simulink model "simulator_prototype_v3_pdg"  (R2021b)
settings: Solver=VariableStepAuto  StartTime=0.0  StopTime=60  FixedStep=0.0001  RelTol=1e-4
undefined symbols (not defined in the file or in its folder): X, Y, Z
libraries: sm_lib x47, nesl_utility x7, simulink x1
(part 4 of 13)

== matlab function simulator_prototype_v3_pdg/Dynamic Model/Coriolis_vector1 ==
  data: dq1 input; dq2 input; tau_c output; dq3 input; dq4 input; dq5 input; dq6 input; q1 input; q2 input; q3 input; q4 input; q5 input; q6 input
function tau_c = Coriolis_vector(dq1,dq2,dq3,dq4,dq5,dq6,q1,q2,q3,q4,q5,q6)
%#codegen

%    This function was generated by the Symbolic Math Toolbox version 9.0.
%    08-Oct-2021 19:57:53

t2 = conj(q1);
t3 = conj(q2);
t4 = conj(q3);
t5 = conj(q4);
t6 = conj(q5);
t7 = conj(q6);
t8 = cos(q1);
t9 = cos(q2);
t10 = cos(q4);
t11 = cos(q5);
t12 = cos(q6);
t13 = sin(q1);
t14 = sin(q2);
t15 = sin(q4);
t16 = sin(q5);
t17 = sin(q6);
t23 = q1+q2;
t29 = dq1.^2;
t30 = dq2.^2;
t31 = dq3.^2;
t32 = dq4.^2;
t33 = dq5.^2;
t34 = dq6.^2;
t50 = 9.007199254740992e+15;
t18 = cos(t2);
t19 = cos(t3);
t20 = cos(t5);
t21 = cos(t6);
t22 = cos(t7);
t24 = sin(t2);
t25 = sin(t3);
t26 = sin(t5);
t27 = sin(t6);
t28 = sin(t7);
t35 = cos(t23);
t36 = sin(t23);
t37 = t2+t3;
t51 = t11.*3.347317932164228e+33;
t52 = t16.*3.347317932164228e+33;
t56 = t8.*4.990478e-2;
t58 = t13.*4.990478e-2;
t59 = t8.*2.167433e-2;
t60 = t13.*2.167433e-2;
t61 = t10.*t12.*3.315051378778914e+33;
t62 = t8.*t9.*3.641522e-2;
t63 = t10.*t17.*3.315051378778914e+33;
t64 = t12.*t15.*3.315051378778914e+33;
t65 = t10.*t16.*1.990083581481952e+33;
t66 = t11.*t15.*1.990083581481952e+33;
t67 = t8.*t14.*3.641522e-2;
t68 = t9.*t13.*3.641522e-2;
t69 = t15.*t16.*1.990083581481952e+33;
t70 = t13.*t14.*3.641522e-2;
t74 = t13.*t14.*2.462267e-2;
t78 = t11.*t12.*5.575912001630188e+33;
t79 = t10.*t12.*6.099194893302011e+33;
t80 = t11.*t12.*1.025883768304404e+34;
t81 = t11.*t17.*5.575912001630188e+33;
t82 = t10.*t17.*6.099194893302011e+33;
t83 = t11.*t17.*1.025883768304404e+34;
t84 = t12.*t16.*1.025883768304404e+34;
t85 = t16.*t17.*5.575912001630188e+33;
t87 = t15.*t17.*6.099194893302011e+33;
t89 = t8.*t9.*2.462267e-2;
t90 = t8.*t14.*2.462267e-2;
t91 = t9.*t13.*2.462267e-2;
t93 = t15.*t16.*t17.*3.315051378778914e+33;
t105 = t11.*t15.*t17.*3.315051378778914e+33;
t116 = t11.*t12.*t15.*6.099194893302011e+33;
t118 = t12.*t15.*t16.*6.099194893302011e+33;
t127 = t15.*t16.*t17.*-6.099194893302011e+33;
t142 = t10.*7.746286054220548e+49;
t143 = t15.*7.746286054220548e+49;
t144 = t10.*t16.*1.830618490855195e+48;
t145 = t11.*t15.*1.830618490855195e+48;
t150 = t10.*t11.*1.830618490855195e+48;
t153 = t10.*t11.*7.290917220067534e+49;
t154 = t10.*t16.*7.290917220067534e+49;
t155 = t15.*t16.*7.290917220067534e+49;
t158 = t10.*6.997781708721691e+52;
t159 = t15.*6.997781708721691e+52;
t166 = t10.*t11.*t12.*5.84291401185902e+49;
t168 = t10.*t11.*t17.*5.84291401185902e+49;
t170 = t10.*t16.*t17.*5.84291401185902e+49;
t171 = t11.*t15.*t17.*5.84291401185902e+49;
t174 = t10.*t16.*7.183572847808854e+52;
t175 = t11.*t15.*7.183572847808854e+52;
t177 = t15.*t16.*7.183572847808854e+52;
t178 = t10.*t11.*t12.*1.075008113939401e+50;
t179 = t10.*t11.*t17.*1.075008113939401e+50;
t180 = t10.*t12.*t16.*1.075008113939401e+50;
t181 = t11.*t12.*t15.*1.075008113939401e+50;
t183 = (q3.*t50)./9.007199254740992e+15;
t184 = t10.*t12.*1.196628789628727e+53;
t185 = t10.*t17.*1.196628789628727e+53;
t186 = t12.*t15.*1.196628789628727e+53;
t187 = (t4.*t50)./9.007199254740992e+15;
t191 = t10.*t12.*2.201616617347892e+53;
t192 = t10.*t17.*2.201616617347892e+53;
t193 = q3.*t50.*2.220446049250313e-16i;
t194 = t15.*t17.*2.201616617347892e+53;
t199 = t4.*t50.*2.220446049250313e-16i;
t206 = q3.*t50.*1.110223024625157e-16i;
t210 = t11.*t15.*t17.*1.196628789628727e+53;
t212 = t15.*t16.*t17.*1.196628789628727e+53;
t214 = t4.*t50.*1.110223024625157e-16i;
t219 = t11.*t12.*t15.*2.201616617347892e+53;
t221 = t12.*t15.*t16.*2.201616617347892e+53;
t232 = t10.*t11.*t50.*4.323455642275676e+17i;
t233 = t10.*t16.*t50.*4.323455642275676e+17i;
t234 = t15.*t16.*t50.*4.323455642275676e+17i;
t242 = t15.*t16.*t17.*-2.201616617347892e+53;
t247 = t10.*t12.*t50.*7.201947557068188e+17i;
t248 = t10.*t17.*t50.*1.325049802940888e+18i;
t249 = t12.*t15.*t50.*1.325049802940888e+18i;
t251 = t12.*t15.*t50.*7.201947557068188e+17i;
t253 = t15.*t17.*t50.*1.325049802940888e+18i;
t254 = t15.*t17.*t50.*7.201947557068188e+17i;
t278 = t10.*t11.*t12.*t50.*1.325049802940888e+18i;
t282 = t10.*t12.*t16.*t50.*1.325049802940888e+18i;
t284 = t10.*t11.*t17.*t50.*7.201947557068188e+17i;
t289 = t10.*t16.*t17.*t50.*7.201947557068188e+17i;
t297 = t10.*t16.*t17.*t50.*-1.325049802940888e+18i;
t298 = t12.*t15.*t16.*t50.*-1.325049802940888e+18i;
t299 = t15.*t16.*t17.*t50.*-7.201947557068188e+17i;
t353 = t11.*t50.*1.746965228796509e+32i;
t355 = t16.*t50.*1.746965228796509e+32i;
t375 = t10.*t50.*4.394953650240249e+33i;
t377 = t15.*t50.*4.394953650240249e+33i;
t379 = t11.*t15.*t50.*1.03862462117543e+32i;
t383 = t15.*t16.*t50.*1.03862462117543e+32i;
t385 = t11.*t50.*6.957746211523004e+33i;
t386 = t16.*t50.*6.957746211523004e+33i;
t390 = t10.*t11.*t50.*1.03862462117543e+32i;
t394 = t10.*t16.*t50.*4.136594366080324e+33i;
t395 = t11.*t15.*t50.*4.136594366080324e+33i;
t396 = t15.*t16.*t50.*4.136594366080324e+33i;
t399 = t10.*t50.*3.97028021545552e+36i;
t400 = t15.*t50.*3.97028021545552e+36i;
t401 = t11.*t12.*t50.*1.025883768304404e+34i;
t402 = t11.*t17.*t50.*5.575912001630188e+33i;
t403 = t12.*t16.*t50.*5.575912001630188e+33i;
t404 = t12.*t16.*t50.*1.025883768304404e+34i;
t406 = t16.*t17.*t50.*5.575912001630188e+33i;
t409 = t16.*t17.*t50.*1.025883768304404e+34i;
t415 = t10.*t11.*t17.*t50.*3.315051378778914e+33i;
t416 = t11.*t12.*t15.*t50.*3.315051378778914e+33i;
t417 = t11.*t15.*t17.*t50.*3.315051378778914e+33i;
t418 = t15.*t16.*t17.*t50.*3.315051378778914e+33i;
t433 = t10.*t11.*t50.*4.075691174875038e+36i;
t435 = t10.*t16.*t50.*4.075691174875038e+36i;
t436 = t15.*t16.*t50.*4.075691174875038e+36i;
t440 = t10.*t11.*t12.*t50.*6.099194893302011e+33i;
t443 = t11.*t12.*t15.*t50.*6.099194893302011e+33i;
t446 = t11.*t15.*t17.*t50.*6.099194893302011e+33i;
t447 = t12.*t15.*t16.*t50.*6.099194893302011e+33i;
t448 = t10.*t12.*t50.*6.789225223739216e+36i;
t449 = t10.*t17.*t50.*1.249115114148252e+37i;
t450 = t12.*t15.*t50.*1.249115114148252e+37i;
t451 = t12.*t15.*t50.*6.789225223739216e+36i;
t453 = t15.*t17.*t50.*1.249115114148252e+37i;
t454 = t15.*t17.*t50.*6.789225223739216e+36i;
t472 = t10.*t11.*t12.*t50.*1.249115114148252e+37i;
t476 = t10.*t12.*t16.*t50.*1.249115114148252e+37i;
t477 = t10.*t11.*t17.*t50.*6.789225223739216e+36i;
t483 = t10.*t16.*t17.*t50.*6.789225223739216e+36i;
t494 = t10.*t16.*t17.*t50.*-1.249115114148252e+37i;
t495 = t12.*t15.*t16.*t50.*-1.249115114148252e+37i;
t496 = t15.*t16.*t17.*t50.*-6.789225223739216e+36i;
t583 = t8.*t9.*3.15365435562893e-2;
t584 = t8.*t14.*3.15365435562893e-2;
t585 = t9.*t13.*3.15365435562893e-2;
t586 = t8.*t9.*2.561099610858757e-2;
t588 = t13.*t14.*3.15365435562893e-2;
t589 = t8.*t14.*2.561099610858757e-2;
t590 = t9.*t13.*2.561099610858757e-2;
t592 = t13.*t14.*2.561099610858757e-2;
t597 = t8.*t9.*1.57299335562893e-2;
t600 = t8.*t14.*1.57299335562893e-2;
t601 = t9.*t13.*1.57299335562893e-2;
t603 = t13.*t14.*1.57299335562893e-2;
t604 = t8.*t9.*4.804434610858757e-2;
t605 = t8.*t14.*4.804434610858757e-2;
t606 = t9.*t13.*4.804434610858757e-2;
t607 = t13.*t14.*4.804434610858757e-2;
t626 = t8.*t9.*1.919581841189621e-2;
t628 = t8.*t9.*4.735389991350965e-2;
t632 = t8.*t14.*1.919581841189621e-2;
t633 = t9.*t13.*1.919581841189621e-2;
t635 = t8.*t14.*4.735389991350965e-2;
t636 = t9.*t13.*4.735389991350965e-2;
t638 = t13.*t14.*1.919581841189621e-2;
t639 = t13.*t14.*4.735389991350965e-2;
t640 = t8.*t9.*2.273122991350965e-2;
t641 = t8.*t9.*3.603517512464e-2;
t642 = t8.*t14.*2.273122991350965e-2;
t643 = t9.*t13.*2.273122991350965e-2;
t645 = t8.*t14.*3.603517512464e-2;
t646 = t9.*t13.*3.603517512464e-2;
t647 = t13.*t14.*2.273122991350965e-2;
t649 = t13.*t14.*3.603517512464e-2;
t653 = t8.*t9.*1.141250512464e-2;
t654 = t8.*t14.*1.141250512464e-2;
t655 = t9.*t13.*1.141250512464e-2;
t656 = t13.*t14.*1.141250512464e-2;
t661 = t8.*t9.*5.561103841189621e-2;
t663 = t8.*t14.*5.561103841189621e-2;
t664 = t9.*t13.*5.561103841189621e-2;
t666 = t13.*t14.*5.561103841189621e-2;
t667 = t8.*t9.*3.823389842399381e-2;
t668 = t8.*t14.*3.823389842399381e-2;
t669 = t9.*t13.*3.823389842399381e-2;
t671 = t8.*t9.*7.464911842399381e-2;
t674 = t13.*t14.*3.823389842399381e-2;
t675 = t8.*t14.*7.464911842399381e-2;
t676 = t9.*t13.*7.464911842399381e-2;
t679 = t13.*t14.*7.464911842399381e-2;
t703 = t8.*t9.*t10.*t16.*2.498039274760989e-3;
t704 = t8.*t10.*t11.*t14.*2.498039274760989e-3;
t705 = t9.*t10.*t11.*t13.*2.498039274760989e-3;
t706 = t8.*t9.*t15.*t16.*2.498039274760989e-3;
t707 = t8.*t10.*t14.*t16.*2.498039274760989e-3;
t708 = t9.*t10.*t13.*t16.*2.498039274760989e-3;
t709 = t10.*t11.*t13.*t14.*2.498039274760989e-3;
t711 = t8.*t9.*t10.*t11.*5.478347731418506e-3;
t712 = t8.*t14.*t15.*t16.*2.498039274760989e-3;
t713 = t9.*t13.*t15.*t16.*2.498039274760989e-3;
t714 = t10.*t13.*t14.*t16.*2.498039274760989e-3;
t719 = t8.*t9.*t10.*t16.*5.478347731418506e-3;
t720 = t8.*t9.*t11.*t15.*5.478347731418506e-3;
t721 = t8.*t10.*t11.*t14.*5.478347731418506e-3;
t722 = t9.*t10.*t11.*t13.*5.478347731418506e-3;
t723 = t13.*t14.*t15.*t16.*2.498039274760989e-3;
t726 = t8.*t10.*t14.*t16.*5.478347731418506e-3;
t727 = t8.*t11.*t14.*t15.*5.478347731418506e-3;
t728 = t9.*t10.*t13.*t16.*5.478347731418506e-3;
t729 = t9.*t11.*t13.*t15.*5.478347731418506e-3;
t730 = t10.*t11.*t13.*t14.*5.478347731418506e-3;
t731 = t10.*t13.*t14.*t16.*5.478347731418506e-3;
t732 = t11.*t13.*t14.*t15.*5.478347731418506e-3;
t742 = t8.*t9.*t10.*t11.*2.498039274760989e-3;
t748 = t8.*t9.*t10.*t11.*4.201698731382561e-3;
t749 = t8.*t9.*t10.*t16.*4.201698731382561e-3;
t750 = t8.*t10.*t11.*t14.*4.201698731382561e-3;
t751 = t9.*t10.*t11.*t13.*4.201698731382561e-3;
t752 = t8.*t9.*t15.*t16.*4.201698731382561e-3;
t753 = t8.*t10.*t14.*t16.*4.201698731382561e-3;
t754 = t9.*t10.*t13.*t16.*4.201698731382561e-3;
t755 = t10.*t11.*t13.*t14.*4.201698731382561e-3;
t760 = t8.*t14.*t15.*t16.*4.201698731382561e-3;
t761 = t9.*t13.*t15.*t16.*4.201698731382561e-3;
t762 = t10.*t13.*t14.*t16.*4.201698731382561e-3;
t766 = t13.*t14.*t15.*t16.*4.201698731382561e-3;
t768 = t8.*t9.*t10.*t11.*9.214573584066668e-3;
t769 = t8.*t9.*t10.*t16.*9.214573584066668e-3;
t770 = t8.*t9.*t11.*t15.*9.214573584066668e-3;
t771 = t8.*t10.*t11.*t14.*9.214573584066668e-3;
t772 = t9.*t10.*t11.*t13.*9.214573584066668e-3;
t773 = t8.*t10.*t14.*t16.*9.214573584066668e-3;
t774 = t8.*t11.*t14.*t15.*9.214573584066668e-3;
t775 = t9.*t10.*t13.*t16.*9.214573584066668e-3;
t776 = t9.*t11.*t13.*t15.*9.214573584066668e-3;
t777 = t10.*t11.*t13.*t14.*9.214573584066668e-3;
t778 = t10.*t13.*t14.*t16.*9.214573584066668e-3;
t779 = t11.*t13.*t14.*t15.*9.214573584066668e-3;
t780 = t13.*t14.*t15.*2.842045365580232e-6;
t788 = t8.*t9.*t10.*2.538961213904336e-3;
t789 = t8.*t9.*t15.*2.538961213904336e-3;
t790 = t8.*t10.*t14.*2.538961213904336e-3;
t791 = t9.*t10.*t13.*2.538961213904336e-3;
t792 = t8.*t14.*t15.*2.538961213904336e-3;
t793 = t9.*t13.*t15.*2.538961213904336e-3;
t794 = t10.*t13.*t14.*2.538961213904336e-3;
t795 = t13.*t14.*t15.*2.538961213904336e-3;
t798 = t8.*t9.*t10.*2.842045365580232e-6;
t800 = t8.*t9.*t15.*2.842045365580232e-6;
t801 = t8.*t10.*t14.*2.842045365580232e-6;
t802 = t9.*t10.*t13.*2.842045365580232e-6;
t803 = t8.*t14.*t15.*2.842045365580232e-6;
t804 = t9.*t13.*t15.*2.842045365580232e-6;
t805 = t10.*t13.*t14.*2.842045365580232e-6;
t806 = t8.*t14.*t15.*4.780316517734772e-6;
t807 = t9.*t13.*t15.*4.780316517734772e-6;
t808 = t10.*t13.*t14.*4.780316517734772e-6;
t810 = t13.*t14.*t15.*4.780316517734772e-6;
t811 = t8.*t9.*t10.*4.270529378491088e-3;
t813 = t8.*t9.*t15.*4.270529378491088e-3;
t814 = t8.*t10.*t14.*4.270529378491088e-3;
t815 = t9.*t10.*t13.*4.270529378491088e-3;
t816 = t8.*t14.*t15.*4.270529378491088e-3;
t817 = t9.*t13.*t15.*4.270529378491088e-3;
t818 = t10.*t13.*t14.*4.270529378491088e-3;
t819 = t13.*t14.*t15.*4.270529378491088e-3;
t821 = t8.*t9.*t10.*4.780316517734772e-6;
t822 = t8.*t9.*t15.*4.780316517734772e-6;
t823 = t8.*t10.*t14.*4.780316517734772e-6;
t824 = t9.*t10.*t13.*4.780316517734772e-6;
t38 = cos(t37);
t39 = sin(t37);
t40 = t36.*7.742227997977903e+15;
t41 = t35.*4.602992943936994e+15;
t42 = t36.*4.602992943936994e+15;
t43 = t35.*7.742227997977903e+15;
t53 = t21.*3.347317932164228e+33;
t54 = t27.*3.347317932164228e+33;
t55 = t35.*1.580661e-2;
t57 = t36.*1.580661e-2;
t73 = -t60;
t75 = -t61;
t76 = -t62;
t77 = -t66;
t86 = t35.*2.243335e-2;
t88 = t36.*2.243335e-2;
t92 = -t74;
t94 = -t83;
t96 = -t87;
t98 = t20.*t22.*3.315051378778914e+33;
t99 = t20.*t28.*3.315051378778914e+33;
t100 = t22.*t26.*3.315051378778914e+33;
t101 = t20.*t27.*1.990083581481952e+33;
t102 = t21.*t26.*1.990083581481952e+33;
t103 = t26.*t27.*1.990083581481952e+33;
t104 = t16.*t63;
t106 = t16.*t64;
t107 = t21.*t22.*5.575912001630188e+33;
t108 = t20.*t22.*6.099194893302011e+33;
t109 = t21.*t22.*1.025883768304404e+34;
t110 = t21.*t28.*5.575912001630188e+33;
t111 = t20.*t28.*6.099194893302011e+33;
t112 = t21.*t28.*1.025883768304404e+34;
t113 = t22.*t27.*1.025883768304404e+34;
t114 = t27.*t28.*5.575912001630188e+33;
t115 = t16.*t79;
t117 = t26.*t28.*6.099194893302011e+33;
t119 = t16.*t87;
t122 = -t105;
t125 = -t116;
t129 = t21.*t26.*t28.*3.315051378778914e+33;
t132 = t26.*t27.*t28.*3.315051378778914e+33;
t135 = t21.*t22.*t26.*6.099194893302011e+33;
t136 = t22.*t26.*t27.*6.099194893302011e+33;
t139 = t26.*t27.*t28.*-6.099194893302011e+33;
t146 = t20.*7.746286054220548e+49;
t147 = t26.*7.746286054220548e+49;
t148 = -t142;
t149 = -t143;
t156 = -t154;
t157 = -t155;
t160 = t20.*t21.*1.830618490855195e+48;
t161 = t20.*t27.*1.830618490855195e+48;
t162 = t21.*t26.*1.830618490855195e+48;
t163 = t20.*t27.*7.290917220067534e+49;
t164 = t26.*t27.*7.290917220067534e+49;
t165 = -t159;
t167 = t20.*6.997781708721691e+52;
t169 = t26.*6.997781708721691e+52;
t172 = t20.*t21.*7.290917220067534e+49;
t188 = cos(t183);
t189 = sin(t183);
t190 = -t179;
t195 = t20.*t21.*t28.*5.84291401185902e+49;
t196 = t20.*t27.*t28.*5.84291401185902e+49;
t197 = t21.*t26.*t28.*5.84291401185902e+49;
t198 = -t184;
t200 = exp(t193);
t201 = cos(t187);
t202 = sin(t187);
t203 = t20.*t27.*7.183572847808854e+52;
t204 = t21.*t26.*7.183572847808854e+52;
t205 = t26.*t27.*7.183572847808854e+52;
t207 = -t194;
t208 = t20.*t21.*t22.*5.84291401185902e+49;
t209 = t16.*t185;
t211 = t16.*t186;
t213 = -t199;
t215 = exp(t206);
t216 = t20.*t22.*2.201616617347892e+53;
t217 = t20.*t28.*2.201616617347892e+53;
t218 = t16.*t191;
t220 = t26.*t28.*2.201616617347892e+53;
t222 = t16.*t194;
t223 = t20.*t21.*t22.*1.075008113939401e+50;
t224 = t20.*t22.*1.196628789628727e+53;
t225 = t20.*t21.*t28.*1.075008113939401e+50;
t226 = t20.*t22.*t27.*1.075008113939401e+50;
t227 = t21.*t22.*t26.*1.075008113939401e+50;
t228 = -t206;
t230 = t20.*t28.*1.196628789628727e+53;
t231 = t22.*t26.*1.196628789628727e+53;
t235 = -t214;
t241 = exp(t214);
t245 = -t232;
t246 = -t234;
t255 = t20.*t27.*t50.*4.323455642275676e+17i;
t257 = t26.*t27.*t50.*4.323455642275676e+17i;
t260 = t21.*t26.*t28.*1.196628789628727e+53;
t263 = t26.*t27.*t28.*1.196628789628727e+53;
t266 = -t248;
t267 = -t249;
t269 = -t253;
t270 = -t254;
t272 = t21.*t22.*t26.*2.201616617347892e+53;
t273 = t20.*t21.*t50.*4.323455642275676e+17i;
t274 = t22.*t26.*t27.*2.201616617347892e+53;
t276 = t26.*t27.*t28.*-2.201616617347892e+53;
t277 = t20.*t22.*t50.*7.201947557068188e+17i;
t279 = t20.*t28.*t50.*1.325049802940888e+18i;
t280 = t22.*t26.*t50.*1.325049802940888e+18i;
t281 = t22.*t26.*t50.*7.201947557068188e+17i;
t283 = t26.*t28.*t50.*1.325049802940888e+18i;
t285 = t16.*t247;
t286 = t26.*t28.*t50.*7.201947557068188e+17i;
t287 = t16.*t248;
t288 = t16.*t249;
t290 = t16.*t254;
t294 = -t278;
t296 = -t284;
t301 = t20.*t21.*t22.*t50.*1.325049802940888e+18i;
t302 = t20.*t22.*t27.*t50.*1.325049802940888e+18i;
t303 = t20.*t21.*t28.*t50.*7.201947557068188e+17i;
t307 = t20.*t27.*t28.*t50.*7.201947557068188e+17i;
t310 = t20.*t22.*t27.*t50.*-7.201947557068188e+17i;
t312 = t18.*7.234522890390001e-5;
t313 = t24.*7.234522890390001e-5;
t314 = t18.*1.665736718274e-4;
t315 = t18.*4.418500737171001e-4;
t316 = t24.*1.665736718274e-4;
t317 = t24.*4.418500737171001e-4;
t318 = t18.*1.0173523574586e-3;
t320 = t24.*1.0173523574586e-3;
t321 = t18.*1.4420704809832e-3;
t322 = t24.*1.4420704809832e-3;
t326 = t18.*5.42809301582e-4;
t327 = t24.*2.35749519977e-4;
t328 = t24.*5.42809301582e-4;
t329 = t18.*3.62675502933e-4;
t330 = t18.*6.263109763852e-4;
t331 = t24.*3.62675502933e-4;
t332 = t24.*6.263109763852e-4;
t333 = t18.*1.575149421255e-4;
t334 = t24.*1.575149421255e-4;
t338 = t18.*2.35749519977e-4;
t357 = t18.*t19.*2.64642149067e-4;
t358 = t18.*t25.*2.64642149067e-4;
t359 = t19.*t24.*2.64642149067e-4;
t360 = t24.*t25.*2.64642149067e-4;
t364 = t18.*t25.*1.789415608245e-4;
t365 = t19.*t24.*1.789415608245e-4;
t367 = t24.*t25.*1.789415608245e-4;
t368 = -t353;
t373 = t21.*t50.*1.746965228796509e+32i;
t376 = t27.*t50.*1.746965228796509e+32i;
t378 = t18.*t19.*1.789415608245e-4;
t381 = t20.*t50.*4.394953650240249e+33i;
t384 = t26.*t50.*4.394953650240249e+33i;
t388 = -t375;
t391 = -t379;
t392 = -t383;
t397 = t21.*t50.*6.957746211523004e+33i;
t398 = t27.*t50.*6.957746211523004e+33i;
t405 = t20.*t21.*t50.*1.03862462117543e+32i;
t407 = -t394;
t408 = -t395;
t411 = t21.*t26.*t50.*1.03862462117543e+32i;
t412 = t26.*t27.*t50.*1.03862462117543e+32i;
t419 = -t399;
t420 = -t400;
t421 = t20.*t27.*t50.*4.136594366080324e+33i;
t422 = t21.*t26.*t50.*4.136594366080324e+33i;
t423 = t26.*t27.*t50.*4.136594366080324e+33i;
t424 = -t401;
t425 = -t402;
t427 = -t409;
t428 = t20.*t50.*3.97028021545552e+36i;
t430 = t26.*t50.*3.97028021545552e+36i;
t431 = -t416;
t432 = -t417;
t434 = -t418;
t437 = t21.*t22.*t50.*1.025883768304404e+34i;
t438 = t21.*t28.*t50.*5.575912001630188e+33i;
t439 = t22.*t27.*t50.*5.575912001630188e+33i;
t441 = t22.*t27.*t50.*1.025883768304404e+34i;
t442 = t27.*t28.*t50.*5.575912001630188e+33i;
t444 = t27.*t28.*t50.*1.025883768304404e+34i;
t452 = -t436;
t457 = -t443;
t459 = -t447;
t460 = t20.*t27.*t50.*4.075691174875038e+36i;
t461 = t26.*t27.*t50.*4.075691174875038e+36i;
t462 = t20.*t21.*t28.*t50.*3.315051378778914e+33i;
t463 = t21.*t22.*t26.*t50.*3.315051378778914e+33i;
t464 = -t449;
t465 = -t450;
t466 = t21.*t26.*t28.*t50.*3.315051378778914e+33i;
t467 = -t453;
t468 = -t454;
t469 = t26.*t27.*t28.*t50.*3.315051378778914e+33i;
t470 = t20.*t21.*t50.*4.075691174875038e+36i;
t473 = t20.*t28.*t50.*1.249115114148252e+37i;
t474 = t22.*t26.*t50.*1.249115114148252e+37i;
tau_c = ft_1({dq1,dq2,dq3,dq4,dq5,dq6,t10,t100,t101,t102,t103,t104,t105,t106,t107,t108,t109,t11,t110,t111,t112,t113,t114,t115,t116,t117,t118,t119,t12,t122,t125,t127,t129,t13,t132,t135,t136,t139,t14,t142,t143,t144,t145,t146,t147,t148,t149,t15,t150,t153,t154,t155,t156,t157,t158,t159,t16,t160,t161,t162,t163,t164,t165,t166,t167,t168,t169,t17,t170,t171,t172,t174,t175,t177,t178,t179,t18,t180,t181,t184,t185,t186,t188,t189,t19,t190,t191,t192,t194,t195,t196,t197,t198,t20,t200,t201,t202,t203,t204,t205,t207,t208,t209,t21,t210,t211,t212,t213,t215,t216,t217,t218,t219,t22,t220,t221,t222,t223,t224,t225,t226,t227,t230,t231,t232,t233,t234,t235,t24,t241,t242,t245,t246,t247,t248,t249,t25,t251,t253,t254,t255,t257,t26,t260,t263,t266,t267,t269,t27,t270,t272,t273,t274,t276,t277,t278,t279,t28,t280,t281,t282,t283,t284,t285,t286,t287,t288,t289,t29,t290,t294,t296,t297,t298,t299,t30,t301,t302,t303,t307,t31,t310,t312,t313,t314,t315,t316,t317,t318,t32,t320,t321,t322,t326,t327,t328,t329,t33,t330,t331,t332,t333,t334,t338,t34,t35,t353,t355,t357,t358,t359,t36,t360,t364,t365,t367,t368,t373,t375,t376,t377,t378,t379,t38,t381,t383,t384,t385,t386,t388,t39,t390,t391,t392,t394,t395,t396,t397,t398,t399,t40,t400,t401,t402,t403,t404,t405,t406,t407,t408,t409,t41,t411,t412,t415,t416,t417,t418,t419,t42,t420,t421,t422,t423,t424,t425,t427,t428,t43,t430,t431,t432,t433,t434,t435,t436,t437,t438,t439,t440,t441,t442,t443,t444,t446,t447,t448,t449,t450,t451,t452,t453,t454,t457,t459,t460,t461,t462,t463,t464,t465,t466,t467,t468,t469,t470,t472,t473,t474,t476,t477,t483,t494,t495,t496,t50,t51,t52,t53,t54,t55,t56,t57,t58,t583,t584,t585,t586,t588,t589,t59,t590,t592,t597,t60,t600,t601,t603,t604,t605,t606,t607,t61,t626,t628,t63,t632,t633,t635,t636,t638,t639,t64,t640,t641,t642,t643,t645,t646,t647,t649,t65,t653,t654,t655,t656,t66,t661,t663,t664,t666,t667,t668,t669,t67,t671,t674,t675,t676,t679,t68,t69,t70,t703,t704,t705,t706,t707,t708,t709,t711,t712,t713,t714,t719,t720,t721,t722,t723,t726,t727,t728,t729,t73,t730,t731,t732,t742,t748,t749,t75,t750,t751,t752,t753,t754,t755,t76,t760,t761,t762,t766,t768,t769,t77,t770,t771,t772,t773,t774,t775,t776,t777,t778,t779,t78,t780,t788,t789,t79,t790,t791,t792,t793,t794,t795,t798,t8,t80,t800,t801,t802,t803,t804,t805,t806,t807,t808,t81,t810,t811,t813,t814,t815,t816,t817,t818,t819,t82,t821,t822,t823,t824,t83,t84,t85,t86,t87,t88,t89,t9,t90,t91,t92,t93,t94,t96,t98,t99});
end
function tau_c = ft_1(ct)
dq1 = ct{1};
dq2 = ct{2};
dq3 = ct{3};
dq4 = ct{4};
dq5 = ct{5};
dq6 = ct{6};
t10 = ct{7};
t100 = ct{8};
t101 = ct{9};
t102 = ct{10};
t103 = ct{11};
t104 = ct{12};
t105 = ct{13};
t106 = ct{14};
t107 = ct{15};
t108 = ct{16};
t109 = ct{17};
t11 = ct{18};
t110 = ct{19};
t111 = ct{20};
t112 = ct{21};
t113 = ct{22};
t114 = ct{23};
t115 = ct{24};
t116 = ct{25};
t117 = ct{26};
t118 = ct{27};
t119 = ct{28};
t12 = ct{29};
t122 = ct{30};
t125 = ct{31};
t127 = ct{32};
t129 = ct{33};
t13 = ct{34};
t132 = ct{35};
t135 = ct{36};
t136 = ct{37};
t139 = ct{38};
t14 = ct{39};
t142 = ct{40};
t143 = ct{41};
t144 = ct{42};
t145 = ct{43};
t146 = ct{44};
t147 = ct{45};
t148 = ct{46};
t149 = ct{47};
t15 = ct{48};
t150 = ct{49};
t153 = ct{50};
t154 = ct{51};
t155 = ct{52};
t156 = ct{53};
t157 = ct{54};
t158 = ct{55};
t159 = ct{56};
t16 = ct{57};
t160 = ct{58};
t161 = ct{59};
t162 = ct{60};
t163 = ct{61};
t164 = ct{62};
t165 = ct{63};
t166 = ct{64};
t167 = ct{65};
t168 = ct{66};
t169 = ct{67};
t17 = ct{68};
t170 = ct{69};
t171 = ct{70};
t172 = ct{71};
t174 = ct{72};
t175 = ct{73};
t177 = ct{74};
t178 = ct{75};
t179 = ct{76};
t18 = ct{77};
t180 = ct{78};
t181 = ct{79};
t184 = ct{80};
t185 = ct{81};
t186 = ct{82};
t188 = ct{83};
t189 = ct{84};
t19 = ct{85};
t190 = ct{86};
t191 = ct{87};
t192 = ct{88};
t194 = ct{89};
t195 = ct{90};
t196 = ct{91};
t197 = ct{92};
t198 = ct{93};
t20 = ct{94};
t200 = ct{95};
t201 = ct{96};
t202 = ct{97};
t203 = ct{98};
t204 = ct{99};
t205 = ct{100};
t207 = ct{101};
t208 = ct{102};
t209 = ct{103};
t21 = ct{104};
t210 = ct{105};
t211 = ct{106};
t212 = ct{107};
t213 = ct{108};
t215 = ct{109};
t216 = ct{110};
t217 = ct{111};
t218 = ct{112};
t219 = ct{113};
t22 = ct{114};
t220 = ct{115};
t221 = ct{116};
t222 = ct{117};
t223 = ct{118};
t224 = ct{119};
t225 = ct{120};
t226 = ct{121};
t227 = ct{122};
t230 = ct{123};
t231 = ct{124};
t232 = ct{125};
t233 = ct{126};
t234 = ct{127};
t235 = ct{128};
t24 = ct{129};
t241 = ct{130};
t242 = ct{131};
t245 = ct{132};
t246 = ct{133};
t247 = ct{134};
t248 = ct{135};
t249 = ct{136};
t25 = ct{137};
t251 = ct{138};
t253 = ct{139};
t254 = ct{140};
t255 = ct{141};
t257 = ct{142};
t26 = ct{143};
t260 = ct{144};
t263 = ct{145};
t266 = ct{146};
t267 = ct{147};
t269 = ct{148};
t27 = ct{149};
t270 = ct{150};
t272 = ct{151};
t273 = ct{152};
t274 = ct{153};
t276 = ct{154};
t277 = ct{155};
t278 = ct{156};
t279 = ct{157};
t28 = ct{158};
t280 = ct{159};
t281 = ct{160};
t282 = ct{161};
t283 = ct{162};
t284 = ct{163};
t285 = ct{164};
t286 = ct{165};
t287 = ct{166};
t288 = ct{167};
t289 = ct{168};
t29 = ct{169};
t290 = ct{170};
t294 = ct{171};
t296 = ct{172};
t297 = ct{173};
t298 = ct{174};
t299 = ct{175};
t30 = ct{176};
t301 = ct{177};
t302 = ct{178};
t303 = ct{179};
t307 = ct{180};
t31 = ct{181};
t310 = ct{182};
t312 = ct{183};
t313 = ct{184};
t314 = ct{185};
t315 = ct{186};
t316 = ct{187};
t317 = ct{188};
t318 = ct{189};
t32 = ct{190};
t320 = ct{191};
t321 = ct{192};
t322 = ct{193};
t326 = ct{194};
t327 = ct{195};
t328 = ct{196};
t329 = ct{197};
t33 = ct{198};
t330 = ct{199};
t331 = ct{200};
t332 = ct{201};
t333 = ct{202};
t334 = ct{203};
t338 = ct{204};
t34 = ct{205};
t35 = ct{206};
t353 = ct{207};
t355 = ct{208};
t357 = ct{209};
t358 = ct{210};
t359 = ct{211};
t36 = ct{212};
t360 = ct{213};
t364 = ct{214};
t365 = ct{215};
t367 = ct{216};
t368 = ct{217};
t373 = ct{218};
t375 = ct{219};
t376 = ct{220};
t377 = ct{221};
t378 = ct{222};
t379 = ct{223};
t38 = ct{224};
t381 = ct{225};
t383 = ct{226};
t384 = ct{227};
t385 = ct{228};
t386 = ct{229};
t388 = ct{230};
t39 = ct{231};
t390 = ct{232};
t391 = ct{233};
t392 = ct{234};
t394 = ct{235};
t395 = ct{236};
t396 = ct{237};
t397 = ct{238};
t398 = ct{239};
t399 = ct{240};
t40 = ct{241};
t400 = ct{242};
t401 = ct{243};
t402 = ct{244};
t403 = ct{245};
t404 = ct{246};
t405 = ct{247};
t406 = ct{248};
t407 = ct{249};
t408 = ct{250};
t409 = ct{251};
t41 = ct{252};
t411 = ct{253};
t412 = ct{254};
t415 = ct{255};
t416 = ct{256};
t417 = ct{257};
t418 = ct{258};
t419 = ct{259};
t42 = ct{260};
t420 = ct{261};
t421 = ct{262};
t422 = ct{263};
t423 = ct{264};
t424 = ct{265};
t425 = ct{266};
t427 = ct{267};
t428 = ct{268};
t43 = ct{269};
t430 = ct{270};
t431 = ct{271};
t432 = ct{272};
t433 = ct{273};
t434 = ct{274};
t435 = ct{275};
t436 = ct{276};
t437 = ct{277};
t438 = ct{278};
t439 = ct{279};
t440 = ct{280};
t441 = ct{281};
t442 = ct{282};
t443 = ct{283};
t444 = ct{284};
t446 = ct{285};
t447 = ct{286};
t448 = ct{287};
t449 = ct{288};
t450 = ct{289};
t451 = ct{290};
t452 = ct{291};
t453 = ct{292};
t454 = ct{293};
t457 = ct{294};
t459 = ct{295};
t460 = ct{296};
t461 = ct{297};
t462 = ct{298};
t463 = ct{299};
t464 = ct{300};
t465 = ct{301};
t466 = ct{302};
t467 = ct{303};
t468 = ct{304};
t469 = ct{305};
t470 = ct{306};
t472 = ct{307};
t473 = ct{308};
t474 = ct{309};
t476 = ct{310};
t477 = ct{311};
t483 = ct{312};
t494 = ct{313};
t495 = ct{314};
t496 = ct{315};
t50 = ct{316};
t51 = ct{317};
t52 = ct{318};
t53 = ct{319};
t54 = ct{320};
t55 = ct{321};
t56 = ct{322};
t57 = ct{323};
t58 = ct{324};
t583 = ct{325};
t584 = ct{326};
t585 = ct{327};
t586 = ct{328};
t588 = ct{329};
t589 = ct{330};
t59 = ct{331};
t590 = ct{332};
t592 = ct{333};
t597 = ct{334};
t60 = ct{335};
t600 = ct{336};
t601 = ct{337};
t603 = ct{338};
t604 = ct{339};
t605 = ct{340};
t606 = ct{341};
t607 = ct{342};
t61 = ct{343};
t626 = ct{344};
t628 = ct{345};
t63 = ct{346};
t632 = ct{347};
t633 = ct{348};
t635 = ct{349};
t636 = ct{350};
t638 = ct{351};
t639 = ct{352};
t64 = ct{353};
t640 = ct{354};
t641 = ct{355};
t642 = ct{356};
t643 = ct{357};
t645 = ct{358};
t646 = ct{359};
t647 = ct{360};
t649 = ct{361};
t65 = ct{362};
t653 = ct{363};
t654 = ct{364};
t655 = ct{365};
t656 = ct{366};
t66 = ct{367};
t661 = ct{368};
t663 = ct{369};
t664 = ct{370};
t666 = ct{371};
t667 = ct{372};
t668 = ct{373};
t669 = ct{374};
t67 = ct{375};
t671 = ct{376};
t674 = ct{377};
t675 = ct{378};
t676 = ct{379};
t679 = ct{380};
t68 = ct{381};
t69 = ct{382};
t70 = ct{383};
t703 = ct{384};
t704 = ct{385};
t705 = ct{386};
t706 = ct{387};
t707 = ct{388};
t708 = ct{389};
t709 = ct{390};
t711 = ct{391};
t712 = ct{392};
t713 = ct{393};
t714 = ct{394};
t719 = ct{395};
t720 = ct{396};
t721 = ct{397};
t722 = ct{398};
t723 = ct{399};
t726 = ct{400};
t727 = ct{401};
t728 = ct{402};
t729 = ct{403};
t73 = ct{404};
t730 = ct{405};
t731 = ct{406};
t732 = ct{407};
t742 = ct{408};
t748 = ct{409};
t749 = ct{410};
t75 = ct{411};
t750 = ct{412};
t751 = ct{413};
t752 = ct{414};
t753 = ct{415};
t754 = ct{416};
t755 = ct{417};
t76 = ct{418};
t760 = ct{419};
t761 = ct{420};
t762 = ct{421};
t766 = ct{422};
t768 = ct{423};
t769 = ct{424};
t77 = ct{425};
t770 = ct{426};
t771 = ct{427};
t772 = ct{428};
t773 = ct{429};
t774 = ct{430};
t775 = ct{431};
t776 = ct{432};
t777 = ct{433};
t778 = ct{434};
t779 = ct{435};
t78 = ct{436};
t780 = ct{437};
t788 = ct{438};
t789 = ct{439};
t79 = ct{440};
t790 = ct{441};
t791 = ct{442};
t792 = ct{443};
t793 = ct{444};
t794 = ct{445};
t795 = ct{446};
t798 = ct{447};
t8 = ct{448};
t80 = ct{449};
t800 = ct{450};
t801 = ct{451};
t802 = ct{452};
t803 = ct{453};
t804 = ct{454};
t805 = ct{455};
t806 = ct{456};
t807 = ct{457};
t808 = ct{458};
t81 = ct{459};
t810 = ct{460};
t811 = ct{461};
t813 = ct{462};
t814 = ct{463};
t815 = ct{464};
t816 = ct{465};
t817 = ct{466};
t818 = ct{467};
t819 = ct{468};
t82 = ct{469};
t821 = ct{470};
t822 = ct{471};
t823 = ct{472};
t824 = ct{473};
t83 = ct{474};
t84 = ct{475};
t85 = ct{476};
t86 = ct{477};
t87 = ct{478};
t88 = ct{479};
t89 = ct{480};
t9 = ct{481};
t90 = ct{482};
t91 = ct{483};
t92 = ct{484};
t93 = ct{485};
t94 = ct{486};
t96 = ct{487};
t98 = ct{488};
t99 = ct{489};
t475 = t22.*t26.*t50.*6.789225223739216e+36i;
t478 = t16.*t448;
t479 = t26.*t28.*t50.*1.249115114148252e+37i;
t480 = t26.*t28.*t50.*6.789225223739216e+36i;
t481 = t16.*t449;
t482 = t16.*t450;
t484 = t16.*t454;
t487 = t20.*t21.*t22.*t50.*6.099194893302011e+33i;
t488 = t21.*t22.*t26.*t50.*6.099194893302011e+33i;
t489 = t21.*t26.*t28.*t50.*6.099194893302011e+33i;
t490 = t22.*t26.*t27.*t50.*6.099194893302011e+33i;
t492 = t20.*t22.*t50.*6.789225223739216e+36i;
t499 = t20.*t21.*t22.*t50.*1.249115114148252e+37i;
t500 = t20.*t22.*t27.*t50.*1.249115114148252e+37i;
t501 = t20.*t21.*t28.*t50.*6.789225223739216e+36i;
t505 = t20.*t27.*t28.*t50.*6.789225223739216e+36i;
t510 = t20.*t22.*t27.*t50.*-6.789225223739216e+36i;
t608 = -t586;
t609 = -t588;
t621 = -t603;
t622 = -t604;
t657 = -t626;
t659 = -t632;
t660 = -t633;
t665 = -t639;
t670 = -t641;
t672 = -t642;
t673 = -t643;
t677 = -t647;
t678 = -t649;
t681 = -t653;
t682 = t18.*t19.*2.273122991350965e-2;
t683 = -t661;
t684 = t18.*t25.*2.273122991350965e-2;
t685 = t19.*t24.*2.273122991350965e-2;
t686 = -t663;
t687 = -t664;
t688 = t24.*t25.*2.273122991350965e-2;
t689 = -t671;
t690 = t18.*t19.*1.141250512464e-2;
t691 = -t674;
t692 = t18.*t25.*1.141250512464e-2;
t693 = t19.*t24.*1.141250512464e-2;
t694 = t24.*t25.*1.141250512464e-2;
t695 = t18.*t19.*1.919581841189621e-2;
t699 = t18.*t25.*1.919581841189621e-2;
t700 = t19.*t24.*1.919581841189621e-2;
t702 = t24.*t25.*1.919581841189621e-2;
t710 = t18.*t19.*3.823389842399381e-2;
t715 = t18.*t25.*3.823389842399381e-2;
t716 = t19.*t24.*3.823389842399381e-2;
t724 = t24.*t25.*3.823389842399381e-2;
t743 = -t703;
t744 = -t706;
t745 = -t707;
t746 = -t708;
t747 = -t709;
t757 = -t727;
t758 = -t729;
t759 = -t730;
t763 = -t731;
t764 = -t732;
t781 = -t748;
t782 = -t752;
t783 = -t753;
t784 = -t754;
t785 = -t760;
t786 = -t761;
t787 = -t762;
t796 = -t768;
t797 = -t769;
t799 = -t779;
t809 = -t780;
t812 = -t788;
t820 = -t795;
t825 = -t803;
t826 = -t804;
t827 = -t805;
t828 = -t810;
t829 = -t811;
t830 = -t813;
t831 = -t814;
t832 = -t815;
t833 = -t821;
t1089 = t24.*t25.*5.250384412218911e-5;
t1101 = t18.*t19.*8.548515114112684e-5;
t1104 = t18.*t25.*8.548515114112684e-5;
t1105 = t19.*t24.*8.548515114112684e-5;
t1108 = t18.*t19.*1.052636211784891e-4;
t1110 = t24.*t25.*8.548515114112684e-5;
t1113 = t18.*t25.*1.052636211784891e-4;
t1114 = t19.*t24.*1.052636211784891e-4;
t1115 = t24.*t25.*1.052636211784891e-4;
t1121 = t18.*t19.*5.250384412218911e-5;
t1123 = t18.*t25.*5.250384412218911e-5;
t1124 = t19.*t24.*5.250384412218911e-5;
t1155 = t18.*t19.*1.603638597716268e-4;
t1158 = t18.*t25.*1.603638597716268e-4;
t1159 = t19.*t24.*1.603638597716268e-4;
t1162 = t24.*t25.*1.603638597716268e-4;
t1190 = t18.*t19.*1.041288275878652e-3;
t1193 = t18.*t25.*1.041288275878652e-3;
t1194 = t19.*t24.*1.041288275878652e-3;
t1196 = t24.*t25.*1.041288275878652e-3;
t1205 = t18.*t19.*5.150636339692531e-4;
t1207 = t18.*t25.*5.150636339692531e-4;
t1208 = t19.*t24.*5.150636339692531e-4;
t1210 = t24.*t25.*5.150636339692531e-4;
t1215 = t18.*t19.*8.119509961859382e-4;
t1216 = t18.*t19.*1.606961034807054e-3;
t1217 = t18.*t25.*8.119509961859382e-4;
t1218 = t19.*t24.*8.119509961859382e-4;
t1219 = t18.*t25.*1.606961034807054e-3;
t1220 = t19.*t24.*1.606961034807054e-3;
t1221 = t24.*t25.*8.119509961859382e-4;
t1222 = t24.*t25.*1.606961034807054e-3;
t1284 = t18.*t19.*t20.*2.761602722751607e-5;
t1285 = t18.*t19.*t26.*2.761602722751607e-5;
t1286 = t18.*t20.*t25.*2.761602722751607e-5;
t1287 = t19.*t20.*t24.*2.761602722751607e-5;
t1288 = t18.*t25.*t26.*2.761602722751607e-5;
t1289 = t19.*t24.*t26.*2.761602722751607e-5;
t1290 = t20.*t24.*t25.*2.761602722751607e-5;
t1293 = t24.*t25.*t26.*2.761602722751607e-5;
t1299 = t18.*t19.*t20.*t21.*5.958744043986595e-5;
t1300 = t18.*t19.*t20.*t27.*5.958744043986595e-5;
t1301 = t18.*t19.*t21.*t26.*5.958744043986595e-5;
t1302 = t18.*t20.*t21.*t25.*5.958744043986595e-5;
t1303 = t19.*t20.*t21.*t24.*5.958744043986595e-5;
t1305 = t18.*t20.*t25.*t27.*5.958744043986595e-5;
t1306 = t18.*t21.*t25.*t26.*5.958744043986595e-5;
t1307 = t19.*t20.*t24.*t27.*5.958744043986595e-5;
t1308 = t19.*t21.*t24.*t26.*5.958744043986595e-5;
t1309 = t20.*t21.*t24.*t25.*5.958744043986595e-5;
t1311 = t18.*t19.*t20.*t21.*2.71709233876478e-5;
t1312 = t20.*t24.*t25.*t27.*5.958744043986595e-5;
t1313 = t21.*t24.*t25.*t26.*5.958744043986595e-5;
t1315 = t18.*t19.*t20.*t27.*2.71709233876478e-5;
t1316 = t18.*t20.*t21.*t25.*2.71709233876478e-5;
t1317 = t19.*t20.*t21.*t24.*2.71709233876478e-5;
t1318 = t18.*t19.*t26.*t27.*2.71709233876478e-5;
t1319 = t18.*t20.*t25.*t27.*2.71709233876478e-5;
t1320 = t19.*t20.*t24.*t27.*2.71709233876478e-5;
t1321 = t20.*t21.*t24.*t25.*2.71709233876478e-5;
t1322 = t18.*t25.*t26.*t27.*2.71709233876478e-5;
t1323 = t19.*t24.*t26.*t27.*2.71709233876478e-5;
t1324 = t20.*t24.*t25.*t27.*2.71709233876478e-5;
t1328 = t24.*t25.*t26.*t27.*2.71709233876478e-5;
t1333 = t18.*t19.*t20.*t21.*4.570145693137498e-5;
t1336 = t18.*t19.*t20.*t27.*4.570145693137498e-5;
t1337 = t18.*t20.*t21.*t25.*4.570145693137498e-5;
t1338 = t19.*t20.*t21.*t24.*4.570145693137498e-5;
t1339 = t18.*t19.*t26.*t27.*4.570145693137498e-5;
t1340 = t18.*t20.*t25.*t27.*4.570145693137498e-5;
t1341 = t19.*t20.*t24.*t27.*4.570145693137498e-5;
t1342 = t20.*t21.*t24.*t25.*4.570145693137498e-5;
t1343 = t18.*t19.*t20.*3.091264323687963e-8;
t1346 = t18.*t25.*t26.*t27.*4.570145693137498e-5;
t1347 = t19.*t24.*t26.*t27.*4.570145693137498e-5;
t1348 = t20.*t24.*t25.*t27.*4.570145693137498e-5;
t1349 = t18.*t19.*t26.*3.091264323687963e-8;
t1350 = t18.*t20.*t25.*3.091264323687963e-8;
t1351 = t19.*t20.*t24.*3.091264323687963e-8;
t1354 = t24.*t25.*t26.*t27.*4.570145693137498e-5;
t1355 = t18.*t19.*t20.*4.645012099690971e-5;
t1356 = t18.*t25.*t26.*3.091264323687963e-8;
t1357 = t19.*t24.*t26.*3.091264323687963e-8;
t1358 = t20.*t24.*t25.*3.091264323687963e-8;
t1360 = t18.*t19.*t26.*4.645012099690971e-5;
t1361 = t18.*t20.*t25.*4.645012099690971e-5;
t1362 = t19.*t20.*t24.*4.645012099690971e-5;
t1363 = t24.*t25.*t26.*3.091264323687963e-8;
t1366 = t18.*t25.*t26.*4.645012099690971e-5;
t1367 = t19.*t24.*t26.*4.645012099690971e-5;
t1368 = t20.*t24.*t25.*4.645012099690971e-5;
t1369 = t24.*t25.*t26.*4.645012099690971e-5;
t1378 = t18.*t19.*t20.*t21.*1.002259954165347e-4;
t1384 = t18.*t19.*t20.*t27.*1.002259954165347e-4;
t1385 = t18.*t19.*t21.*t26.*1.002259954165347e-4;
t1386 = t18.*t20.*t21.*t25.*1.002259954165347e-4;
t1387 = t19.*t20.*t21.*t24.*1.002259954165347e-4;
t1392 = t18.*t20.*t25.*t27.*1.002259954165347e-4;
t1393 = t18.*t21.*t25.*t26.*1.002259954165347e-4;
t1394 = t19.*t20.*t24.*t27.*1.002259954165347e-4;
t1395 = t19.*t21.*t24.*t26.*1.002259954165347e-4;
t1396 = t20.*t21.*t24.*t25.*1.002259954165347e-4;
t1399 = t20.*t24.*t25.*t27.*1.002259954165347e-4;
t1400 = t21.*t24.*t25.*t26.*1.002259954165347e-4;
t1425 = t18.*t19.*t20.*5.199502473174935e-8;
t1427 = t18.*t19.*t26.*5.199502473174935e-8;
t1428 = t18.*t20.*t25.*5.199502473174935e-8;
t1429 = t19.*t20.*t24.*5.199502473174935e-8;
t1433 = t18.*t25.*t26.*5.199502473174935e-8;
t1434 = t19.*t24.*t26.*5.199502473174935e-8;
t1435 = t20.*t24.*t25.*5.199502473174935e-8;
t1438 = t24.*t25.*t26.*5.199502473174935e-8;
t44 = -t42;
t45 = t38.*4.602992943936994e+15;
t46 = t39.*4.602992943936994e+15;
t47 = t38.*7.742227997977903e+15;
t48 = t39.*7.742227997977903e+15;
t71 = -t55;
t72 = -t57;
t95 = -t86;
t97 = -t88;
t120 = -t98;
t121 = -t102;
t123 = t40+t41;
t124 = -t112;
t126 = -t117;
t128 = t27.*t99;
t130 = t27.*t100;
t133 = -t129;
t134 = t27.*t108;
t137 = t27.*t117;
t138 = -t135;
t151 = -t146;
t152 = -t147;
t173 = -t163;
t176 = -t164;
t182 = -t169;
t229 = -t208;
t236 = 1.0./t215;
t237 = t10.*t188;
t238 = t15.*t188;
t239 = -t220;
t240 = exp(t213);
t243 = -t224;
t244 = -t201;
t250 = exp(t235);
t252 = t189.*1i;
t256 = t27.*t220;
t258 = t202.*1i;
t259 = t27.*t230;
t261 = t27.*t231;
t262 = t20.*t201;
t264 = t26.*t201;
t265 = t215-1.0;
t271 = t27.*t216;
t275 = -t255;
t293 = -t277;
t295 = -t281;
t304 = t27.*t277;
t305 = t27.*t279;
t306 = t27.*t280;
t308 = t27.*t286;
t309 = -t302;
t311 = -t307;
t319 = -t313;
t323 = -t317;
t324 = t38.*3.222314966007e-4;
t325 = t39.*3.222314966007e-4;
t339 = -t327;
t340 = t39.*1.71926916309e-4;
t341 = t38.*4.567547574683999e-4;
t342 = t39.*4.567547574683999e-4;
t343 = -t332;
t344 = t38.*1.148721671835e-4;
t345 = t39.*1.148721671835e-4;
t346 = -t334;
t348 = t38.*4.573233567645e-4;
t349 = t39.*4.573233567645e-4;
t350 = t38.*1.71926916309e-4;
t363 = t38.*2.44005304615e-4;
t366 = t39.*2.44005304615e-4;
t369 = t38.*6.48243952274e-4;
t370 = t39.*6.48243952274e-4;
t371 = -t357;
t372 = t38.*1.630310061225e-4;
t374 = t39.*1.630310061225e-4;
t382 = -t367;
t389 = -t376;
t393 = -t384;
t410 = t55+t88;
t413 = -t397;
t414 = -t398;
t426 = -t405;
t445 = -t423;
t455 = -t441;
t456 = -t442;
t458 = -t444;
t471 = -t460;
t485 = -t462;
t486 = -t463;
t491 = -t470;
t493 = -t475;
t497 = -t487;
t498 = -t492;
t502 = t27.*t492;
t503 = t27.*t473;
t504 = t27.*t474;
t506 = t27.*t480;
t507 = -t499;
t508 = -t500;
t509 = -t501;
t511 = -t505;
t514 = t11.*t188.*8.595599785252598e-1;
t515 = t200.*3.064357668490995e+34;
t516 = t16.*t188.*8.595599785252598e-1;
t519 = t51.*t200;
t520 = t52.*t200;
t521 = t21.*t201.*8.595599785252598e-1;
t522 = t27.*t201.*8.595599785252598e-1;
t528 = t11.*t188.*5.157359871151559e-3;
t529 = t61.*t200;
t531 = t63.*t200;
t532 = t64.*t200;
t533 = t65.*t200;
t534 = t66.*t200;
t537 = t69.*t200;
t541 = t87.*t200;
t545 = t10.*t12.*t200.*-3.315051378778914e+33;
t547 = t10.*t16.*t200.*7.788445287802242e+33;
t548 = t11.*t15.*t200.*-1.990083581481952e+33;
t550 = t78.*t200;
t553 = t79.*t200;
t554 = t80.*t200;
t555 = t81.*t200;
t557 = t82.*t200;
t558 = t83.*t200;
t559 = t84.*t200;
t560 = t85.*t200;
t561 = t15.*t17.*t200.*-6.099194893302011e+33;
t562 = t21.*t201.*5.157359871151559e-3;
t566 = t104.*t200;
t567 = t105.*t200;
t568 = t106.*t200;
t570 = t93.*t200;
t582 = t11.*t17.*t200.*-1.025883768304404e+34;
t591 = t11.*t15.*t17.*t200.*-3.315051378778914e+33;
t595 = t115.*t200;
t596 = t116.*t200;
t599 = t118.*t200;
t602 = t119.*t200;
t619 = t11.*t12.*t15.*t200.*-6.099194893302011e+33;
t620 = t127.*t200;
t648 = t16.*t188.*8.595599785252598e-9;
t717 = -t684;
t718 = -t685;
t725 = -t688;
t736 = -t690;
t738 = -t695;
t740 = -t699;
t741 = -t700;
t756 = -t724;
t834 = t142.*t200;
t835 = t143.*t200;
t836 = t10.*t200.*-7.746286054220548e+49;
t837 = t15.*t200.*-7.746286054220548e+49;
t838 = t150.*t200;
t839 = t144.*t200;
t840 = t145.*t200;
t841 = t153.*t200;
t842 = t154.*t200;
t843 = t155.*t200;
t844 = t10.*t16.*t200.*-7.290917220067534e+49;
t845 = t15.*t16.*t200.*-7.290917220067534e+49;
t846 = t158.*t200;
t848 = t159.*t200;
t850 = (t50.*t189)./9.007199254740992e+15;
t851 = t166.*t200;
t852 = t168.*t200;
t853 = t170.*t200;
t854 = t171.*t200;
t855 = (t50.*t202)./9.007199254740992e+15;
t857 = t15.*t200.*-6.997781708721691e+52;
t860 = t10.*t16.*t200.*7.342112502577776e+52;
t861 = t178.*t200;
t862 = t179.*t200;
t863 = t180.*t200;
t864 = t181.*t200;
t866 = t174.*t200;
t867 = t175.*t200;
t869 = t177.*t200;
t874 = t50.*t188.*1.110223024625157e-16i;
t875 = t10.*t11.*t17.*t200.*-1.075008113939401e+50;
t876 = t191.*t200;
t877 = t192.*t200;
t878 = t50.*t201.*1.110223024625157e-16i;
t879 = t194.*t200;
t880 = t184.*t200;
t882 = t185.*t200;
t883 = t186.*t200;
t887 = t15.*t50.*t189.*(-1.110223024625157e-16);
t889 = t15.*t17.*t200.*-2.201616617347892e+53;
t890 = t10.*t12.*t200.*-1.196628789628727e+53;
t896 = t200.*t218;
t897 = t200.*t219;
t898 = t200.*t221;
t899 = t200.*t222;
t900 = t200.*t209;
t901 = t200.*t210;
t902 = t200.*t211;
t903 = t200.*t212;
t904 = t26.*t50.*t202.*(-1.110223024625157e-16);
t905 = t11.*t50.*t200.*7.432538878058787e+17i;
t906 = t200.*t242;
t908 = t15.*t16.*t50.*t200.*4.418873226179514e+17i;
t909 = t200.*t232;
t910 = t200.*t233;
t913 = t200.*t234;
t919 = t200.*t247;
t920 = t200.*t248;
t921 = t200.*t249;
t922 = t200.*t251;
t923 = t200.*t253;
t924 = t200.*t254;
t929 = t10.*t16.*t50.*t200.*-4.323455642275676e+17i;
t938 = t10.*t12.*t50.*t200.*-7.201947557068188e+17i;
t939 = t12.*t15.*t50.*t200.*-7.201947557068188e+17i;
t946 = t200.*t290;
t952 = t200.*t278;
t953 = t200.*t282;
t954 = t200.*t284;
t955 = t200.*t285;
t956 = t200.*t287;
t957 = t200.*t288;
t958 = t200.*t289;
t963 = t188.*7.38843356682345e-1;
t964 = t188.*2.61156643317655e-1;
t972 = (t15.*t50.*t189)./9.007199254740992e+23;
t975 = t10.*t12.*t16.*t50.*t200.*-1.325049802940888e+18i;
t977 = t10.*t16.*t17.*t50.*t200.*-7.201947557068188e+17i;
t983 = t188.*1.738813335718512e-2;
t986 = t201.*7.38843356682345e-1;
t988 = t201.*2.61156643317655e-1;
t996 = t201.*1.738813335718512e-2;
t998 = t188.*2.982577219529057e-2;
t1000 = t188.*4.721390555247569e-2;
t1001 = t11.*t188.*1.07201054193752e-2;
t1002 = t16.*t188.*1.07201054193752e-2;
t1003 = t201.*4.721390555247569e-2;
t1006 = t11.*t188.*4.888197259476159e-3;
t1008 = t16.*t188.*4.888197259476159e-3;
t1019 = t201.*2.982577219529057e-2;
t1030 = t188.*2.673231533213558e-6;
t1035 = t27.*t201.*1.07201054193752e-2;
t1039 = t188.*2.784974330421842e-6;
t1044 = t21.*t201.*4.888197259476159e-3;
t1047 = t15.*t17.*t200.*2.386997519508773e+34;
t1049 = t11.*t188.*2.691626116753997e-4;
t1055 = t12.*t15.*t200.*1.297387533374166e+34;
t1058 = t16.*t188.*8.76751178095765e-7;
t1065 = t11.*t188.*4.899491877593981e-7;
t1066 = t10.*t12.*t16.*t200.*2.386997519508773e+34;
t1067 = t21.*t201.*2.691626116753997e-4;
t1070 = t10.*t16.*t17.*t200.*1.297387533374166e+34;
t1071 = t16.*t188.*2.062943948460623e-7;
t1080 = t200.*t353;
t1082 = t200.*t355;
t1083 = t11.*t188.*3.438239914101039e-8;
t1084 = t16.*t188.*3.438239914101039e-8;
t1092 = t200.*t375;
t1096 = t200.*t377;
t1112 = t16.*t50.*t200.*-1.746965228796509e+32i;
t1126 = -t1089;
t1137 = t15.*t50.*t200.*-4.394953650240249e+33i;
t1143 = t200.*t390;
t1145 = t200.*t379;
t1148 = t200.*t383;
t1150 = -t1101;
t1154 = -t1115;
t1157 = t200.*t385;
t1161 = t200.*t386;
t1166 = t200.*t394;
t1167 = t200.*t395;
t1168 = t200.*t396;
t1170 = t10.*t11.*t50.*t200.*-1.03862462117543e+32i;
t1176 = -t1155;
t1177 = t11.*t50.*t200.*-6.957746211523004e+33i;
t1178 = t16.*t50.*t200.*-6.957746211523004e+33i;
t1179 = t200.*t401;
t1180 = t200.*t402;
t1181 = t200.*t403;
t1182 = t200.*t404;
t1183 = t200.*t406;
t1184 = t200.*t409;
t1185 = t15.*t16.*t50.*t200.*-4.136594366080324e+33i;
t1189 = t200.*t399;
t1192 = t200.*t400;
t1197 = t12.*t16.*t50.*t200.*-5.575912001630188e+33i;
t1198 = t12.*t16.*t50.*t200.*-1.025883768304404e+34i;
t1199 = t16.*t17.*t50.*t200.*-5.575912001630188e+33i;
t1201 = t200.*t415;
t1202 = t200.*t416;
t1203 = t200.*t417;
t1204 = t200.*t418;
t1212 = -t1190;
t1214 = -t1196;
t1223 = t10.*t11.*t17.*t50.*t200.*-3.315051378778914e+33i;
t1225 = t200.*t433;
t1227 = t200.*t435;
t1229 = t200.*t436;
t1230 = -t1210;
t1231 = t200.*t440;
t1232 = t200.*t443;
t1233 = t200.*t446;
t1234 = t200.*t447;
t1235 = -t1215;
t1236 = -t1216;
tau_c = ft_2({dq1,dq2,dq3,dq4,dq5,dq6,t10,t100,t1000,t1001,t1002,t1003,t1006,t1008,t101,t1019,t102,t103,t1030,t1035,t1039,t104,t1044,t1047,t1049,t1055,t1058,t106,t1065,t1066,t1067,t107,t1070,t1071,t108,t1080,t1083,t1084,t1089,t109,t1092,t11,t110,t1104,t1105,t1108,t111,t1110,t1112,t1113,t1114,t1115,t112,t1121,t1123,t1124,t1126,t113,t1137,t114,t1145,t1148,t115,t1150,t1154,t1158,t1159,t1162,t1166,t1167,t117,t1170,t1176,t1177,t1178,t1179,t118,t1180,t1184,t1185,t1189,t1190,t1192,t1193,t1194,t1196,t1197,t1198,t1199,t12,t120,t1202,t1203,t1204,t1205,t1207,t1208,t121,t1210,t1212,t1214,t1217,t1218,t1219,t122,t1220,t1221,t1222,t1223,t1229,t123,t1230,t1232,t1234,t1235,t1236,t124,t125,t126,t127,t128,t1284,t1285,t1286,t1287,t1288,t1289,t129,t1290,t1293,t1299,t13,t130,t1300,t1301,t1302,t1303,t1305,t1306,t1307,t1308,t1309,t1311,t1312,t1313,t1315,t1316,t1317,t1318,t1319,t132,t1320,t1321,t1322,t1323,t1324,t1328,t133,t1333,t1336,t1337,t1338,t1339,t134,t1340,t1341,t1342,t1343,t1346,t1347,t1348,t1349,t135,t1350,t1351,t1354,t1355,t1356,t1357,t1358,t136,t1360,t1361,t1362,t1363,t1366,t1367,t1368,t1369,t137,t1378,t138,t1384,t1385,t1386,t1387,t139,t1392,t1393,t1394,t1395,t1396,t1399,t14,t1400,t1425,t1427,t1428,t1429,t1433,t1434,t1435,t1438,t144,t145,t146,t147,t148,t149,t15,t150,t151,t152,t153,t156,t157,t158,t16,t160,t161,t162,t163,t164,t165,t166,t167,t168,t169,t17,t170,t171,t172,t173,t174,t175,t176,t177,t178,t18,t180,t181,t182,t185,t186,t188,t189,t19,t190,t191,t192,t195,t196,t197,t198,t20,t200,t201,t202,t203,t204,t205,t207,t208,t209,t21,t210,t211,t212,t216,t217,t218,t219,t22,t220,t221,t223,t224,t225,t226,t227,t229,t230,t231,t233,t236,t237,t238,t239,t24,t240,t241,t242,t243,t244,t245,t246,t247,t25,t250,t251,t252,t255,t256,t257,t258,t259,t26,t260,t261,t262,t263,t264,t265,t266,t267,t269,t27,t270,t271,t272,t273,t274,t275,t276,t277,t279,t28,t280,t281,t282,t283,t285,t286,t289,t29,t293,t294,t295,t296,t297,t298,t299,t30,t301,t302,t303,t304,t305,t306,t307,t308,t309,t31,t310,t311,t312,t313,t314,t315,t316,t318,t319,t32,t320,t321,t322,t323,t324,t325,t326,t328,t329,t33,t330,t331,t332,t333,t338,t339,t34,t340,t341,t342,t343,t344,t345,t346,t348,t349,t35,t350,t355,t358,t359,t36,t360,t363,t364,t365,t366,t368,t369,t370,t371,t372,t373,t374,t376,t377,t378,t38,t381,t382,t384,t385,t386,t388,t389,t39,t390,t391,t392,t393,t396,t397,t398,t403,t404,t405,t406,t407,t408,t410,t411,t412,t413,t414,t415,t419,t42,t420,t421,t422,t423,t424,t425,t426,t427,t428,t43,t430,t431,t432,t433,t434,t435,t437,t438,t439,t44,t440,t441,t442,t444,t445,t446,t448,t449,t45,t450,t451,t452,t453,t454,t455,t456,t457,t458,t459,t46,t460,t461,t462,t463,t464,t465,t466,t467,t468,t469,t47,t470,t471,t472,t473,t474,t475,t476,t477,t478,t479,t48,t480,t481,t482,t483,t484,t485,t486,t487,t488,t489,t490,t491,t492,t493,t494,t495,t496,t497,t498,t499,t50,t500,t501,t502,t503,t504,t505,t506,t507,t508,t509,t51,t510,t511,t514,t515,t516,t519,t52,t520,t521,t522,t528,t53,t531,t532,t533,t537,t54,t545,t547,t548,t550,t553,t554,t555,t557,t559,t56,t560,t561,t562,t566,t568,t57,t570,t58,t582,t583,t584,t585,t589,t59,t590,t591,t592,t595,t597,t599,t60,t600,t601,t605,t606,t607,t608,t609,t619,t620,t621,t622,t628,t63,t635,t636,t638,t64,t640,t641,t642,t643,t645,t646,t648,t649,t65,t654,t655,t656,t657,t659,t660,t663,t664,t665,t666,t667,t668,t669,t67,t670,t672,t673,t674,t675,t676,t677,t678,t679,t68,t681,t682,t683,t684,t685,t686,t687,t689,t69,t691,t692,t693,t694,t70,t702,t704,t705,t707,t708,t71,t710,t711,t712,t713,t714,t715,t716,t717,t718,t719,t72,t720,t721,t722,t723,t724,t725,t726,t728,t73,t736,t738,t740,t741,t742,t743,t744,t745,t746,t747,t749,t75,t750,t751,t755,t756,t757,t758,t759,t76,t762,t763,t764,t766,t768,t77,t770,t771,t772,t773,t774,t775,t776,t777,t778,t78,t781,t782,t783,t784,t785,t786,t787,t789,t79,t790,t791,t792,t793,t794,t796,t797,t798,t799,t8,t80,t800,t801,t802,t806,t807,t808,t809,t81,t812,t813,t816,t817,t818,t819,t82,t820,t821,t822,t823,t824,t825,t826,t827,t828,t829,t830,t831,t832,t833,t836,t837,t838,t839,t84,t840,t841,t844,t845,t846,t85,t850,t851,t852,t853,t854,t855,t857,t86,t860,t861,t863,t864,t866,t867,t869,t874,t875,t876,t877,t878,t882,t883,t887,t889,t89,t890,t896,t897,t898,t9,t90,t900,t901,t902,t903,t904,t905,t906,t908,t909,t91,t913,t92,t920,t921,t923,t924,t929,t93,t938,t939,t94,t946,t95,t952,t954,t956,t957,t96,t963,t964,t97,t972,t975,t977,t98,t983,t986,t988,t99,t996,t998});
end
function tau_c = ft_2(ct)
dq1 = ct{1};
dq2 = ct{2};
dq3 = ct{3};
dq4 = ct{4};
dq5 = ct{5};
dq6 = ct{6};
t10 = ct{7};
t100 = ct{8};
t1000 = ct{9};
t1001 = ct{10};
t1002 = ct{11};
t1003 = ct{12};
t1006 = ct{13};
t1008 = ct{14};
t101 = ct{15};
t1019 = ct{16};
t102 = ct{17};
t103 = ct{18};
t1030 = ct{19};
t1035 = ct{20};
t1039 = ct{21};
t104 = ct{22};
t1044 = ct{23};
t1047 = ct{24};
t1049 = ct{25};
t1055 = ct{26};
t1058 = ct{27};
t106 = ct{28};
t1065 = ct{29};
t1066 = ct{30};
t1067 = ct{31};
t107 = ct{32};
t1070 = ct{33};
t1071 = ct{34};
t108 = ct{35};
t1080 = ct{36};
t1083 = ct{37};
t1084 = ct{38};
t1089 = ct{39};
t109 = ct{40};
t1092 = ct{41};
t11 = ct{42};
t110 = ct{43};
t1104 = ct{44};
t1105 = ct{45};
t1108 = ct{46};
t111 = ct{47};
t1110 = ct{48};
t1112 = ct{49};
t1113 = ct{50};
t1114 = ct{51};
t1115 = ct{52};
t112 = ct{53};
t1121 = ct{54};
t1123 = ct{55};
t1124 = ct{56};
t1126 = ct{57};
t113 = ct{58};
t1137 = ct{59};
t114 = ct{60};
t1145 = ct{61};
t1148 = ct{62};
t115 = ct{63};
t1150 = ct{64};
t1154 = ct{65};
t1158 = ct{66};
t1159 = ct{67};
t1162 = ct{68};
t1166 = ct{69};
t1167 = ct{70};
t117 = ct{71};
t1170 = ct{72};
t1176 = ct{73};
t1177 = ct{74};
t1178 = ct{75};
t1179 = ct{76};
t118 = ct{77};
t1180 = ct{78};
t1184 = ct{79};
t1185 = ct{80};
t1189 = ct{81};
t1190 = ct{82};
t1192 = ct{83};
t1193 = ct{84};
t1194 = ct{85};
t1196 = ct{86};
t1197 = ct{87};
t1198 = ct{88};
t1199 = ct{89};
t12 = ct{90};
t120 = ct{91};
t1202 = ct{92};
t1203 = ct{93};
t1204 = ct{94};
t1205 = ct{95};
t1207 = ct{96};
t1208 = ct{97};
t121 = ct{98};
t1210 = ct{99};
t1212 = ct{100};
t1214 = ct{101};
t1217 = ct{102};
t1218 = ct{103};
t1219 = ct{104};
t122 = ct{105};
t1220 = ct{106};
t1221 = ct{107};
t1222 = ct{108};
t1223 = ct{109};
t1229 = ct{110};
t123 = ct{111};
t1230 = ct{112};
t1232 = ct{113};
t1234 = ct{114};
t1235 = ct{115};
t1236 = ct{116};
t124 = ct{117};
t125 = ct{118};
t126 = ct{119};
t127 = ct{120};
t128 = ct{121};
t1284 = ct{122};
t1285 = ct{123};
t1286 = ct{124};
t1287 = ct{125};
t1288 = ct{126};
t1289 = ct{127};
t129 = ct{128};
t1290 = ct{129};
t1293 = ct{130};
t1299 = ct{131};
t13 = ct{132};
t130 = ct{133};
t1300 = ct{134};
t1301 = ct{135};
t1302 = ct{136};
t1303 = ct{137};
t1305 = ct{138};
t1306 = ct{139};
t1307 = ct{140};
t1308 = ct{141};
t1309 = ct{142};
t1311 = ct{143};
t1312 = ct{144};
t1313 = ct{145};
t1315 = ct{146};
t1316 = ct{147};
t1317 = ct{148};
t1318 = ct{149};
t1319 = ct{150};
t132 = ct{151};
t1320 = ct{152};
t1321 = ct{153};
t1322 = ct{154};
t1323 = ct{155};
t1324 = ct{156};
t1328 = ct{157};
t133 = ct{158};
t1333 = ct{159};
t1336 = ct{160};
t1337 = ct{161};
t1338 = ct{162};
t1339 = ct{163};
t134 = ct{164};
t1340 = ct{165};
t1341 = ct{166};
t1342 = ct{167};
t1343 = ct{168};
t1346 = ct{169};
t1347 = ct{170};
t1348 = ct{171};
t1349 = ct{172};
t135 = ct{173};
t1350 = ct{174};
t1351 = ct{175};
t1354 = ct{176};
t1355 = ct{177};
t1356 = ct{178};
t1357 = ct{179};
t1358 = ct{180};
t136 = ct{181};
t1360 = ct{182};
t1361 = ct{183};
t1362 = ct{184};
t1363 = ct{185};
t1366 = ct{186};
t1367 = ct{187};
t1368 = ct{188};
t1369 = ct{189};
t137 = ct{190};
t1378 = ct{191};
t138 = ct{192};
t1384 = ct{193};
t1385 = ct{194};
t1386 = ct{195};
t1387 = ct{196};
t139 = ct{197};
t1392 = ct{198};
t1393 = ct{199};
t1394 = ct{200};
t1395 = ct{201};
t1396 = ct{202};
t1399 = ct{203};
t14 = ct{204};
t1400 = ct{205};
t1425 = ct{206};
t1427 = ct{207};
t1428 = ct{208};
t1429 = ct{209};
t1433 = ct{210};
t1434 = ct{211};
t1435 = ct{212};
t1438 = ct{213};
t144 = ct{214};
t145 = ct{215};
t146 = ct{216};
t147 = ct{217};
t148 = ct{218};
t149 = ct{219};
t15 = ct{220};
t150 = ct{221};
t151 = ct{222};
t152 = ct{223};
t153 = ct{224};
t156 = ct{225};
t157 = ct{226};
t158 = ct{227};
t16 = ct{228};
t160 = ct{229};
t161 = ct{230};
t162 = ct{231};
t163 = ct{232};
t164 = ct{233};
t165 = ct{234};
t166 = ct{235};
t167 = ct{236};
t168 = ct{237};
t169 = ct{238};
t17 = ct{239};
t170 = ct{240};
t171 = ct{241};
t172 = ct{242};
t173 = ct{243};
t174 = ct{244};
t175 = ct{245};
t176 = ct{246};
t177 = ct{247};
t178 = ct{248};
t18 = ct{249};
t180 = ct{250};
t181 = ct{251};
t182 = ct{252};
t185 = ct{253};
t186 = ct{254};
t188 = ct{255};
t189 = ct{256};
t19 = ct{257};
t190 = ct{258};
t191 = ct{259};
t192 = ct{260};
t195 = ct{261};
t196 = ct{262};
t197 = ct{263};
t198 = ct{264};
t20 = ct{265};
t200 = ct{266};
t201 = ct{267};
t202 = ct{268};
t203 = ct{269};
t204 = ct{270};
t205 = ct{271};
t207 = ct{272};
t208 = ct{273};
t209 = ct{274};
t21 = ct{275};
t210 = ct{276};
t211 = ct{277};
t212 = ct{278};
t216 = ct{279};
t217 = ct{280};
t218 = ct{281};
t219 = ct{282};
t22 = ct{283};
t220 = ct{284};
t221 = ct{285};
t223 = ct{286};
t224 = ct{287};
t225 = ct{288};
t226 = ct{289};
t227 = ct{290};
t229 = ct{291};
t230 = ct{292};
t231 = ct{293};
t233 = ct{294};
t236 = ct{295};
t237 = ct{296};
t238 = ct{297};
t239 = ct{298};
t24 = ct{299};
t240 = ct{300};
t241 = ct{301};
t242 = ct{302};
t243 = ct{303};
t244 = ct{304};
t245 = ct{305};
t246 = ct{306};
t247 = ct{307};
t25 = ct{308};
t250 = ct{309};
t251 = ct{310};
t252 = ct{311};
t255 = ct{312};
t256 = ct{313};
t257 = ct{314};
t258 = ct{315};
t259 = ct{316};
t26 = ct{317};
t260 = ct{318};
t261 = ct{319};
t262 = ct{320};
t263 = ct{321};
t264 = ct{322};
t265 = ct{323};
t266 = ct{324};
t267 = ct{325};
t269 = ct{326};
t27 = ct{327};
t270 = ct{328};
t271 = ct{329};
t272 = ct{330};
t273 = ct{331};
t274 = ct{332};
t275 = ct{333};
t276 = ct{334};
t277 = ct{335};
t279 = ct{336};
t28 = ct{337};
t280 = ct{338};
t281 = ct{339};
t282 = ct{340};
t283 = ct{341};
t285 = ct{342};
t286 = ct{343};
t289 = ct{344};
t29 = ct{345};
t293 = ct{346};
t294 = ct{347};
t295 = ct{348};
t296 = ct{349};
t297 = ct{350};
t298 = ct{351};
t299 = ct{352};
t30 = ct{353};
t301 = ct{354};
t302 = ct{355};
t303 = ct{356};
t304 = ct{357};
t305 = ct{358};
t306 = ct{359};
t307 = ct{360};
t308 = ct{361};
t309 = ct{362};
t31 = ct{363};
t310 = ct{364};
t311 = ct{365};
t312 = ct{366};
t313 = ct{367};
t314 = ct{368};
t315 = ct{369};
t316 = ct{370};
t318 = ct{371};
t319 = ct{372};
t32 = ct{373};
t320 = ct{374};
t321 = ct{375};
t322 = ct{376};
t323 = ct{377};
t324 = ct{378};
t325 = ct{379};
t326 = ct{380};
t328 = ct{381};
t329 = ct{382};
t33 = ct{383};
t330 = ct{384};
t331 = ct{385};
t332 = ct{386};
t333 = ct{387};
t338 = ct{388};
t339 = ct{389};
t34 = ct{390};
t340 = ct{391};
t341 = ct{392};
t342 = ct{393};
t343 = ct{394};
t344 = ct{395};
t345 = ct{396};
t346 = ct{397};
t348 = ct{398};
t349 = ct{399};
t35 = ct{400};
t350 = ct{401};
t355 = ct{402};
t358 = ct{403};
t359 = ct{404};
t36 = ct{405};
t360 = ct{406};
t363 = ct{407};
t364 = ct{408};
t365 = ct{409};
t366 = ct{410};
t368 = ct{411};
t369 = ct{412};
t370 = ct{413};
t371 = ct{414};
t372 = ct{415};
t373 = ct{416};
t374 = ct{417};
t376 = ct{418};
t377 = ct{419};
t378 = ct{420};
t38 = ct{421};
t381 = ct{422};
t382 = ct{423};
t384 = ct{424};
t385 = ct{425};
t386 = ct{426};
t388 = ct{427};
t389 = ct{428};
t39 = ct{429};
t390 = ct{430};
t391 = ct{431};
t392 = ct{432};
t393 = ct{433};
t396 = ct{434};
t397 = ct{435};
t398 = ct{436};
t403 = ct{437};
t404 = ct{438};
t405 = ct{439};
t406 = ct{440};
t407 = ct{441};
t408 = ct{442};
t410 = ct{443};
t411 = ct{444};
t412 = ct{445};
t413 = ct{446};
t414 = ct{447};
t415 = ct{448};
t419 = ct{449};
t42 = ct{450};
t420 = ct{451};
t421 = ct{452};
t422 = ct{453};
t423 = ct{454};
t424 = ct{455};
t425 = ct{456};
t426 = ct{457};
t427 = ct{458};
t428 = ct{459};
t43 = ct{460};
t430 = ct{461};
t431 = ct{462};
t432 = ct{463};
t433 = ct{464};
t434 = ct{465};
t435 = ct{466};
t437 = ct{467};
t438 = ct{468};
t439 = ct{469};
t44 = ct{470};
t440 = ct{471};
t441 = ct{472};
t442 = ct{473};
t444 = ct{474};
t445 = ct{475};
t446 = ct{476};
t448 = ct{477};
t449 = ct{478};
t45 = ct{479};
t450 = ct{480};
t451 = ct{481};
t452 = ct{482};
t453 = ct{483};
t454 = ct{484};
t455 = ct{485};
t456 = ct{486};
t457 = ct{487};
t458 = ct{488};
t459 = ct{489};
t46 = ct{490};
t460 = ct{491};
t461 = ct{492};
t462 = ct{493};
t463 = ct{494};
t464 = ct{495};
t465 = ct{496};
t466 = ct{497};
t467 = ct{498};
t468 = ct{499};
t469 = ct{500};
t47 = ct{501};
t470 = ct{502};
t471 = ct{503};
t472 = ct{504};
t473 = ct{505};
t474 = ct{506};
t475 = ct{507};
t476 = ct{508};
t477 = ct{509};
t478 = ct{510};
t479 = ct{511};
t48 = ct{512};
t480 = ct{513};
t481 = ct{514};
t482 = ct{515};
t483 = ct{516};
t484 = ct{517};
t485 = ct{518};
t486 = ct{519};
t487 = ct{520};
t488 = ct{521};
t489 = ct{522};
t490 = ct{523};
t491 = ct{524};
t492 = ct{525};
t493 = ct{526};
t494 = ct{527};
t495 = ct{528};
t496 = ct{529};
t497 = ct{530};
t498 = ct{531};
t499 = ct{532};
t50 = ct{533};
t500 = ct{534};
t501 = ct{535};
t502 = ct{536};
t503 = ct{537};
t504 = ct{538};
t505 = ct{539};
t506 = ct{540};
t507 = ct{541};
t508 = ct{542};
t509 = ct{543};
t51 = ct{544};
t510 = ct{545};
t511 = ct{546};
t514 = ct{547};
t515 = ct{548};
t516 = ct{549};
t519 = ct{550};
t52 = ct{551};
t520 = ct{552};
t521 = ct{553};
t522 = ct{554};
t528 = ct{555};
t53 = ct{556};
t531 = ct{557};
t532 = ct{558};
t533 = ct{559};
t537 = ct{560};
t54 = ct{561};
t545 = ct{562};
t547 = ct{563};
t548 = ct{564};
t550 = ct{565};
t553 = ct{566};
t554 = ct{567};
t555 = ct{568};
t557 = ct{569};
t559 = ct{570};
t56 = ct{571};
t560 = ct{572};
t561 = ct{573};
t562 = ct{574};
t566 = ct{575};
t568 = ct{576};
t57 = ct{577};
t570 = ct{578};
t58 = ct{579};
t582 = ct{580};
t583 = ct{581};
t584 = ct{582};
t585 = ct{583};
t589 = ct{584};
t59 = ct{585};
t590 = ct{586};
t591 = ct{587};
t592 = ct{588};
t595 = ct{589};
t597 = ct{590};
t599 = ct{591};
t60 = ct{592};
t600 = ct{593};
t601 = ct{594};
t605 = ct{595};
t606 = ct{596};
t607 = ct{597};
t608 = ct{598};
t609 = ct{599};
t619 = ct{600};
t620 = ct{601};
t621 = ct{602};
t622 = ct{603};
t628 = ct{604};
t63 = ct{605};
t635 = ct{606};
t636 = ct{607};
t638 = ct{608};
t64 = ct{609};
t640 = ct{610};
t641 = ct{611};
t642 = ct{612};
t643 = ct{613};
t645 = ct{614};
t646 = ct{615};
t648 = ct{616};
t649 = ct{617};
t65 = ct{618};
t654 = ct{619};
t655 = ct{620};
t656 = ct{621};
t657 = ct{622};
t659 = ct{623};
t660 = ct{624};
t663 = ct{625};
t664 = ct{626};
t665 = ct{627};
t666 = ct{628};
t667 = ct{629};
t668 = ct{630};
t669 = ct{631};
t67 = ct{632};
t670 = ct{633};
t672 = ct{634};
t673 = ct{635};
t674 = ct{636};
t675 = ct{637};
t676 = ct{638};
t677 = ct{639};
t678 = ct{640};
t679 = ct{641};
t68 = ct{642};
t681 = ct{643};
t682 = ct{644};
t683 = ct{645};
t684 = ct{646};
t685 = ct{647};
t686 = ct{648};
t687 = ct{649};
t689 = ct{650};
t69 = ct{651};
t691 = ct{652};
t692 = ct{653};
t693 = ct{654};
t694 = ct{655};
t70 = ct{656};
t702 = ct{657};
t704 = ct{658};
t705 = ct{659};
t707 = ct{660};
t708 = ct{661};
t71 = ct{662};
t710 = ct{663};
t711 = ct{664};
t712 = ct{665};
t713 = ct{666};
t714 = ct{667};
t715 = ct{668};
t716 = ct{669};
t717 = ct{670};
t718 = ct{671};
t719 = ct{672};
t72 = ct{673};
t720 = ct{674};
t721 = ct{675};
t722 = ct{676};
t723 = ct{677};
t724 = ct{678};
t725 = ct{679};
t726 = ct{680};
t728 = ct{681};
t73 = ct{682};
t736 = ct{683};
t738 = ct{684};
t740 = ct{685};
t741 = ct{686};
t742 = ct{687};
t743 = ct{688};
t744 = ct{689};
t745 = ct{690};
t746 = ct{691};
t747 = ct{692};
t749 = ct{693};
t75 = ct{694};
t750 = ct{695};
t751 = ct{696};
t755 = ct{697};
t756 = ct{698};
t757 = ct{699};
t758 = ct{700};
t759 = ct{701};
t76 = ct{702};
t762 = ct{703};
t763 = ct{704};
t764 = ct{705};
t766 = ct{706};
t768 = ct{707};
t77 = ct{708};
t770 = ct{709};
t771 = ct{710};
t772 = ct{711};
t773 = ct{712};
t774 = ct{713};
t775 = ct{714};
t776 = ct{715};
t777 = ct{716};
t778 = ct{717};
t78 = ct{718};
t781 = ct{719};
t782 = ct{720};
t783 = ct{721};
t784 = ct{722};
t785 = ct{723};
t786 = ct{724};
t787 = ct{725};
t789 = ct{726};
t79 = ct{727};
t790 = ct{728};
t791 = ct{729};
t792 = ct{730};
t793 = ct{731};
t794 = ct{732};
t796 = ct{733};
t797 = ct{734};
t798 = ct{735};
t799 = ct{736};
t8 = ct{737};
t80 = ct{738};
t800 = ct{739};
t801 = ct{740};
t802 = ct{741};
t806 = ct{742};
t807 = ct{743};
t808 = ct{744};
t809 = ct{745};
t81 = ct{746};
t812 = ct{747};
t813 = ct{748};
t816 = ct{749};
t817 = ct{750};
t818 = ct{751};
t819 = ct{752};
t82 = ct{753};
t820 = ct{754};
t821 = ct{755};
t822 = ct{756};
t823 = ct{757};
t824 = ct{758};
t825 = ct{759};
t826 = ct{760};
t827 = ct{761};
t828 = ct{762};
t829 = ct{763};
t830 = ct{764};
t831 = ct{765};
t832 = ct{766};
t833 = ct{767};
t836 = ct{768};
t837 = ct{769};
t838 = ct{770};
t839 = ct{771};
t84 = ct{772};
t840 = ct{773};
t841 = ct{774};
t844 = ct{775};
t845 = ct{776};
t846 = ct{777};
t85 = ct{778};
t850 = ct{779};
t851 = ct{780};
t852 = ct{781};
t853 = ct{782};
t854 = ct{783};
t855 = ct{784};
t857 = ct{785};
t86 = ct{786};
t860 = ct{787};
t861 = ct{788};
t863 = ct{789};
t864 = ct{790};
t866 = ct{791};
t867 = ct{792};
t869 = ct{793};
t874 = ct{794};
t875 = ct{795};
t876 = ct{796};
t877 = ct{797};
t878 = ct{798};
t882 = ct{799};
t883 = ct{800};
t887 = ct{801};
t889 = ct{802};
t89 = ct{803};
t890 = ct{804};
t896 = ct{805};
t897 = ct{806};
t898 = ct{807};
t9 = ct{808};
t90 = ct{809};
t900 = ct{810};
t901 = ct{811};
t902 = ct{812};
t903 = ct{813};
t904 = ct{814};
t905 = ct{815};
t906 = ct{816};
t908 = ct{817};
t909 = ct{818};
t91 = ct{819};
t913 = ct{820};
t92 = ct{821};
t920 = ct{822};
t921 = ct{823};
t923 = ct{824};
t924 = ct{825};
t929 = ct{826};
t93 = ct{827};
t938 = ct{828};
t939 = ct{829};
t94 = ct{830};
t946 = ct{831};
t95 = ct{832};
t952 = ct{833};
t954 = ct{834};
t956 = ct{835};
t957 = ct{836};
t96 = ct{837};
t963 = ct{838};
t964 = ct{839};
t97 = ct{840};
t972 = ct{841};
t975 = ct{842};
t977 = ct{843};
t98 = ct{844};
t983 = ct{845};
t986 = ct{846};
t988 = ct{847};
t99 = ct{848};
t996 = ct{849};
t998 = ct{850};
t1237 = -t1219;
t1238 = -t1220;
t1242 = t10.*t11.*t50.*t200.*-4.075691174875038e+36i;
t1243 = t200.*t448;
t1246 = t10.*t16.*t50.*t200.*-4.075691174875038e+36i;
t1247 = t200.*t449;
t1248 = t200.*t450;
t1249 = t200.*t451;
t1252 = t200.*t453;
t1253 = t200.*t454;
t1254 = t10.*t11.*t12.*t50.*t200.*-6.099194893302011e+33i;
t1255 = t15.*t16.*t50.*t200.*1.595073594941899e+37i;
t1256 = t11.*t15.*t17.*t50.*t200.*-6.099194893302011e+33i;
t1265 = t10.*t12.*t50.*t200.*-6.789225223739216e+36i;
t1267 = t12.*t15.*t50.*t200.*-6.789225223739216e+36i;
t1269 = t15.*t200.*7.152220999552773e+52;
t1273 = t200.*t472;
t1274 = t200.*t476;
t1275 = t200.*t477;
t1276 = t200.*t478;
t1277 = t200.*t481;
t1278 = t200.*t482;
t1279 = t200.*t483;
t1280 = t200.*t484;
t1291 = t10.*t11.*t12.*t50.*t200.*-1.249115114148252e+37i;
t1292 = t16.*t200.*3.147052781374869e+48;
t1294 = t10.*t12.*t16.*t50.*t200.*-1.249115114148252e+37i;
t1295 = t10.*t11.*t17.*t50.*t200.*-6.789225223739216e+36i;
t1297 = t10.*t16.*t17.*t50.*t200.*-6.789225223739216e+36i;
t1298 = t12.*t15.*t200.*1.223038087510652e+53;
t1327 = t15.*t17.*t200.*2.250205745048369e+53;
t1329 = t11.*t15.*t200.*1.871019782761396e+48;
t1334 = t11.*t200.*1.253396129822139e+50;
t1335 = -t1284;
t1344 = -t1288;
t1345 = -t1289;
t1352 = -t1293;
t1370 = -t1302;
t1371 = -t1303;
t1373 = t10.*t200.*7.917244648613035e+49;
t1374 = -t1306;
t1375 = -t1308;
t1376 = -t1309;
t1379 = -t1312;
t1380 = -t1313;
t1389 = -t1315;
t1397 = -t1318;
t1398 = -t1321;
t1404 = -t1333;
t1405 = -t1336;
t1406 = -t1339;
t1407 = -t1340;
t1408 = -t1341;
t1409 = -t1346;
t1410 = -t1347;
t1411 = -t1350;
t1412 = -t1351;
t1413 = t10.*t16.*t17.*t200.*1.223038087510652e+53;
t1414 = -t1355;
t1415 = -t1356;
t1416 = -t1357;
t1417 = -t1358;
t1419 = -t1361;
t1420 = -t1362;
t1421 = -t1363;
t1424 = -t1369;
t1430 = t10.*t12.*t16.*t200.*2.250205745048369e+53;
t1436 = -t1384;
t1440 = -t1396;
t1441 = -t1400;
t1443 = t16.*t17.*t200.*1.004467008511696e+50;
t1445 = t15.*t16.*t200.*7.451825938264896e+49;
t1446 = t12.*t16.*t200.*1.848067902664462e+50;
t1447 = -t1435;
t1448 = -t1438;
t1454 = t10.*t50.*t189.*5.673626844500105e-17;
t1455 = t15.*t50.*t189.*5.673626844500105e-17;
t1456 = t11.*t50.*t189.*9.543032792050485e-17;
t1458 = t16.*t50.*t189.*9.543032792050485e-17;
t1470 = t11.*t15.*t17.*t200.*5.971865661673106e+49;
t1473 = t11.*t12.*t15.*t200.*1.098733273949399e+50;
t1474 = t20.*t50.*t202.*5.673626844500105e-17;
t1475 = t26.*t50.*t202.*5.673626844500105e-17;
t1477 = t21.*t50.*t202.*9.543032792050485e-17;
t1478 = t27.*t50.*t202.*9.543032792050485e-17;
t1480 = t10.*t50.*t189.*6.489053738789607e-19;
t1481 = t15.*t50.*t189.*6.489053738789607e-19;
t1483 = t10.*t50.*t189.*1.092459456231154e-21;
t1488 = t11.*t50.*t189.*5.725819675230291e-19;
t1490 = t10.*t50.*t189.*7.194245199571015e-21;
t1491 = t50.*t200.*6.804240878490729e+18i;
t1492 = t16.*t50.*t189.*5.725819675230291e-19;
t1493 = t15.*t50.*t189.*7.194245199571015e-21;
t1496 = t10.*t11.*t50.*t189.*1.384627967837559e-18;
t1497 = t10.*t16.*t50.*t189.*1.384627967837559e-18;
t1498 = t11.*t15.*t50.*t189.*1.384627967837559e-18;
t1500 = t10.*t16.*t50.*t189.*6.313682909819818e-19;
t1501 = t15.*t16.*t50.*t189.*6.313682909819818e-19;
t1503 = t26.*t50.*t202.*6.489053738789607e-19;
t1509 = t10.*t11.*t50.*t189.*6.313682909819818e-19;
t1511 = t15.*t50.*t189.*6.88338275267597e-23;
t1513 = t21.*t50.*t202.*5.725819675230291e-19;
t1514 = t27.*t50.*t202.*5.725819675230291e-19;
t1515 = t26.*t50.*t202.*7.194245199571015e-21;
t1517 = t10.*t50.*t189.*6.417111286793897e-19;
t1518 = t15.*t50.*t189.*3.597122599785507e-22;
t1519 = t10.*t50.*t189.*7.183142969324763e-22;
t1520 = t15.*t50.*t189.*8.693046282814975e-22;
t1521 = t15.*t50.*t189.*7.183142969324763e-22;
t1523 = t10.*t17.*t50.*t200.*1.354293320444013e+18i;
t1524 = t10.*t12.*t50.*t200.*7.360892737071442e+17i;
t1528 = t11.*t12.*t50.*t200.*2.277919560321538e+18i;
t1530 = t11.*t17.*t50.*t200.*1.238101177498716e+18i;
t1537 = t20.*t50.*t202.*7.183142969324763e-22;
t1538 = t10.*t50.*t189.*5.673626844500105e-25;
t1539 = t15.*t50.*t189.*5.673626844500105e-25;
t1541 = t12.*t15.*t16.*t50.*t200.*1.354293320444013e+18i;
t1542 = t15.*t16.*t17.*t50.*t200.*7.360892737071442e+17i;
t1545 = t11.*t50.*t189.*9.543032792050485e-25;
t1546 = t16.*t50.*t189.*9.543032792050485e-25;
t1560 = t8.*t9.*t188.*1.374006108587572e-3;
t1561 = t8.*t14.*t188.*1.374006108587572e-3;
t1562 = t9.*t13.*t188.*1.374006108587572e-3;
t1563 = t13.*t14.*t188.*1.374006108587572e-3;
t1566 = t13.*t14.*t188.*6.463878411896211e-3;
t1567 = t8.*t9.*t188.*2.311076443710702e-3;
t1570 = t8.*t14.*t188.*2.311076443710702e-3;
t1571 = t9.*t13.*t188.*2.311076443710702e-3;
t1573 = t13.*t14.*t188.*2.311076443710702e-3;
t1576 = t8.*t9.*t188.*6.463878411896211e-3;
t1577 = t8.*t14.*t188.*6.463878411896211e-3;
t1578 = t9.*t13.*t188.*6.463878411896211e-3;
t1581 = t8.*t9.*t188.*1.087223487536e-2;
t1582 = t201.*8.618586366948822e-4;
t1584 = t8.*t14.*t188.*1.087223487536e-2;
t1585 = t9.*t13.*t188.*1.087223487536e-2;
t1586 = t13.*t14.*t188.*1.087223487536e-2;
t1587 = t8.*t9.*t188.*2.550195842399381e-2;
t1589 = t8.*t14.*t188.*2.550195842399381e-2;
t1590 = t9.*t13.*t188.*2.550195842399381e-2;
t1591 = t13.*t14.*t188.*2.550195842399381e-2;
t1593 = t201.*5.135409293037228e-4;
t1607 = t8.*t9.*t188.*4.289426008649035e-2;
t1608 = t8.*t14.*t188.*4.289426008649035e-2;
t1609 = t9.*t13.*t188.*4.289426008649035e-2;
t1611 = t13.*t14.*t188.*4.289426008649035e-2;
t1614 = t18.*t19.*t201.*6.463878411896211e-3;
t1615 = t18.*t25.*t201.*6.463878411896211e-3;
t1616 = t19.*t24.*t201.*6.463878411896211e-3;
t1617 = t24.*t25.*t201.*6.463878411896211e-3;
t1621 = t21.*t201.*5.316843277159623e-5;
t1623 = t27.*t201.*5.316843277159623e-5;
t1624 = t21.*t201.*1.166015146360021e-4;
t1625 = t27.*t201.*1.166015146360021e-4;
t1638 = t18.*t19.*t201.*1.087223487536e-2;
t1648 = t18.*t25.*t201.*1.087223487536e-2;
t1649 = t19.*t24.*t201.*1.087223487536e-2;
t1660 = t24.*t25.*t201.*1.087223487536e-2;
t1686 = t18.*t19.*t201.*2.550195842399381e-2;
t1688 = t18.*t25.*t201.*2.550195842399381e-2;
t1689 = t19.*t24.*t201.*2.550195842399381e-2;
t1690 = t24.*t25.*t201.*2.550195842399381e-2;
t1695 = t10.*t50.*t200.*1.553819674864718e+37i;
t1700 = t18.*t25.*t201.*4.289426008649035e-2;
t1701 = t19.*t24.*t201.*4.289426008649035e-2;
t1702 = t24.*t25.*t201.*4.289426008649035e-2;
t1750 = t18.*t19.*t201.*4.289426008649035e-2;
t1765 = t10.*t17.*t50.*t200.*4.888570919953966e+37i;
t1780 = t10.*t12.*t50.*t200.*2.657049668350291e+37i;
t1782 = t15.*t50.*t200.*1.720021026545681e+34i;
t1795 = t12.*t15.*t16.*t50.*t200.*4.888570919953966e+37i;
t1796 = t10.*t11.*t50.*t200.*4.064789595703988e+32i;
t1797 = t15.*t16.*t17.*t50.*t200.*2.657049668350291e+37i;
t1798 = t10.*t16.*t50.*t200.*1.618908833671003e+34i;
t1807 = t10.*t11.*t12.*t50.*t200.*2.386997519508773e+34i;
t1817 = t10.*t11.*t17.*t50.*t200.*1.297387533374166e+34i;
t1863 = t10.*t50.*t189.*(t42-t43).*(-1.232595164407831e-32);
t1865 = t15.*t50.*t189.*(t42-t43).*(-1.232595164407831e-32);
t1868 = (t10.*t50.*t189.*(t42-t43))./8.112963841460668e+31;
t1870 = t50.*t189.*1.930470600839964e-18;
t1871 = t10.*t50.*t189.*5.582848814988104e-22;
t1872 = t15.*t50.*t189.*5.582848814988104e-22;
t1873 = t50.*t189.*3.311325901843639e-18;
t1874 = t50.*t189.*5.241796502683603e-18;
t1875 = t50.*t189.*5.241796502683603e-18;
t1876 = t50.*t202.*1.930470600839964e-18;
t1877 = t50.*t202.*3.311325901843639e-18;
t1879 = t50.*t202.*5.241796502683603e-18;
t1880 = t35.*t50.*t189.*2.899421184450801e-17;
t1881 = t36.*t50.*t189.*2.899421184450801e-17;
t1882 = t11.*t50.*t189.*5.426989146380022e-19;
t1883 = t11.*t50.*t189.*5.426989146380022e-19;
t1884 = t16.*t50.*t189.*5.426989146380022e-19;
t1886 = t10.*t50.*t189.*3.31613276532711e-19;
t1887 = t15.*t50.*t189.*3.31613276532711e-19;
t1889 = t11.*t50.*t189.*1.190170786299927e-18;
t1890 = t16.*t50.*t189.*1.190170786299927e-18;
t1891 = t16.*t50.*t189.*1.190170786299927e-18;
t1894 = t10.*t50.*t189.*3.676510195236068e-21;
t1895 = t10.*t50.*t189.*3.676510195236068e-21;
t1897 = t15.*t50.*t189.*3.676510195236068e-21;
t1898 = t10.*t50.*t189.*4.442449819243582e-22;
t1899 = t15.*t50.*t189.*4.442449819243582e-22;
t1901 = t35.*t50.*t189.*8.202809061800765e-17;
t1902 = t36.*t50.*t189.*8.202809061800765e-17;
t1903 = t10.*t50.*t189.*3.517648643590065e-23;
t1904 = t15.*t50.*t189.*3.517648643590065e-23;
t1907 = t50.*t189.*3.091942624624357e-22;
t1909 = t10.*t11.*t50.*t189.*7.075931802640439e-19;
t1914 = t10.*t16.*t50.*t189.*7.075931802640439e-19;
t1915 = t11.*t15.*t50.*t189.*7.075931802640439e-19;
t1916 = t11.*t15.*t50.*t189.*7.075931802640439e-19;
t1917 = t10.*t50.*t189.*1.838255097618034e-22;
t1919 = t15.*t50.*t189.*1.838255097618034e-22;
t1920 = t10.*t11.*t50.*t189.*3.226512155691387e-19;
t1922 = t10.*t16.*t50.*t189.*3.226512155691387e-19;
t1923 = t21.*t50.*t202.*5.426989146380022e-19;
t1924 = t15.*t16.*t50.*t189.*3.226512155691387e-19;
t1925 = t15.*t16.*t50.*t189.*3.226512155691387e-19;
t1926 = t27.*t50.*t202.*5.426989146380022e-19;
t1927 = t20.*t50.*t202.*3.31613276532711e-19;
t1928 = t50.*t189.*2.967883198327701e-22;
t1929 = t26.*t50.*t202.*3.31613276532711e-19;
t1930 = t21.*t50.*t202.*1.190170786299927e-18;
t1931 = t27.*t50.*t202.*1.190170786299927e-18;
t1936 = t10.*t50.*t189.*3.279367663374749e-19;
t1937 = t15.*t50.*t189.*3.279367663374749e-19;
t1940 = t10.*t50.*t189.*3.670836568391568e-22;
t1941 = t38.*t50.*t202.*2.899421184450801e-17;
t1942 = t15.*t50.*t189.*3.670836568391568e-22;
t1943 = t39.*t50.*t202.*2.899421184450801e-17;
t1947 = t11.*t50.*t189.*2.988305288502687e-20;
t1948 = t16.*t50.*t189.*2.988305288502687e-20;
t1949 = t20.*t50.*t202.*3.676510195236068e-21;
t1950 = t26.*t50.*t202.*3.676510195236068e-21;
t1951 = t11.*t50.*t189.*5.439528691468777e-23;
t1952 = t16.*t50.*t189.*5.439528691468777e-23;
t1953 = t11.*t50.*t189.*9.733893447891495e-23;
t1956 = t16.*t50.*t189.*9.733893447891495e-23;
t1958 = t38.*t50.*t202.*8.202809061800765e-17;
t1959 = t39.*t50.*t202.*8.202809061800765e-17;
t1960 = t20.*t50.*t202.*1.875105520197095e-20;
t1961 = t26.*t50.*t202.*1.875105520197095e-20;
t1965 = t11.*t50.*t189.*2.290327870092116e-23;
t1966 = t16.*t50.*t189.*2.290327870092116e-23;
t1967 = t20.*t50.*t202.*3.670836568391568e-22;
t1968 = t26.*t50.*t202.*3.670836568391568e-22;
t1970 = t21.*t50.*t202.*2.988305288502687e-20;
t1971 = t27.*t50.*t202.*2.988305288502687e-20;
t1975 = t8.*t11.*t14.*t15.*t50.*t189.*3.226512155691387e-19;
t1977 = t9.*t11.*t13.*t15.*t50.*t189.*3.226512155691387e-19;
t1982 = t11.*t13.*t14.*t15.*t50.*t189.*3.226512155691387e-19;
t1991 = t20.*t50.*t202.*7.825108561121397e-23;
t1997 = t26.*t50.*t202.*7.825108561121397e-23;
t2017 = t8.*t9.*t15.*t16.*t50.*t189.*7.075931802640439e-19;
t2021 = t8.*t14.*t15.*t16.*t50.*t189.*7.075931802640439e-19;
t2022 = t9.*t13.*t15.*t16.*t50.*t189.*7.075931802640439e-19;
t2024 = t11.*t50.*t189.*3.817213116820194e-24;
t2025 = t13.*t14.*t15.*t16.*t50.*t189.*7.075931802640439e-19;
t2027 = t8.*t9.*t11.*t15.*t50.*t189.*3.226512155691387e-19;
t2028 = t16.*t50.*t189.*3.817213116820194e-24;
t2029 = t8.*t9.*t15.*t16.*t50.*t189.*(-3.226512155691387e-19);
t2030 = t8.*t10.*t14.*t16.*t50.*t189.*(-3.226512155691387e-19);
t2032 = t9.*t10.*t13.*t16.*t50.*t189.*(-3.226512155691387e-19);
t2034 = t20.*t50.*t202.*2.075672598245148e-23;
t2035 = t20.*t27.*t50.*t202.*6.867329764181918e-21;
t2038 = t26.*t50.*t202.*2.075672598245148e-23;
t2039 = t26.*t27.*t50.*t202.*6.867329764181918e-21;
t2043 = t8.*t9.*t15.*t16.*t50.*t189.*(-5.426989146380022e-19);
t2044 = t8.*t10.*t14.*t16.*t50.*t189.*(-5.426989146380022e-19);
t2045 = t9.*t10.*t13.*t16.*t50.*t189.*(-5.426989146380022e-19);
t2049 = t8.*t14.*t15.*t16.*t50.*t189.*(-5.426989146380022e-19);
t2050 = t9.*t13.*t15.*t16.*t50.*t189.*(-5.426989146380022e-19);
t2051 = t10.*t13.*t14.*t16.*t50.*t189.*(-5.426989146380022e-19);
t2052 = t11.*t13.*t14.*t15.*t50.*t189.*(-5.426989146380022e-19);
t2054 = t8.*t9.*t10.*t11.*t50.*t189.*(-1.190170786299927e-18);
t2055 = t20.*t21.*t50.*t202.*1.506045994337235e-20;
t2056 = t20.*t27.*t50.*t202.*1.506045994337235e-20;
t2057 = t21.*t26.*t50.*t202.*1.506045994337235e-20;
t2058 = t11.*t13.*t14.*t15.*t50.*t189.*(-1.190170786299927e-18);
t2059 = t13.*t14.*t15.*t16.*t50.*t189.*(-1.190170786299927e-18);
t2061 = t8.*t11.*t14.*t15.*t50.*t189.*(-7.075931802640439e-19);
t2062 = t9.*t11.*t13.*t15.*t50.*t189.*(-7.075931802640439e-19);
t2063 = t10.*t11.*t13.*t14.*t50.*t189.*(-7.075931802640439e-19);
t2069 = t11.*t13.*t14.*t15.*t50.*t189.*(-7.075931802640439e-19);
t2075 = t8.*t9.*t10.*t16.*t50.*t189.*(-3.226512155691387e-19);
t2077 = t20.*t21.*t50.*t202.*6.867329764181918e-21;
t2080 = t8.*t9.*t10.*t50.*t189.*6.174342216456664e-22;
t2081 = t8.*t14.*t15.*t50.*t189.*(-3.670836568391568e-22);
t2082 = t9.*t13.*t15.*t50.*t189.*(-3.670836568391568e-22);
t2083 = t10.*t13.*t14.*t50.*t189.*(-3.670836568391568e-22);
t2084 = t8.*t9.*t15.*t50.*t189.*6.174342216456664e-22;
t2085 = t8.*t10.*t14.*t50.*t189.*6.174342216456664e-22;
t2086 = t9.*t10.*t13.*t50.*t189.*6.174342216456664e-22;
t2087 = t13.*t14.*t15.*t50.*t189.*(-3.670836568391568e-22);
t2088 = t26.*t50.*t202.*7.813032776304851e-24;
t2089 = t8.*t14.*t15.*t50.*t189.*6.174342216456664e-22;
t2090 = t9.*t13.*t15.*t50.*t189.*6.174342216456664e-22;
t2091 = t10.*t13.*t14.*t50.*t189.*6.174342216456664e-22;
t2092 = t13.*t14.*t15.*t50.*t189.*6.174342216456664e-22;
t2093 = t20.*t50.*t202.*6.979827775532854e-21;
t2096 = t8.*t9.*t10.*t50.*t189.*5.515892039870764e-19;
t2097 = t8.*t9.*t15.*t50.*t189.*5.515892039870764e-19;
t2098 = t8.*t10.*t14.*t50.*t189.*5.515892039870764e-19;
t2099 = t9.*t10.*t13.*t50.*t189.*5.515892039870764e-19;
t2100 = t8.*t14.*t15.*t50.*t189.*5.515892039870764e-19;
t2101 = t9.*t13.*t15.*t50.*t189.*5.515892039870764e-19;
t2102 = t10.*t13.*t14.*t50.*t189.*5.515892039870764e-19;
t2103 = t13.*t14.*t15.*t50.*t189.*5.515892039870764e-19;
t2104 = t8.*t9.*t10.*t50.*t189.*(-3.279367663374749e-19);
t2105 = t13.*t14.*t15.*t50.*t189.*(-3.279367663374749e-19);
t2117 = t18.*t19.*t201.*7.713980286110892e-6;
t2118 = t18.*t25.*t201.*7.713980286110892e-6;
t2119 = t19.*t24.*t201.*7.713980286110892e-6;
t2120 = t24.*t25.*t201.*7.713980286110892e-6;
t2121 = t18.*t19.*t201.*4.586198809426854e-6;
t2122 = t18.*t25.*t201.*4.586198809426854e-6;
t2123 = t19.*t24.*t201.*4.586198809426854e-6;
t2124 = t24.*t25.*t201.*4.586198809426854e-6;
t2131 = t24.*t25.*t201.*1.867830746966542e-4;
t2138 = t18.*t19.*t201.*1.867830746966542e-4;
t2139 = t18.*t25.*t201.*1.867830746966542e-4;
t2140 = t19.*t24.*t201.*1.867830746966542e-4;
t2147 = t18.*t19.*t201.*4.665565775347468e-4;
t2149 = t18.*t25.*t201.*4.665565775347468e-4;
t2150 = t19.*t24.*t201.*4.665565775347468e-4;
t2151 = t18.*t19.*t201.*2.773822515819383e-4;
t2152 = t24.*t25.*t201.*4.665565775347468e-4;
t2153 = t18.*t19.*t201.*3.141688827417478e-4;
t2154 = t18.*t25.*t201.*2.773822515819383e-4;
t2155 = t19.*t24.*t201.*2.773822515819383e-4;
t2156 = t18.*t25.*t201.*3.141688827417478e-4;
t2157 = t19.*t24.*t201.*3.141688827417478e-4;
t2158 = t24.*t25.*t201.*2.773822515819383e-4;
t2159 = t24.*t25.*t201.*3.141688827417478e-4;
t2294 = t10.*t50.*t189.*(t42-t43).*(-7.204296868834178e-35);
t2296 = t15.*t50.*t189.*(t42-t43).*(-7.204296868834178e-35);
t2299 = t10.*t50.*t189.*(t42-t43).*(-7.987216665362745e-37);
t2300 = t10.*t50.*t189.*(t42-t43).*7.204296868834178e-35;
t2302 = t15.*t50.*t189.*(t42-t43).*(-7.987216665362745e-37);
t2303 = t15.*t50.*t189.*(t42-t43).*7.204296868834178e-35;
t2305 = t35.*t50.*t189.*2.492226411042213e-17;
t2306 = t36.*t50.*t189.*2.492226411042213e-17;
t2308 = t35.*t50.*t189.*3.691525655515653e-19;
t2309 = t36.*t50.*t189.*3.691525655515653e-19;
t2310 = t10.*t50.*t189.*(t42-t43).*7.987216665362745e-37;
t2313 = t15.*t50.*t189.*(t42-t43).*(-7.974890713718666e-38);
t2314 = t8.*t9.*t50.*t189.*1.525453217729535e-19;
t2315 = t8.*t14.*t50.*t189.*1.525453217729535e-19;
t2316 = t9.*t13.*t50.*t189.*1.525453217729535e-19;
t2317 = t35.*t50.*t189.*4.191921502353519e-17;
t2318 = t13.*t14.*t50.*t189.*1.525453217729535e-19;
t2319 = t36.*t50.*t189.*4.191921502353519e-17;
t2322 = t35.*t50.*t189.*3.487329940320384e-18;
t2323 = t36.*t50.*t189.*3.487329940320384e-18;
t2324 = t10.*t50.*t189.*(t42-t43).*(-7.974890713718666e-38);
t2325 = t15.*t50.*t189.*(t42-t43).*7.974890713718666e-38;
t2326 = t8.*t9.*t50.*t189.*7.176346641264665e-19;
t2327 = t8.*t14.*t50.*t189.*7.176346641264665e-19;
t2328 = t9.*t13.*t50.*t189.*7.176346641264665e-19;
t2329 = t13.*t14.*t50.*t189.*7.176346641264665e-19;
t2330 = t8.*t9.*t50.*t189.*2.565810279476446e-19;
t2331 = t8.*t14.*t50.*t189.*2.565810279476446e-19;
t2332 = t9.*t13.*t50.*t189.*2.565810279476446e-19;
t2334 = t13.*t14.*t50.*t189.*2.565810279476446e-19;
t2339 = t10.*t50.*t189.*(t42-t43).*7.974890713718666e-38;
t2340 = t50.*t202.*5.701449638003928e-20;
t2345 = t38.*t50.*t202.*2.492226411042213e-17;
t2346 = t39.*t50.*t202.*2.492226411042213e-17;
t2348 = t8.*t9.*t50.*t189.*1.207060548775729e-18;
t2349 = t35.*t50.*t189.*1.89580370025077e-18;
t2352 = t8.*t14.*t50.*t189.*1.207060548775729e-18;
t2353 = t9.*t13.*t50.*t189.*1.207060548775729e-18;
t2354 = t36.*t50.*t189.*1.89580370025077e-18;
t2357 = t13.*t14.*t50.*t189.*1.207060548775729e-18;
t2358 = t38.*t50.*t202.*3.691525655515653e-19;
t2359 = t8.*t9.*t50.*t189.*2.83128614153514e-18;
t2360 = t39.*t50.*t202.*3.691525655515653e-19;
t2361 = t8.*t14.*t50.*t189.*2.83128614153514e-18;
t2362 = t9.*t13.*t50.*t189.*2.83128614153514e-18;
t2364 = t13.*t14.*t50.*t189.*2.83128614153514e-18;
t2365 = t8.*t14.*t50.*t189.*4.762219517228144e-18;
t2366 = t9.*t13.*t50.*t189.*4.762219517228144e-18;
t2367 = t13.*t14.*t50.*t189.*4.762219517228144e-18;
t2374 = t35.*t50.*t189.*5.383133640571155e-18;
t2378 = t36.*t50.*t189.*5.383133640571155e-18;
t2382 = t38.*t50.*t202.*4.191921502353519e-17;
t2383 = t39.*t50.*t202.*4.191921502353519e-17;
t2391 = t38.*t50.*t202.*3.487329940320384e-18;
t2392 = t39.*t50.*t202.*3.487329940320384e-18;
t2393 = t8.*t9.*t50.*t189.*4.762219517228144e-18;
t2402 = t18.*t19.*t50.*t202.*7.176346641264665e-19;
t2404 = t18.*t25.*t50.*t202.*7.176346641264665e-19;
t2405 = t19.*t24.*t50.*t202.*7.176346641264665e-19;
t2406 = t24.*t25.*t50.*t202.*7.176346641264665e-19;
t2407 = t20.*t50.*t202.*3.998903374256319e-23;
t2409 = t21.*t50.*t202.*5.902881824626087e-21;
t2411 = t27.*t50.*t202.*1.294536862550567e-20;
t2415 = t24.*t25.*t50.*t202.*2.83128614153514e-18;
t2416 = t8.*t9.*t15.*t50.*t189.*1.675871243454932e-19;
t2417 = t8.*t14.*t15.*t50.*t189.*1.675871243454932e-19;
t2418 = t9.*t13.*t15.*t50.*t189.*1.675871243454932e-19;
t2420 = t13.*t14.*t15.*t50.*t189.*1.675871243454932e-19;
t2426 = t8.*t9.*t10.*t16.*t50.*t189.*2.773380719257578e-19;
t2427 = t8.*t9.*t10.*t11.*t50.*t189.*3.616047923242029e-19;
t2428 = t18.*t19.*t50.*t202.*1.207060548775729e-18;
t2429 = t8.*t10.*t14.*t16.*t50.*t189.*2.773380719257578e-19;
t2430 = t9.*t10.*t13.*t16.*t50.*t189.*2.773380719257578e-19;
t2431 = t8.*t10.*t11.*t14.*t50.*t189.*3.616047923242029e-19;
t2432 = t9.*t10.*t11.*t13.*t50.*t189.*3.616047923242029e-19;
t2433 = t18.*t25.*t50.*t202.*1.207060548775729e-18;
t2434 = t19.*t24.*t50.*t202.*1.207060548775729e-18;
t2435 = t8.*t9.*t10.*t11.*t50.*t189.*6.082187788323819e-19;
t2436 = t10.*t13.*t14.*t16.*t50.*t189.*2.773380719257578e-19;
t2437 = t10.*t11.*t13.*t14.*t50.*t189.*3.616047923242029e-19;
t2438 = t24.*t25.*t50.*t202.*1.207060548775729e-18;
t2439 = t8.*t9.*t10.*t16.*t50.*t189.*1.648860235700588e-19;
t2440 = t8.*t10.*t11.*t14.*t50.*t189.*6.082187788323819e-19;
t2441 = t9.*t10.*t11.*t13.*t50.*t189.*6.082187788323819e-19;
t2442 = t8.*t10.*t14.*t16.*t50.*t189.*1.648860235700588e-19;
t2443 = t9.*t10.*t13.*t16.*t50.*t189.*1.648860235700588e-19;
t2444 = t10.*t11.*t13.*t14.*t50.*t189.*6.082187788323819e-19;
t2446 = t10.*t13.*t14.*t16.*t50.*t189.*1.648860235700588e-19;
t2447 = t18.*t19.*t50.*t202.*2.83128614153514e-18;
t2448 = t18.*t25.*t50.*t202.*2.83128614153514e-18;
t2449 = t19.*t24.*t50.*t202.*2.83128614153514e-18;
t2451 = t20.*t21.*t50.*t202.*7.696420262413979e-21;
t2452 = t20.*t27.*t50.*t202.*7.696420262413979e-21;
t2453 = t21.*t26.*t50.*t202.*7.696420262413979e-21;
t2454 = t21.*t26.*t50.*t202.*7.69642026241398e-21;
t2455 = t20.*t50.*t202.*3.566935413776081e-21;
t2456 = t18.*t19.*t50.*t202.*4.762219517228144e-18;
t2457 = t26.*t50.*t202.*3.566935413776081e-21;
t2459 = t18.*t25.*t50.*t202.*4.762219517228144e-18;
t2460 = t19.*t24.*t50.*t202.*4.762219517228144e-18;
t2461 = t24.*t25.*t50.*t202.*4.762219517228144e-18;
t2463 = t8.*t9.*t10.*t50.*t189.*1.875925506339668e-22;
t2466 = t8.*t10.*t14.*t50.*t189.*1.875925506339668e-22;
t2467 = t9.*t10.*t13.*t50.*t189.*1.875925506339668e-22;
t2469 = t10.*t13.*t14.*t50.*t189.*1.875925506339668e-22;
t2471 = t38.*t50.*t202.*5.383133640571155e-18;
t2475 = t39.*t50.*t202.*5.383133640571155e-18;
t2482 = t20.*t21.*t50.*t202.*3.509445006623964e-21;
t2483 = t20.*t27.*t50.*t202.*3.509445006623964e-21;
t2484 = t26.*t27.*t50.*t202.*3.509445006623964e-21;
t2485 = t26.*t27.*t50.*t202.*3.509445006623964e-21;
t2486 = t8.*t9.*t15.*t50.*t189.*2.818813198306831e-19;
t2487 = t8.*t14.*t15.*t50.*t189.*2.818813198306831e-19;
t2488 = t9.*t13.*t15.*t50.*t189.*2.818813198306831e-19;
t2491 = t13.*t14.*t15.*t50.*t189.*2.818813198306831e-19;
t2495 = t8.*t9.*t10.*t50.*t189.*3.155304201896394e-22;
t2498 = t8.*t10.*t14.*t50.*t189.*3.155304201896394e-22;
t2499 = t9.*t10.*t13.*t50.*t189.*3.155304201896394e-22;
t2505 = t10.*t13.*t14.*t50.*t189.*3.155304201896394e-22;
t2512 = t20.*t50.*t202.*3.992732227073824e-24;
t2513 = t26.*t50.*t202.*3.992732227073824e-24;
t2515 = t189.*t202.*2.393852475650798e-6;
t2529 = t189.*t202.*2.297802839282093e-6;
t2541 = t18.*t19.*t21.*t26.*t50.*t202.*3.509445006623964e-21;
t2544 = t18.*t21.*t25.*t26.*t50.*t202.*3.509445006623964e-21;
t2546 = t19.*t21.*t24.*t26.*t50.*t202.*3.509445006623964e-21;
t2551 = t21.*t24.*t25.*t26.*t50.*t202.*3.509445006623964e-21;
t2560 = t18.*t19.*t26.*t27.*t50.*t202.*7.696420262413979e-21;
t2567 = t18.*t25.*t26.*t27.*t50.*t202.*7.696420262413979e-21;
t2568 = t19.*t24.*t26.*t27.*t50.*t202.*7.696420262413979e-21;
t2573 = t24.*t25.*t26.*t27.*t50.*t202.*7.696420262413979e-21;
t2577 = t18.*t19.*t20.*t27.*t50.*t202.*(-3.509445006623964e-21);
t2579 = t18.*t20.*t25.*t27.*t50.*t202.*(-3.509445006623964e-21);
t2581 = t19.*t20.*t24.*t27.*t50.*t202.*(-3.509445006623964e-21);
t2586 = t18.*t19.*t20.*t27.*t50.*t202.*5.902881824626087e-21;
t2587 = t18.*t19.*t21.*t26.*t50.*t202.*5.902881824626087e-21;
t2588 = t18.*t19.*t20.*t21.*t50.*t202.*1.294536862550567e-20;
t2593 = t18.*t19.*t26.*t27.*t50.*t202.*5.902881824626087e-21;
t2594 = t18.*t20.*t25.*t27.*t50.*t202.*5.902881824626087e-21;
t2595 = t18.*t21.*t25.*t26.*t50.*t202.*5.902881824626087e-21;
t2596 = t19.*t20.*t24.*t27.*t50.*t202.*5.902881824626087e-21;
t2597 = t19.*t21.*t24.*t26.*t50.*t202.*5.902881824626087e-21;
t2599 = t18.*t19.*t21.*t26.*t50.*t202.*1.294536862550567e-20;
t2600 = t18.*t20.*t21.*t25.*t50.*t202.*1.294536862550567e-20;
t2601 = t19.*t20.*t21.*t24.*t50.*t202.*1.294536862550567e-20;
t2603 = t24.*t25.*t26.*t27.*t50.*t202.*(-3.509445006623964e-21);
t2605 = t18.*t25.*t26.*t27.*t50.*t202.*5.902881824626087e-21;
t2606 = t19.*t24.*t26.*t27.*t50.*t202.*5.902881824626087e-21;
t2607 = t20.*t24.*t25.*t27.*t50.*t202.*5.902881824626087e-21;
t2608 = t21.*t24.*t25.*t26.*t50.*t202.*5.902881824626087e-21;
t2609 = t18.*t19.*t20.*t50.*t202.*5.999580612847032e-21;
t2610 = t18.*t19.*t21.*t26.*t50.*t202.*(-7.696420262413979e-21);
t2611 = t18.*t19.*t26.*t27.*t50.*t202.*1.294536862550567e-20;
t2612 = t18.*t21.*t25.*t26.*t50.*t202.*1.294536862550567e-20;
t2613 = t19.*t21.*t24.*t26.*t50.*t202.*1.294536862550567e-20;
t2614 = t20.*t21.*t24.*t25.*t50.*t202.*1.294536862550567e-20;
t2616 = t24.*t25.*t26.*t27.*t50.*t202.*5.902881824626087e-21;
t2617 = t18.*t19.*t26.*t50.*t202.*5.999580612847032e-21;
t2618 = t18.*t20.*t25.*t50.*t202.*5.999580612847032e-21;
t2619 = t19.*t20.*t24.*t50.*t202.*5.999580612847032e-21;
t2620 = t18.*t21.*t25.*t26.*t50.*t202.*(-7.696420262413979e-21);
t2621 = t19.*t21.*t24.*t26.*t50.*t202.*(-7.696420262413979e-21);
t2622 = t20.*t21.*t24.*t25.*t50.*t202.*(-7.696420262413979e-21);
t2623 = t18.*t25.*t26.*t27.*t50.*t202.*1.294536862550567e-20;
t2624 = t19.*t24.*t26.*t27.*t50.*t202.*1.294536862550567e-20;
tau_c = ft_3({dq1,dq2,dq3,dq4,dq5,dq6,t10,t100,t1000,t1001,t1002,t1003,t1006,t1008,t101,t1019,t102,t103,t1030,t1035,t1039,t104,t1044,t1047,t1049,t1055,t1058,t106,t1065,t1066,t1067,t107,t1070,t1071,t108,t1080,t1083,t1084,t1089,t109,t1092,t11,t110,t1104,t1105,t1108,t111,t1110,t1112,t1113,t1114,t1115,t112,t1121,t1123,t1124,t1126,t113,t1137,t114,t1145,t1148,t115,t1150,t1154,t1158,t1159,t1162,t1166,t1167,t117,t1170,t1176,t1177,t1178,t1179,t118,t1180,t1184,t1185,t1189,t1190,t1192,t1193,t1194,t1196,t1197,t1198,t1199,t12,t120,t1202,t1203,t1204,t1205,t1207,t1208,t121,t1210,t1212,t1214,t1217,t1218,t1219,t122,t1220,t1221,t1222,t1223,t1229,t123,t1230,t1232,t1234,t1235,t1236,t1237,t1238,t124,t1242,t1246,t1247,t1248,t125,t1252,t1253,t1254,t1255,t1256,t126,t1265,t1267,t1269,t127,t1277,t1278,t128,t1280,t1285,t1286,t1287,t1288,t1289,t129,t1290,t1291,t1292,t1294,t1295,t1297,t1298,t1299,t13,t130,t1300,t1301,t1302,t1303,t1305,t1307,t1311,t1316,t1317,t1319,t132,t1320,t1322,t1323,t1324,t1327,t1328,t1329,t133,t1334,t1335,t1336,t1337,t1338,t134,t1342,t1343,t1344,t1345,t1348,t1349,t135,t1350,t1351,t1352,t1354,t136,t1360,t1366,t1367,t1368,t1369,t137,t1370,t1371,t1373,t1374,t1375,t1376,t1378,t1379,t138,t1380,t1385,t1386,t1387,t1389,t139,t1392,t1393,t1394,t1395,t1396,t1397,t1398,t1399,t14,t1404,t1405,t1406,t1407,t1408,t1409,t1410,t1411,t1412,t1413,t1414,t1415,t1416,t1417,t1419,t1420,t1421,t1424,t1425,t1427,t1428,t1429,t1430,t1433,t1434,t1435,t1436,t144,t1440,t1441,t1443,t1445,t1446,t1447,t1448,t145,t1454,t1455,t1456,t1458,t146,t147,t1470,t1473,t1474,t1475,t1477,t1478,t148,t1480,t1481,t1483,t1488,t149,t1490,t1491,t1492,t1493,t1496,t1497,t1498,t15,t150,t1500,t1501,t1503,t1509,t151,t1511,t1513,t1514,t1515,t1517,t1518,t1519,t152,t1520,t1521,t1523,t1524,t1528,t153,t1530,t1537,t1538,t1539,t1541,t1542,t1545,t1546,t156,t1560,t1561,t1562,t1563,t1566,t1567,t157,t1570,t1571,t1573,t1576,t1577,t1578,t158,t1581,t1582,t1584,t1585,t1586,t1587,t1589,t1590,t1591,t1593,t16,t160,t1607,t1608,t1609,t161,t1611,t1614,t1615,t1616,t1617,t162,t1621,t1623,t1624,t1625,t163,t1638,t164,t1648,t1649,t165,t166,t1660,t167,t168,t1686,t1688,t1689,t169,t1690,t1695,t17,t170,t1700,t1701,t1702,t171,t172,t173,t174,t175,t1750,t176,t1765,t177,t178,t1780,t1782,t1795,t1796,t1797,t1798,t18,t180,t1807,t181,t1817,t182,t185,t186,t1865,t1868,t1870,t1871,t1872,t1873,t1874,t1875,t1876,t1877,t1879,t188,t1880,t1881,t1882,t1883,t1884,t1886,t1887,t1889,t189,t1890,t1891,t1894,t1895,t1897,t1898,t1899,t19,t190,t1901,t1902,t1903,t1904,t1907,t1909,t191,t1914,t1915,t1916,t1917,t1919,t192,t1920,t1922,t1923,t1924,t1925,t1926,t1927,t1928,t1929,t1930,t1931,t1936,t1937,t1940,t1941,t1942,t1943,t1947,t1948,t1949,t195,t1950,t1951,t1952,t1953,t1956,t1958,t1959,t196,t1960,t1961,t1965,t1966,t1967,t1968,t197,t1970,t1971,t1975,t1977,t198,t1982,t1991,t1997,t20,t201,t2017,t202,t2021,t2022,t2024,t2025,t2027,t2028,t2029,t203,t2030,t2032,t2034,t2035,t2038,t2039,t204,t2043,t2044,t2045,t2049,t205,t2050,t2051,t2052,t2054,t2055,t2056,t2057,t2058,t2059,t2061,t2062,t2063,t2069,t207,t2075,t2077,t208,t2080,t2081,t2082,t2083,t2084,t2085,t2086,t2087,t2088,t2089,t209,t2090,t2091,t2092,t2093,t2096,t2097,t2098,t2099,t21,t210,t2100,t2101,t2102,t2103,t2104,t2105,t211,t2117,t2118,t2119,t212,t2120,t2121,t2122,t2123,t2124,t2131,t2138,t2139,t2140,t2147,t2149,t2150,t2151,t2152,t2153,t2154,t2155,t2156,t2157,t2158,t2159,t216,t217,t218,t219,t22,t220,t221,t223,t224,t225,t226,t227,t229,t2294,t2296,t2299,t230,t2300,t2302,t2303,t2305,t2306,t2308,t2309,t231,t2310,t2313,t2314,t2315,t2316,t2317,t2318,t2319,t2322,t2323,t2324,t2325,t2326,t2327,t2328,t2329,t233,t2330,t2331,t2332,t2334,t2339,t2340,t2345,t2346,t2348,t2349,t2352,t2353,t2354,t2357,t2358,t2359,t236,t2360,t2361,t2362,t2364,t2365,t2366,t2367,t237,t2374,t2378,t238,t2382,t2383,t239,t2391,t2392,t2393,t24,t240,t2402,t2404,t2405,t2406,t2407,t2409,t241,t2411,t2415,t2416,t2417,t2418,t242,t2420,t2426,t2427,t2428,t2429,t243,t2430,t2431,t2432,t2433,t2434,t2435,t2436,t2437,t2438,t2439,t244,t2440,t2441,t2442,t2443,t2444,t2446,t2447,t2448,t2449,t245,t2451,t2452,t2453,t2454,t2455,t2456,t2457,t2459,t246,t2460,t2461,t2463,t2466,t2467,t2469,t247,t2471,t2475,t2482,t2483,t2484,t2485,t2486,t2487,t2488,t2491,t2495,t2498,t2499,t25,t250,t2505,t251,t2512,t2513,t2515,t252,t2529,t2541,t2544,t2546,t255,t2551,t256,t2560,t2567,t2568,t257,t2573,t2577,t2579,t258,t2581,t2586,t2587,t2588,t259,t2593,t2594,t2595,t2596,t2597,t2599,t26,t260,t2600,t2601,t2603,t2605,t2606,t2607,t2608,t2609,t261,t2610,t2611,t2612,t2613,t2614,t2616,t2617,t2618,t2619,t262,t2620,t2621,t2622,t2623,t2624,t263,t264,t265,t266,t267,t269,t27,t270,t271,t272,t273,t274,t275,t276,t277,t279,t28,t280,t281,t282,t283,t285,t286,t289,t29,t293,t294,t295,t296,t297,t298,t299,t30,t301,t302,t303,t304,t305,t306,t307,t308,t309,t31,t310,t311,t312,t313,t314,t315,t316,t318,t319,t32,t320,t321,t322,t323,t324,t325,t326,t328,t329,t33,t330,t331,t332,t333,t338,t339,t34,t340,t341,t342,t343,t344,t345,t346,t348,t349,t35,t350,t355,t358,t359,t36,t360,t363,t364,t365,t366,t368,t369,t370,t371,t372,t373,t374,t376,t377,t378,t38,t381,t382,t384,t385,t386,t388,t389,t39,t390,t391,t392,t393,t396,t397,t398,t403,t404,t405,t406,t407,t408,t410,t411,t412,t413,t414,t415,t419,t42,t420,t421,t422,t423,t424,t425,t426,t427,t428,t43,t430,t431,t432,t433,t434,t435,t437,t438,t439,t44,t440,t441,t442,t444,t445,t446,t448,t45,t451,t452,t455,t456,t457,t458,t459,t46,t460,t461,t462,t463,t464,t465,t466,t467,t468,t469,t47,t470,t471,t472,t473,t474,t475,t476,t477,t478,t479,t48,t480,t483,t485,t486,t487,t488,t489,t490,t491,t492,t493,t494,t495,t496,t497,t498,t499,t50,t500,t501,t502,t503,t504,t505,t506,t507,t508,t509,t51,t510,t511,t514,t515,t516,t519,t52,t520,t521,t522,t528,t53,t531,t532,t533,t537,t54,t545,t547,t548,t550,t553,t554,t555,t557,t559,t56,t560,t561,t562,t566,t568,t57,t570,t58,t582,t583,t584,t585,t589,t59,t590,t591,t592,t595,t597,t599,t60,t600,t601,t605,t606,t607,t608,t609,t619,t620,t621,t622,t628,t63,t635,t636,t638,t64,t640,t641,t642,t643,t645,t646,t648,t649,t65,t654,t655,t656,t657,t659,t660,t663,t664,t665,t666,t667,t668,t669,t67,t670,t672,t673,t674,t675,t676,t677,t678,t679,t68,t681,t682,t683,t684,t685,t686,t687,t689,t69,t691,t692,t693,t694,t70,t702,t704,t705,t707,t708,t71,t710,t711,t712,t713,t714,t715,t716,t717,t718,t719,t72,t720,t721,t722,t723,t724,t725,t726,t728,t73,t736,t738,t740,t741,t742,t743,t744,t745,t746,t747,t749,t75,t750,t751,t755,t756,t757,t758,t759,t76,t762,t763,t764,t766,t768,t77,t770,t771,t772,t773,t774,t775,t776,t777,t778,t78,t781,t782,t783,t784,t785,t786,t787,t789,t79,t790,t791,t792,t793,t794,t796,t797,t798,t799,t8,t80,t800,t801,t802,t806,t807,t808,t809,t81,t812,t813,t816,t817,t818,t819,t82,t820,t821,t822,t823,t824,t825,t826,t827,t828,t829,t830,t831,t832,t833,t836,t837,t838,t839,t84,t840,t841,t844,t845,t846,t85,t850,t851,t852,t853,t854,t855,t857,t86,t860,t861,t863,t864,t866,t867,t869,t874,t875,t876,t877,t878,t882,t883,t887,t889,t89,t890,t896,t897,t898,t9,t90,t900,t901,t902,t903,t904,t905,t906,t908,t909,t91,t913,t92,t920,t921,t923,t924,t929,t93,t938,t939,t94,t946,t95,t952,t954,t956,t957,t96,t963,t964,t97,t972,t975,t977,t98,t983,t986,t988,t99,t996,t998});
end
function tau_c = ft_3(ct)
dq1 = ct{1};
dq2 = ct{2};
dq3 = ct{3};
dq4 = ct{4};
dq5 = ct{5};
dq6 = ct{6};
t10 = ct{7};
t100 = ct{8};
t1000 = ct{9};
t1001 = ct{10};
t1002 = ct{11};
t1003 = ct{12};
t1006 = ct{13};
t1008 = ct{14};
t101 = ct{15};
t1019 = ct{16};
t102 = ct{17};
t103 = ct{18};
t1030 = ct{19};
t1035 = ct{20};
t1039 = ct{21};
t104 = ct{22};
t1044 = ct{23};
t1047 = ct{24};
t1049 = ct{25};
t1055 = ct{26};
t1058 = ct{27};
t106 = ct{28};
t1065 = ct{29};
t1066 = ct{30};
t1067 = ct{31};
t107 = ct{32};
t1070 = ct{33};
t1071 = ct{34};
t108 = ct{35};
t1080 = ct{36};
t1083 = ct{37};
t1084 = ct{38};
t1089 = ct{39};
t109 = ct{40};
t1092 = ct{41};
t11 = ct{42};
t110 = ct{43};
t1104 = ct{44};
t1105 = ct{45};
t1108 = ct{46};
t111 = ct{47};
t1110 = ct{48};
t1112 = ct{49};
t1113 = ct{50};
t1114 = ct{51};
t1115 = ct{52};
t112 = ct{53};
t1121 = ct{54};
t1123 = ct{55};
t1124 = ct{56};
t1126 = ct{57};
t113 = ct{58};
t1137 = ct{59};
t114 = ct{60};
t1145 = ct{61};
t1148 = ct{62};
t115 = ct{63};
t1150 = ct{64};
t1154 = ct{65};
t1158 = ct{66};
t1159 = ct{67};
t1162 = ct{68};
t1166 = ct{69};
t1167 = ct{70};
t117 = ct{71};
t1170 = ct{72};
t1176 = ct{73};
t1177 = ct{74};
t1178 = ct{75};
t1179 = ct{76};
t118 = ct{77};
t1180 = ct{78};
t1184 = ct{79};
t1185 = ct{80};
t1189 = ct{81};
t1190 = ct{82};
t1192 = ct{83};
t1193 = ct{84};
t1194 = ct{85};
t1196 = ct{86};
t1197 = ct{87};
t1198 = ct{88};
t1199 = ct{89};
t12 = ct{90};
t120 = ct{91};
t1202 = ct{92};
t1203 = ct{93};
t1204 = ct{94};
t1205 = ct{95};
t1207 = ct{96};
t1208 = ct{97};
t121 = ct{98};
t1210 = ct{99};
t1212 = ct{100};
t1214 = ct{101};
t1217 = ct{102};
t1218 = ct{103};
t1219 = ct{104};
t122 = ct{105};
t1220 = ct{106};
t1221 = ct{107};
t1222 = ct{108};
t1223 = ct{109};
t1229 = ct{110};
t123 = ct{111};
t1230 = ct{112};
t1232 = ct{113};
t1234 = ct{114};
t1235 = ct{115};
t1236 = ct{116};
t1237 = ct{117};
t1238 = ct{118};
t124 = ct{119};
t1242 = ct{120};
t1246 = ct{121};
t1247 = ct{122};
t1248 = ct{123};
t125 = ct{124};
t1252 = ct{125};
t1253 = ct{126};
t1254 = ct{127};
t1255 = ct{128};
t1256 = ct{129};
t126 = ct{130};
t1265 = ct{131};
t1267 = ct{132};
t1269 = ct{133};
t127 = ct{134};
t1277 = ct{135};
t1278 = ct{136};
t128 = ct{137};
t1280 = ct{138};
t1285 = ct{139};
t1286 = ct{140};
t1287 = ct{141};
t1288 = ct{142};
t1289 = ct{143};
t129 = ct{144};
t1290 = ct{145};
t1291 = ct{146};
t1292 = ct{147};
t1294 = ct{148};
t1295 = ct{149};
t1297 = ct{150};
t1298 = ct{151};
t1299 = ct{152};
t13 = ct{153};
t130 = ct{154};
t1300 = ct{155};
t1301 = ct{156};
t1302 = ct{157};
t1303 = ct{158};
t1305 = ct{159};
t1307 = ct{160};
t1311 = ct{161};
t1316 = ct{162};
t1317 = ct{163};
t1319 = ct{164};
t132 = ct{165};
t1320 = ct{166};
t1322 = ct{167};
t1323 = ct{168};
t1324 = ct{169};
t1327 = ct{170};
t1328 = ct{171};
t1329 = ct{172};
t133 = ct{173};
t1334 = ct{174};
t1335 = ct{175};
t1336 = ct{176};
t1337 = ct{177};
t1338 = ct{178};
t134 = ct{179};
t1342 = ct{180};
t1343 = ct{181};
t1344 = ct{182};
t1345 = ct{183};
t1348 = ct{184};
t1349 = ct{185};
t135 = ct{186};
t1350 = ct{187};
t1351 = ct{188};
t1352 = ct{189};
t1354 = ct{190};
t136 = ct{191};
t1360 = ct{192};
t1366 = ct{193};
t1367 = ct{194};
t1368 = ct{195};
t1369 = ct{196};
t137 = ct{197};
t1370 = ct{198};
t1371 = ct{199};
t1373 = ct{200};
t1374 = ct{201};
t1375 = ct{202};
t1376 = ct{203};
t1378 = ct{204};
t1379 = ct{205};
t138 = ct{206};
t1380 = ct{207};
t1385 = ct{208};
t1386 = ct{209};
t1387 = ct{210};
t1389 = ct{211};
t139 = ct{212};
t1392 = ct{213};
t1393 = ct{214};
t1394 = ct{215};
t1395 = ct{216};
t1396 = ct{217};
t1397 = ct{218};
t1398 = ct{219};
t1399 = ct{220};
t14 = ct{221};
t1404 = ct{222};
t1405 = ct{223};
t1406 = ct{224};
t1407 = ct{225};
t1408 = ct{226};
t1409 = ct{227};
t1410 = ct{228};
t1411 = ct{229};
t1412 = ct{230};
t1413 = ct{231};
t1414 = ct{232};
t1415 = ct{233};
t1416 = ct{234};
t1417 = ct{235};
t1419 = ct{236};
t1420 = ct{237};
t1421 = ct{238};
t1424 = ct{239};
t1425 = ct{240};
t1427 = ct{241};
t1428 = ct{242};
t1429 = ct{243};
t1430 = ct{244};
t1433 = ct{245};
t1434 = ct{246};
t1435 = ct{247};
t1436 = ct{248};
t144 = ct{249};
t1440 = ct{250};
t1441 = ct{251};
t1443 = ct{252};
t1445 = ct{253};
t1446 = ct{254};
t1447 = ct{255};
t1448 = ct{256};
t145 = ct{257};
t1454 = ct{258};
t1455 = ct{259};
t1456 = ct{260};
t1458 = ct{261};
t146 = ct{262};
t147 = ct{263};
t1470 = ct{264};
t1473 = ct{265};
t1474 = ct{266};
t1475 = ct{267};
t1477 = ct{268};
t1478 = ct{269};
t148 = ct{270};
t1480 = ct{271};
t1481 = ct{272};
t1483 = ct{273};
t1488 = ct{274};
t149 = ct{275};
t1490 = ct{276};
t1491 = ct{277};
t1492 = ct{278};
t1493 = ct{279};
t1496 = ct{280};
t1497 = ct{281};
t1498 = ct{282};
t15 = ct{283};
t150 = ct{284};
t1500 = ct{285};
t1501 = ct{286};
t1503 = ct{287};
t1509 = ct{288};
t151 = ct{289};
t1511 = ct{290};
t1513 = ct{291};
t1514 = ct{292};
t1515 = ct{293};
t1517 = ct{294};
t1518 = ct{295};
t1519 = ct{296};
t152 = ct{297};
t1520 = ct{298};
t1521 = ct{299};
t1523 = ct{300};
t1524 = ct{301};
t1528 = ct{302};
t153 = ct{303};
t1530 = ct{304};
t1537 = ct{305};
t1538 = ct{306};
t1539 = ct{307};
t1541 = ct{308};
t1542 = ct{309};
t1545 = ct{310};
t1546 = ct{311};
t156 = ct{312};
t1560 = ct{313};
t1561 = ct{314};
t1562 = ct{315};
t1563 = ct{316};
t1566 = ct{317};
t1567 = ct{318};
t157 = ct{319};
t1570 = ct{320};
t1571 = ct{321};
t1573 = ct{322};
t1576 = ct{323};
t1577 = ct{324};
t1578 = ct{325};
t158 = ct{326};
t1581 = ct{327};
t1582 = ct{328};
t1584 = ct{329};
t1585 = ct{330};
t1586 = ct{331};
t1587 = ct{332};
t1589 = ct{333};
t1590 = ct{334};
t1591 = ct{335};
t1593 = ct{336};
t16 = ct{337};
t160 = ct{338};
t1607 = ct{339};
t1608 = ct{340};
t1609 = ct{341};
t161 = ct{342};
t1611 = ct{343};
t1614 = ct{344};
t1615 = ct{345};
t1616 = ct{346};
t1617 = ct{347};
t162 = ct{348};
t1621 = ct{349};
t1623 = ct{350};
t1624 = ct{351};
t1625 = ct{352};
t163 = ct{353};
t1638 = ct{354};
t164 = ct{355};
t1648 = ct{356};
t1649 = ct{357};
t165 = ct{358};
t166 = ct{359};
t1660 = ct{360};
t167 = ct{361};
t168 = ct{362};
t1686 = ct{363};
t1688 = ct{364};
t1689 = ct{365};
t169 = ct{366};
t1690 = ct{367};
t1695 = ct{368};
t17 = ct{369};
t170 = ct{370};
t1700 = ct{371};
t1701 = ct{372};
t1702 = ct{373};
t171 = ct{374};
t172 = ct{375};
t173 = ct{376};
t174 = ct{377};
t175 = ct{378};
t1750 = ct{379};
t176 = ct{380};
t1765 = ct{381};
t177 = ct{382};
t178 = ct{383};
t1780 = ct{384};
t1782 = ct{385};
t1795 = ct{386};
t1796 = ct{387};
t1797 = ct{388};
t1798 = ct{389};
t18 = ct{390};
t180 = ct{391};
t1807 = ct{392};
t181 = ct{393};
t1817 = ct{394};
t182 = ct{395};
t185 = ct{396};
t186 = ct{397};
t1865 = ct{398};
t1868 = ct{399};
t1870 = ct{400};
t1871 = ct{401};
t1872 = ct{402};
t1873 = ct{403};
t1874 = ct{404};
t1875 = ct{405};
t1876 = ct{406};
t1877 = ct{407};
t1879 = ct{408};
t188 = ct{409};
t1880 = ct{410};
t1881 = ct{411};
t1882 = ct{412};
t1883 = ct{413};
t1884 = ct{414};
t1886 = ct{415};
t1887 = ct{416};
t1889 = ct{417};
t189 = ct{418};
t1890 = ct{419};
t1891 = ct{420};
t1894 = ct{421};
t1895 = ct{422};
t1897 = ct{423};
t1898 = ct{424};
t1899 = ct{425};
t19 = ct{426};
t190 = ct{427};
t1901 = ct{428};
t1902 = ct{429};
t1903 = ct{430};
t1904 = ct{431};
t1907 = ct{432};
t1909 = ct{433};
t191 = ct{434};
t1914 = ct{435};
t1915 = ct{436};
t1916 = ct{437};
t1917 = ct{438};
t1919 = ct{439};
t192 = ct{440};
t1920 = ct{441};
t1922 = ct{442};
t1923 = ct{443};
t1924 = ct{444};
t1925 = ct{445};
t1926 = ct{446};
t1927 = ct{447};
t1928 = ct{448};
t1929 = ct{449};
t1930 = ct{450};
t1931 = ct{451};
t1936 = ct{452};
t1937 = ct{453};
t1940 = ct{454};
t1941 = ct{455};
t1942 = ct{456};
t1943 = ct{457};
t1947 = ct{458};
t1948 = ct{459};
t1949 = ct{460};
t195 = ct{461};
t1950 = ct{462};
t1951 = ct{463};
t1952 = ct{464};
t1953 = ct{465};
t1956 = ct{466};
t1958 = ct{467};
t1959 = ct{468};
t196 = ct{469};
t1960 = ct{470};
t1961 = ct{471};
t1965 = ct{472};
t1966 = ct{473};
t1967 = ct{474};
t1968 = ct{475};
t197 = ct{476};
t1970 = ct{477};
t1971 = ct{478};
t1975 = ct{479};
t1977 = ct{480};
t198 = ct{481};
t1982 = ct{482};
t1991 = ct{483};
t1997 = ct{484};
t20 = ct{485};
t201 = ct{486};
t2017 = ct{487};
t202 = ct{488};
t2021 = ct{489};
t2022 = ct{490};
t2024 = ct{491};
t2025 = ct{492};
t2027 = ct{493};
t2028 = ct{494};
t2029 = ct{495};
t203 = ct{496};
t2030 = ct{497};
t2032 = ct{498};
t2034 = ct{499};
t2035 = ct{500};
t2038 = ct{501};
t2039 = ct{502};
t204 = ct{503};
t2043 = ct{504};
t2044 = ct{505};
t2045 = ct{506};
t2049 = ct{507};
t205 = ct{508};
t2050 = ct{509};
t2051 = ct{510};
t2052 = ct{511};
t2054 = ct{512};
t2055 = ct{513};
t2056 = ct{514};
t2057 = ct{515};
t2058 = ct{516};
t2059 = ct{517};
t2061 = ct{518};
t2062 = ct{519};
t2063 = ct{520};
t2069 = ct{521};
t207 = ct{522};
t2075 = ct{523};
t2077 = ct{524};
t208 = ct{525};
t2080 = ct{526};
t2081 = ct{527};
t2082 = ct{528};
t2083 = ct{529};
t2084 = ct{530};
t2085 = ct{531};
t2086 = ct{532};
t2087 = ct{533};
t2088 = ct{534};
t2089 = ct{535};
t209 = ct{536};
t2090 = ct{537};
t2091 = ct{538};
t2092 = ct{539};
t2093 = ct{540};
t2096 = ct{541};
t2097 = ct{542};
t2098 = ct{543};
t2099 = ct{544};
t21 = ct{545};
t210 = ct{546};
t2100 = ct{547};
t2101 = ct{548};
t2102 = ct{549};
t2103 = ct{550};
t2104 = ct{551};
t2105 = ct{552};
t211 = ct{553};
t2117 = ct{554};
t2118 = ct{555};
t2119 = ct{556};
t212 = ct{557};
t2120 = ct{558};
t2121 = ct{559};
t2122 = ct{560};
t2123 = ct{561};
t2124 = ct{562};
t2131 = ct{563};
t2138 = ct{564};
t2139 = ct{565};
t2140 = ct{566};
t2147 = ct{567};
t2149 = ct{568};
t2150 = ct{569};
t2151 = ct{570};
t2152 = ct{571};
t2153 = ct{572};
t2154 = ct{573};
t2155 = ct{574};
t2156 = ct{575};
t2157 = ct{576};
t2158 = ct{577};
t2159 = ct{578};
t216 = ct{579};
t217 = ct{580};
t218 = ct{581};
t219 = ct{582};
t22 = ct{583};
t220 = ct{584};
t221 = ct{585};
t223 = ct{586};
t224 = ct{587};
t225 = ct{588};
t226 = ct{589};
t227 = ct{590};
t229 = ct{591};
t2294 = ct{592};
t2296 = ct{593};
t2299 = ct{594};
t230 = ct{595};
t2300 = ct{596};
t2302 = ct{597};
t2303 = ct{598};
t2305 = ct{599};
t2306 = ct{600};
t2308 = ct{601};
t2309 = ct{602};
t231 = ct{603};
t2310 = ct{604};
t2313 = ct{605};
t2314 = ct{606};
t2315 = ct{607};
t2316 = ct{608};
t2317 = ct{609};
t2318 = ct{610};
t2319 = ct{611};
t2322 = ct{612};
t2323 = ct{613};
t2324 = ct{614};
t2325 = ct{615};
t2326 = ct{616};
t2327 = ct{617};
t2328 = ct{618};
t2329 = ct{619};
t233 = ct{620};
t2330 = ct{621};
t2331 = ct{622};
t2332 = ct{623};
t2334 = ct{624};
t2339 = ct{625};
t2340 = ct{626};
t2345 = ct{627};
t2346 = ct{628};
t2348 = ct{629};
t2349 = ct{630};
t2352 = ct{631};
t2353 = ct{632};
t2354 = ct{633};
t2357 = ct{634};
t2358 = ct{635};
t2359 = ct{636};
t236 = ct{637};
t2360 = ct{638};
t2361 = ct{639};
t2362 = ct{640};
t2364 = ct{641};
t2365 = ct{642};
t2366 = ct{643};
t2367 = ct{644};
t237 = ct{645};
t2374 = ct{646};
t2378 = ct{647};
t238 = ct{648};
t2382 = ct{649};
t2383 = ct{650};
t239 = ct{651};
t2391 = ct{652};
t2392 = ct{653};
t2393 = ct{654};
t24 = ct{655};
t240 = ct{656};
t2402 = ct{657};
t2404 = ct{658};
t2405 = ct{659};
t2406 = ct{660};
t2407 = ct{661};
t2409 = ct{662};
t241 = ct{663};
t2411 = ct{664};
t2415 = ct{665};
t2416 = ct{666};
t2417 = ct{667};
t2418 = ct{668};
t242 = ct{669};
t2420 = ct{670};
t2426 = ct{671};
t2427 = ct{672};
t2428 = ct{673};
t2429 = ct{674};
t243 = ct{675};
t2430 = ct{676};
t2431 = ct{677};
t2432 = ct{678};
t2433 = ct{679};
t2434 = ct{680};
t2435 = ct{681};
t2436 = ct{682};
t2437 = ct{683};
t2438 = ct{684};
t2439 = ct{685};
t244 = ct{686};
t2440 = ct{687};
t2441 = ct{688};
t2442 = ct{689};
t2443 = ct{690};
t2444 = ct{691};
t2446 = ct{692};
t2447 = ct{693};
t2448 = ct{694};
t2449 = ct{695};
t245 = ct{696};
t2451 = ct{697};
t2452 = ct{698};
t2453 = ct{699};
t2454 = ct{700};
t2455 = ct{701};
t2456 = ct{702};
t2457 = ct{703};
t2459 = ct{704};
t246 = ct{705};
t2460 = ct{706};
t2461 = ct{707};
t2463 = ct{708};
t2466 = ct{709};
t2467 = ct{710};
t2469 = ct{711};
t247 = ct{712};
t2471 = ct{713};
t2475 = ct{714};
t2482 = ct{715};
t2483 = ct{716};
t2484 = ct{717};
t2485 = ct{718};
t2486 = ct{719};
t2487 = ct{720};
t2488 = ct{721};
t2491 = ct{722};
t2495 = ct{723};
t2498 = ct{724};
t2499 = ct{725};
t25 = ct{726};
t250 = ct{727};
t2505 = ct{728};
t251 = ct{729};
t2512 = ct{730};
t2513 = ct{731};
t2515 = ct{732};
t252 = ct{733};
t2529 = ct{734};
t2541 = ct{735};
t2544 = ct{736};
t2546 = ct{737};
t255 = ct{738};
t2551 = ct{739};
t256 = ct{740};
t2560 = ct{741};
t2567 = ct{742};
t2568 = ct{743};
t257 = ct{744};
t2573 = ct{745};
t2577 = ct{746};
t2579 = ct{747};
t258 = ct{748};
t2581 = ct{749};
t2586 = ct{750};
t2587 = ct{751};
t2588 = ct{752};
t259 = ct{753};
t2593 = ct{754};
t2594 = ct{755};
t2595 = ct{756};
t2596 = ct{757};
t2597 = ct{758};
t2599 = ct{759};
t26 = ct{760};
t260 = ct{761};
t2600 = ct{762};
t2601 = ct{763};
t2603 = ct{764};
t2605 = ct{765};
t2606 = ct{766};
t2607 = ct{767};
t2608 = ct{768};
t2609 = ct{769};
t261 = ct{770};
t2610 = ct{771};
t2611 = ct{772};
t2612 = ct{773};
t2613 = ct{774};
t2614 = ct{775};
t2616 = ct{776};
t2617 = ct{777};
t2618 = ct{778};
t2619 = ct{779};
t262 = ct{780};
t2620 = ct{781};
t2621 = ct{782};
t2622 = ct{783};
t2623 = ct{784};
t2624 = ct{785};
t263 = ct{786};
t264 = ct{787};
t265 = ct{788};
t266 = ct{789};
t267 = ct{790};
t269 = ct{791};
t27 = ct{792};
t270 = ct{793};
t271 = ct{794};
t272 = ct{795};
t273 = ct{796};
t274 = ct{797};
t275 = ct{798};
t276 = ct{799};
t277 = ct{800};
t279 = ct{801};
t28 = ct{802};
t280 = ct{803};
t281 = ct{804};
t282 = ct{805};
t283 = ct{806};
t285 = ct{807};
t286 = ct{808};
t289 = ct{809};
t29 = ct{810};
t293 = ct{811};
t294 = ct{812};
t295 = ct{813};
t296 = ct{814};
t297 = ct{815};
t298 = ct{816};
t299 = ct{817};
t30 = ct{818};
t301 = ct{819};
t302 = ct{820};
t303 = ct{821};
t304 = ct{822};
t305 = ct{823};
t306 = ct{824};
t307 = ct{825};
t308 = ct{826};
t309 = ct{827};
t31 = ct{828};
t310 = ct{829};
t311 = ct{830};
t312 = ct{831};
t313 = ct{832};
t314 = ct{833};
t315 = ct{834};
t316 = ct{835};
t318 = ct{836};
t319 = ct{837};
t32 = ct{838};
t320 = ct{839};
t321 = ct{840};
t322 = ct{841};
t323 = ct{842};
t324 = ct{843};
t325 = ct{844};
t326 = ct{845};
t328 = ct{846};
t329 = ct{847};
t33 = ct{848};
t330 = ct{849};
t331 = ct{850};
t332 = ct{851};
t333 = ct{852};
t338 = ct{853};
t339 = ct{854};
t34 = ct{855};
t340 = ct{856};
t341 = ct{857};
t342 = ct{858};
t343 = ct{859};
t344 = ct{860};
t345 = ct{861};
t346 = ct{862};
t348 = ct{863};
t349 = ct{864};
t35 = ct{865};
t350 = ct{866};
t355 = ct{867};
t358 = ct{868};
t359 = ct{869};
t36 = ct{870};
t360 = ct{871};
t363 = ct{872};
t364 = ct{873};
t365 = ct{874};
t366 = ct{875};
t368 = ct{876};
t369 = ct{877};
t370 = ct{878};
t371 = ct{879};
t372 = ct{880};
t373 = ct{881};
t374 = ct{882};
t376 = ct{883};
t377 = ct{884};
t378 = ct{885};
t38 = ct{886};
t381 = ct{887};
t382 = ct{888};
t384 = ct{889};
t385 = ct{890};
t386 = ct{891};
t388 = ct{892};
t389 = ct{893};
t39 = ct{894};
t390 = ct{895};
t391 = ct{896};
t392 = ct{897};
t393 = ct{898};
t396 = ct{899};
t397 = ct{900};
t398 = ct{901};
t403 = ct{902};
t404 = ct{903};
t405 = ct{904};
t406 = ct{905};
t407 = ct{906};
t408 = ct{907};
t410 = ct{908};
t411 = ct{909};
t412 = ct{910};
t413 = ct{911};
t414 = ct{912};
t415 = ct{913};
t419 = ct{914};
t42 = ct{915};
t420 = ct{916};
t421 = ct{917};
t422 = ct{918};
t423 = ct{919};
t424 = ct{920};
t425 = ct{921};
t426 = ct{922};
t427 = ct{923};
t428 = ct{924};
t43 = ct{925};
t430 = ct{926};
t431 = ct{927};
t432 = ct{928};
t433 = ct{929};
t434 = ct{930};
t435 = ct{931};
t437 = ct{932};
t438 = ct{933};
t439 = ct{934};
t44 = ct{935};
t440 = ct{936};
t441 = ct{937};
t442 = ct{938};
t444 = ct{939};
t445 = ct{940};
t446 = ct{941};
t448 = ct{942};
t45 = ct{943};
t451 = ct{944};
t452 = ct{945};
t455 = ct{946};
t456 = ct{947};
t457 = ct{948};
t458 = ct{949};
t459 = ct{950};
t46 = ct{951};
t460 = ct{952};
t461 = ct{953};
t462 = ct{954};
t463 = ct{955};
t464 = ct{956};
t465 = ct{957};
t466 = ct{958};
t467 = ct{959};
t468 = ct{960};
t469 = ct{961};
t47 = ct{962};
t470 = ct{963};
t471 = ct{964};
t472 = ct{965};
t473 = ct{966};
t474 = ct{967};
t475 = ct{968};
t476 = ct{969};
t477 = ct{970};
t478 = ct{971};
t479 = ct{972};
t48 = ct{973};
t480 = ct{974};
t483 = ct{975};
t485 = ct{976};
t486 = ct{977};
t487 = ct{978};
t488 = ct{979};
t489 = ct{980};
t490 = ct{981};
t491 = ct{982};
t492 = ct{983};
t493 = ct{984};
t494 = ct{985};
t495 = ct{986};
t496 = ct{987};
t497 = ct{988};
t498 = ct{989};
t499 = ct{990};
t50 = ct{991};
t500 = ct{992};
t501 = ct{993};
t502 = ct{994};
t503 = ct{995};
t504 = ct{996};
t505 = ct{997};
t506 = ct{998};
t507 = ct{999};
t508 = ct{1000};
t509 = ct{1001};
t51 = ct{1002};
t510 = ct{1003};
t511 = ct{1004};
t514 = ct{1005};
t515 = ct{1006};
t516 = ct{1007};
t519 = ct{1008};
t52 = ct{1009};
t520 = ct{1010};
t521 = ct{1011};
t522 = ct{1012};
t528 = ct{1013};
t53 = ct{1014};
t531 = ct{1015};
t532 = ct{1016};
t533 = ct{1017};
t537 = ct{1018};
t54 = ct{1019};
t545 = ct{1020};
t547 = ct{1021};
t548 = ct{1022};
t550 = ct{1023};
t553 = ct{1024};
t554 = ct{1025};
t555 = ct{1026};
t557 = ct{1027};
t559 = ct{1028};
t56 = ct{1029};
t560 = ct{1030};
t561 = ct{1031};
t562 = ct{1032};
t566 = ct{1033};
t568 = ct{1034};
t57 = ct{1035};
t570 = ct{1036};
t58 = ct{1037};
t582 = ct{1038};
t583 = ct{1039};
t584 = ct{1040};
t585 = ct{1041};
t589 = ct{1042};
t59 = ct{1043};
t590 = ct{1044};
t591 = ct{1045};
t592 = ct{1046};
t595 = ct{1047};
t597 = ct{1048};
t599 = ct{1049};
t60 = ct{1050};
t600 = ct{1051};
t601 = ct{1052};
t605 = ct{1053};
t606 = ct{1054};
t607 = ct{1055};
t608 = ct{1056};
t609 = ct{1057};
t619 = ct{1058};
t620 = ct{1059};
t621 = ct{1060};
t622 = ct{1061};
t628 = ct{1062};
t63 = ct{1063};
t635 = ct{1064};
t636 = ct{1065};
t638 = ct{1066};
t64 = ct{1067};
t640 = ct{1068};
t641 = ct{1069};
t642 = ct{1070};
t643 = ct{1071};
t645 = ct{1072};
t646 = ct{1073};
t648 = ct{1074};
t649 = ct{1075};
t65 = ct{1076};
t654 = ct{1077};
t655 = ct{1078};
t656 = ct{1079};
t657 = ct{1080};
t659 = ct{1081};
t660 = ct{1082};
t663 = ct{1083};
t664 = ct{1084};
t665 = ct{1085};
t666 = ct{1086};
t667 = ct{1087};
t668 = ct{1088};
t669 = ct{1089};
t67 = ct{1090};
t670 = ct{1091};
t672 = ct{1092};
t673 = ct{1093};
t674 = ct{1094};
t675 = ct{1095};
t676 = ct{1096};
t677 = ct{1097};
t678 = ct{1098};
t679 = ct{1099};
t68 = ct{1100};
t681 = ct{1101};
t682 = ct{1102};
t683 = ct{1103};
t684 = ct{1104};
t685 = ct{1105};
t686 = ct{1106};
t687 = ct{1107};
t689 = ct{1108};
t69 = ct{1109};
t691 = ct{1110};
t692 = ct{1111};
t693 = ct{1112};
t694 = ct{1113};
t70 = ct{1114};
t702 = ct{1115};
t704 = ct{1116};
t705 = ct{1117};
t707 = ct{1118};
t708 = ct{1119};
t71 = ct{1120};
t710 = ct{1121};
t711 = ct{1122};
t712 = ct{1123};
t713 = ct{1124};
t714 = ct{1125};
t715 = ct{1126};
t716 = ct{1127};
t717 = ct{1128};
t718 = ct{1129};
t719 = ct{1130};
t72 = ct{1131};
t720 = ct{1132};
t721 = ct{1133};
t722 = ct{1134};
t723 = ct{1135};
t724 = ct{1136};
t725 = ct{1137};
t726 = ct{1138};
t728 = ct{1139};
t73 = ct{1140};
t736 = ct{1141};
t738 = ct{1142};
t740 = ct{1143};
t741 = ct{1144};
t742 = ct{1145};
t743 = ct{1146};
t744 = ct{1147};
t745 = ct{1148};
t746 = ct{1149};
t747 = ct{1150};
t749 = ct{1151};
t75 = ct{1152};
t750 = ct{1153};
t751 = ct{1154};
t755 = ct{1155};
t756 = ct{1156};
t757 = ct{1157};
t758 = ct{1158};
t759 = ct{1159};
t76 = ct{1160};
t762 = ct{1161};
t763 = ct{1162};
t764 = ct{1163};
t766 = ct{1164};
t768 = ct{1165};
t77 = ct{1166};
t770 = ct{1167};
t771 = ct{1168};
t772 = ct{1169};
t773 = ct{1170};
t774 = ct{1171};
t775 = ct{1172};
t776 = ct{1173};
t777 = ct{1174};
t778 = ct{1175};
t78 = ct{1176};
t781 = ct{1177};
t782 = ct{1178};
t783 = ct{1179};
t784 = ct{1180};
t785 = ct{1181};
t786 = ct{1182};
t787 = ct{1183};
t789 = ct{1184};
t79 = ct{1185};
t790 = ct{1186};
t791 = ct{1187};
t792 = ct{1188};
t793 = ct{1189};
t794 = ct{1190};
t796 = ct{1191};
t797 = ct{1192};
t798 = ct{1193};
t799 = ct{1194};
t8 = ct{1195};
t80 = ct{1196};
t800 = ct{1197};
t801 = ct{1198};
t802 = ct{1199};
t806 = ct{1200};
t807 = ct{1201};
t808 = ct{1202};
t809 = ct{1203};
t81 = ct{1204};
t812 = ct{1205};
t813 = ct{1206};
t816 = ct{1207};
t817 = ct{1208};
t818 = ct{1209};
t819 = ct{1210};
t82 = ct{1211};
t820 = ct{1212};
t821 = ct{1213};
t822 = ct{1214};
t823 = ct{1215};
t824 = ct{1216};
t825 = ct{1217};
t826 = ct{1218};
t827 = ct{1219};
t828 = ct{1220};
t829 = ct{1221};
t830 = ct{1222};
t831 = ct{1223};
t832 = ct{1224};
t833 = ct{1225};
t836 = ct{1226};
t837 = ct{1227};
t838 = ct{1228};
t839 = ct{1229};
t84 = ct{1230};
t840 = ct{1231};
t841 = ct{1232};
t844 = ct{1233};
t845 = ct{1234};
t846 = ct{1235};
t85 = ct{1236};
t850 = ct{1237};
t851 = ct{1238};
t852 = ct{1239};
t853 = ct{1240};
t854 = ct{1241};
t855 = ct{1242};
t857 = ct{1243};
t86 = ct{1244};
t860 = ct{1245};
t861 = ct{1246};
t863 = ct{1247};
t864 = ct{1248};
t866 = ct{1249};
t867 = ct{1250};
t869 = ct{1251};
t874 = ct{1252};
t875 = ct{1253};
t876 = ct{1254};
t877 = ct{1255};
t878 = ct{1256};
t882 = ct{1257};
t883 = ct{1258};
t887 = ct{1259};
t889 = ct{1260};
t89 = ct{1261};
t890 = ct{1262};
t896 = ct{1263};
t897 = ct{1264};
t898 = ct{1265};
t9 = ct{1266};
t90 = ct{1267};
t900 = ct{1268};
t901 = ct{1269};
t902 = ct{1270};
t903 = ct{1271};
t904 = ct{1272};
t905 = ct{1273};
t906 = ct{1274};
t908 = ct{1275};
t909 = ct{1276};
t91 = ct{1277};
t913 = ct{1278};
t92 = ct{1279};
t920 = ct{1280};
t921 = ct{1281};
t923 = ct{1282};
t924 = ct{1283};
t929 = ct{1284};
t93 = ct{1285};
t938 = ct{1286};
t939 = ct{1287};
t94 = ct{1288};
t946 = ct{1289};
t95 = ct{1290};
t952 = ct{1291};
t954 = ct{1292};
t956 = ct{1293};
t957 = ct{1294};
t96 = ct{1295};
t963 = ct{1296};
t964 = ct{1297};
t97 = ct{1298};
t972 = ct{1299};
t975 = ct{1300};
t977 = ct{1301};
t98 = ct{1302};
t983 = ct{1303};
t986 = ct{1304};
t988 = ct{1305};
t99 = ct{1306};
t996 = ct{1307};
t998 = ct{1308};
t2625 = t21.*t24.*t25.*t26.*t50.*t202.*1.294536862550567e-20;
t2626 = t18.*t25.*t26.*t50.*t202.*5.999580612847032e-21;
t2627 = t19.*t24.*t26.*t50.*t202.*5.999580612847032e-21;
t2628 = t20.*t24.*t25.*t50.*t202.*5.999580612847032e-21;
t2631 = t24.*t25.*t26.*t27.*t50.*t202.*1.294536862550567e-20;
t2632 = t20.*t24.*t25.*t50.*t202.*(-3.566935413776081e-21);
t2633 = t24.*t25.*t26.*t50.*t202.*5.999580612847032e-21;
t2635 = t24.*t25.*t26.*t50.*t202.*(-3.566935413776081e-21);
t2639 = t18.*t19.*t20.*t50.*t202.*6.715770285417749e-24;
t2640 = t18.*t19.*t26.*t50.*t202.*(-3.992732227073824e-24);
t2641 = t18.*t19.*t26.*t50.*t202.*6.715770285417749e-24;
t2642 = t18.*t20.*t25.*t50.*t202.*6.715770285417749e-24;
t2643 = t19.*t20.*t24.*t50.*t202.*6.715770285417749e-24;
t2645 = t18.*t25.*t26.*t50.*t202.*(-3.992732227073824e-24);
t2646 = t19.*t24.*t26.*t50.*t202.*(-3.992732227073824e-24);
t2647 = t20.*t24.*t25.*t50.*t202.*(-3.992732227073824e-24);
t2651 = t18.*t25.*t26.*t50.*t202.*6.715770285417749e-24;
t2652 = t19.*t24.*t26.*t50.*t202.*6.715770285417749e-24;
t2653 = t20.*t24.*t25.*t50.*t202.*6.715770285417749e-24;
t2656 = t24.*t25.*t26.*t50.*t202.*6.715770285417749e-24;
t2723 = t18.*t19.*t50.*t202.*5.091703513734173e-22;
t2724 = t18.*t25.*t50.*t202.*5.091703513734173e-22;
t2725 = t19.*t24.*t50.*t202.*5.091703513734173e-22;
t2726 = t24.*t25.*t50.*t202.*5.091703513734173e-22;
t2727 = t18.*t19.*t50.*t202.*8.564238525144865e-22;
t2728 = t18.*t25.*t50.*t202.*8.564238525144865e-22;
t2729 = t19.*t24.*t50.*t202.*8.564238525144865e-22;
t2730 = t24.*t25.*t50.*t202.*8.564238525144865e-22;
t2735 = t38.*t50.*t202.*2.682760897261168e-21;
t2736 = t39.*t50.*t202.*2.682760897261168e-21;
t2745 = t18.*t19.*t50.*t202.*2.073708701385059e-20;
t2748 = t18.*t25.*t50.*t202.*2.073708701385059e-20;
t2749 = t19.*t24.*t50.*t202.*2.073708701385059e-20;
t2750 = t24.*t25.*t50.*t202.*2.073708701385059e-20;
t2773 = t38.*t50.*t202.*5.478197787607436e-20;
t2774 = t39.*t50.*t202.*5.478197787607436e-20;
t2775 = t18.*t19.*t50.*t202.*5.17981854669388e-20;
t2777 = t18.*t25.*t50.*t202.*5.17981854669388e-20;
t2778 = t19.*t24.*t50.*t202.*5.17981854669388e-20;
t2779 = t18.*t19.*t50.*t202.*3.079561623286356e-20;
t2780 = t24.*t25.*t50.*t202.*5.17981854669388e-20;
t2781 = t18.*t19.*t50.*t202.*3.487975272406493e-20;
t2782 = t18.*t25.*t50.*t202.*3.079561623286356e-20;
t2783 = t19.*t24.*t50.*t202.*3.079561623286356e-20;
t2785 = t18.*t25.*t50.*t202.*3.487975272406493e-20;
t2786 = t19.*t24.*t50.*t202.*3.487975272406493e-20;
t2787 = t24.*t25.*t50.*t202.*3.079561623286356e-20;
t2788 = t24.*t25.*t50.*t202.*3.487975272406493e-20;
t2797 = t38.*t50.*t202.*3.912111626280478e-20;
t2800 = t39.*t50.*t202.*3.912111626280478e-20;
t2857 = t18.*t19.*t20.*t21.*t50.*t202.*3.933139165631123e-21;
t2858 = t18.*t20.*t21.*t25.*t50.*t202.*3.933139165631123e-21;
t2859 = t19.*t20.*t21.*t24.*t50.*t202.*3.933139165631123e-21;
t2860 = t20.*t21.*t24.*t25.*t50.*t202.*3.933139165631123e-21;
t2865 = t18.*t19.*t26.*t50.*t202.*1.822828392793495e-21;
t2867 = t18.*t25.*t26.*t50.*t202.*1.822828392793495e-21;
t2868 = t19.*t24.*t26.*t50.*t202.*1.822828392793495e-21;
t2872 = t24.*t25.*t26.*t50.*t202.*1.822828392793495e-21;
t2879 = t18.*t19.*t26.*t50.*t202.*3.065994927666357e-21;
t2883 = t18.*t25.*t26.*t50.*t202.*3.065994927666357e-21;
t2884 = t19.*t24.*t26.*t50.*t202.*3.065994927666357e-21;
t2886 = t24.*t25.*t26.*t50.*t202.*3.065994927666357e-21;
t2887 = t18.*t19.*t20.*t27.*t50.*t202.*1.793448789769173e-21;
t2890 = t18.*t19.*t20.*t50.*t202.*2.040425413990593e-24;
t2891 = t18.*t20.*t25.*t27.*t50.*t202.*1.793448789769173e-21;
t2892 = t19.*t20.*t24.*t27.*t50.*t202.*1.793448789769173e-21;
t2894 = t18.*t20.*t25.*t50.*t202.*2.040425413990593e-24;
t2895 = t19.*t20.*t24.*t50.*t202.*2.040425413990593e-24;
t2896 = t18.*t19.*t20.*t21.*t50.*t202.*6.615534835481934e-21;
t2898 = t20.*t24.*t25.*t27.*t50.*t202.*1.793448789769173e-21;
t2899 = t20.*t24.*t25.*t50.*t202.*2.040425413990593e-24;
t2900 = t18.*t20.*t21.*t25.*t50.*t202.*6.615534835481934e-21;
t2901 = t19.*t20.*t21.*t24.*t50.*t202.*6.615534835481934e-21;
t2903 = t20.*t21.*t24.*t25.*t50.*t202.*6.615534835481934e-21;
t2905 = t18.*t19.*t20.*t27.*t50.*t202.*3.016578474529275e-21;
t2906 = t18.*t20.*t25.*t27.*t50.*t202.*3.016578474529275e-21;
t2907 = t19.*t20.*t24.*t27.*t50.*t202.*3.016578474529275e-21;
t2908 = t20.*t24.*t25.*t27.*t50.*t202.*3.016578474529275e-21;
t2915 = t18.*t19.*t20.*t50.*t202.*3.431992827360689e-24;
t2917 = t18.*t20.*t25.*t50.*t202.*3.431992827360689e-24;
t2918 = t19.*t20.*t24.*t50.*t202.*3.431992827360689e-24;
t2919 = t20.*t24.*t25.*t50.*t202.*3.431992827360689e-24;
t2959 = t50.*t188.*t202.*2.657710136023448e-22;
t2960 = t50.*t189.*t201.*2.657710136023448e-22;
t2965 = t50.*t188.*t202.*7.819782623635085e-24;
t2966 = t50.*t189.*t201.*7.819782623635085e-24;
t2967 = t50.*t188.*t202.*2.551073618220038e-22;
t2968 = t50.*t189.*t201.*2.551073618220038e-22;
t49 = -t46;
t131 = t43+t44;
t140 = t45+t48;
t268 = -t252;
t291 = t265.^2;
t292 = t250-1.0;
t335 = t237./1.0e+8;
t336 = t238./1.0e+8;
t337 = -t325;
t351 = -t340;
t352 = -t342;
t354 = -t344;
t356 = -t345;
t361 = -t348;
t362 = -t350;
t380 = -t366;
t387 = -t374;
t429 = t72+t86;
t512 = t237.*5.110348748545983e-1;
t513 = t238.*5.110348748545983e-1;
t517 = t262.*5.110348748545983e-1;
t518 = t264.*5.110348748545983e-1;
t523 = t237.*5.84482e-3;
t524 = t238.*5.84482e-3;
t525 = t237.*9.840000000000001e-6;
t526 = t238.*9.840000000000001e-6;
t527 = t240.*3.064357668490995e+34;
t530 = t237.*6.48e-5;
t536 = t238.*6.48e-5;
t538 = t11.*t237.*1.247162e-2;
t539 = t11.*t238.*1.247162e-2;
t540 = t16.*t238.*1.247162e-2;
t542 = t262.*5.84482e-3;
t543 = t264.*5.84482e-3;
t544 = t53.*t240;
t546 = t54.*t240;
t551 = t16.*t237.*5.68686e-3;
t552 = t11.*t238.*5.68686e-3;
t556 = t16.*t238.*5.68686e-3;
t563 = t262.*6.48e-5;
t565 = t264.*6.48e-5;
t569 = t237.*3.24e-6;
t571 = t237.*5.78002e-3;
t572 = t238.*3.24e-6;
t573 = t238.*5.78002e-3;
t574 = t237.*7.83e-6;
t575 = t237.*6.47e-6;
t576 = t238.*7.83e-6;
t577 = t238.*6.47e-6;
t578 = t237.*6.2e-7;
t580 = t238.*6.2e-7;
t610 = t262.*6.47e-6;
t611 = t264.*6.47e-6;
t612 = t237.*5.110348748545983e-9;
t613 = t98.*t240;
t614 = t99.*t240;
t615 = t100.*t240;
t616 = t101.*t240;
t617 = t102.*t240;
t618 = t103.*t240;
t623 = t107.*t240;
t624 = t108.*t240;
t625 = t109.*t240;
t627 = t110.*t240;
t629 = t111.*t240;
t630 = t112.*t240;
t631 = t113.*t240;
t634 = t114.*t240;
t637 = t117.*t240;
t650 = t20.*t22.*t240.*-3.315051378778914e+33;
t651 = t20.*t27.*t240.*7.788445287802242e+33;
t652 = t21.*t26.*t240.*-1.990083581481952e+33;
t658 = t21.*t28.*t240.*-1.025883768304404e+34;
t662 = t26.*t28.*t240.*-6.099194893302011e+33;
t696 = t128.*t240;
t697 = t129.*t240;
t698 = t130.*t240;
t701 = t132.*t240;
t733 = t134.*t240;
t734 = t135.*t240;
t735 = t136.*t240;
t737 = t137.*t240;
t739 = t21.*t26.*t28.*t240.*-3.315051378778914e+33;
t765 = t21.*t22.*t26.*t240.*-6.099194893302011e+33;
t767 = t139.*t240;
t847 = t146.*t240;
t849 = t147.*t240;
t856 = t20.*t240.*-7.746286054220548e+49;
t858 = t26.*t240.*-7.746286054220548e+49;
t859 = -t850;
t865 = -t855;
t868 = t160.*t240;
t870 = t161.*t240;
t871 = t162.*t240;
t872 = t10.*t850;
t873 = t15.*t850;
t881 = t167.*t240;
t884 = t169.*t240;
t885 = t172.*t240;
t886 = t163.*t240;
t888 = t164.*t240;
t891 = t20.*t855;
t892 = t26.*t855;
t893 = t26.*t240.*-6.997781708721691e+52;
t894 = t20.*t27.*t240.*-7.290917220067534e+49;
t895 = t26.*t27.*t240.*-7.290917220067534e+49;
t907 = t20.*t27.*t240.*7.342112502577776e+52;
t911 = t203.*t240;
t912 = t204.*t240;
t914 = t205.*t240;
t915 = t208.*t240;
t916 = t195.*t240;
t917 = t196.*t240;
t918 = t197.*t240;
t926 = t216.*t240;
t927 = t217.*t240;
t928 = t220.*t240;
t930 = t223.*t240;
t931 = t224.*t240;
t932 = t225.*t240;
t933 = t226.*t240;
t934 = t227.*t240;
t935 = t20.*t21.*t22.*t240.*-5.84291401185902e+49;
t936 = t230.*t240;
t937 = t231.*t240;
t940 = t26.*t28.*t240.*-2.201616617347892e+53;
t942 = t21.*t50.*t240.*7.432538878058787e+17i;
t943 = t20.*t22.*t240.*-1.196628789628727e+53;
t944 = (t123.*t237)./9.007199254740992e+15;
t945 = (t123.*t238)./9.007199254740992e+15;
t947 = t201+t258;
t948 = t188+t252-1.0;
t950 = t237.*(t42-t43).*(-1.110223024625157e-16);
t951 = t238.*(t42-t43).*(-1.110223024625157e-16);
t959 = t240.*t259;
t960 = t240.*t260;
t961 = t240.*t261;
t962 = t240.*t263;
t965 = t26.*t27.*t50.*t240.*4.418873226179514e+17i;
t966 = t240.*t271;
t967 = t240.*t272;
t968 = t240.*t273;
t969 = t240.*t274;
t970 = t240.*t255;
t971 = t240.*t256;
t973 = t240.*t257;
t974 = (t238.*(t42-t43))./9.007199254740992e+15;
t976 = t16.*t938;
t978 = t240.*t277;
t979 = t240.*t279;
t980 = t240.*t280;
t981 = t240.*t281;
t982 = t240.*t283;
t984 = t240.*t286;
t985 = t20.*t21.*t50.*t240.*-4.323455642275676e+17i;
t987 = t240.*t276;
t989 = -t972;
t990 = t26.*t27.*t50.*t240.*-4.323455642275676e+17i;
t992 = t20.*t28.*t50.*t240.*-1.325049802940888e+18i;
t993 = t22.*t26.*t50.*t240.*-1.325049802940888e+18i;
t994 = t26.*t28.*t50.*t240.*-1.325049802940888e+18i;
t995 = t26.*t28.*t50.*t240.*-7.201947557068188e+17i;
t997 = t238.*5.028583168569248e-6;
t999 = t244+t258+1.0;
t1007 = t240.*t301;
t1009 = t240.*t302;
t1010 = t240.*t303;
t1011 = t240.*t304;
t1012 = t240.*t305;
t1013 = t240.*t306;
t1014 = t240.*t307;
t1015 = t237.*2.986906857247653e-3;
t1016 = t240.*t308;
t1017 = t238.*2.986906857247653e-3;
t1018 = -t1002;
t1020 = t237.*3.311505989057797e-5;
t1021 = t238.*3.311505989057797e-5;
t1023 = t262.*(t46-t47).*(-1.110223024625157e-16);
t1024 = t16.*t237.*2.906183788415621e-3;
t1025 = t11.*t238.*2.906183788415621e-3;
t1027 = t264.*(t46-t47).*(-1.110223024625157e-16);
t1028 = t16.*t238.*2.906183788415621e-3;
t1029 = t20.*t21.*t22.*t50.*t240.*-1.325049802940888e+18i;
t1031 = -t1008;
t1032 = t20.*t21.*t28.*t50.*t240.*-7.201947557068188e+17i;
t1038 = t11.*t237.*6.373432765934105e-3;
t1041 = t11.*t238.*6.373432765934105e-3;
t1042 = t16.*t238.*6.373432765934105e-3;
t1045 = (t264.*(t46-t47))./9.007199254740992e+15;
t1046 = t262.*2.986906857247653e-3;
t1048 = t237.*3.168416224098509e-7;
t1050 = -t1035;
t1051 = t262.*3.311505989057797e-5;
t1052 = t237.*4.001403070111505e-6;
t1056 = t238.*2.953791797357075e-3;
t1057 = t237.*3.306395640309251e-6;
t1059 = t238.*3.306395640309251e-6;
t1061 = -t1047;
t1062 = t237.*1.655752994528898e-6;
t1072 = t264.*3.306395640309251e-6;
t1073 = t8.*t9.*t11.*t238.*1.07201054193752e-2;
t1074 = t8.*t11.*t14.*t238.*1.07201054193752e-2;
t1075 = t9.*t11.*t13.*t238.*1.07201054193752e-2;
t1076 = t11.*t13.*t14.*t238.*1.07201054193752e-2;
t1090 = t8.*t14.*t16.*t238.*4.888197259476159e-3;
t1091 = t9.*t13.*t16.*t238.*4.888197259476159e-3;
t1094 = t22.*t26.*t240.*1.297387533374166e+34;
t1095 = t13.*t14.*t16.*t238.*4.888197259476159e-3;
t1098 = t21.*t262.*1.35652563578e-4;
t1099 = t21.*t264.*1.35652563578e-4;
t1100 = t27.*t264.*1.35652563578e-4;
t1102 = t8.*t9.*t237.*2.953791797357075e-3;
t1103 = t26.*t28.*t240.*2.386997519508773e+34;
t1106 = t8.*t14.*t237.*2.953791797357075e-3;
t1107 = t9.*t13.*t237.*2.953791797357075e-3;
t1109 = t11.*t13.*t14.*t238.*(-6.373432765934105e-3);
t1111 = t13.*t14.*t237.*2.953791797357075e-3;
t1116 = t8.*t9.*t16.*t238.*(-2.906183788415621e-3);
t1117 = t27.*t262.*6.1855407534e-5;
t1118 = t21.*t264.*6.1855407534e-5;
t1119 = t8.*t14.*t16.*t238.*(-2.906183788415621e-3);
t1120 = t9.*t13.*t16.*t238.*(-2.906183788415621e-3);
t1122 = t27.*t264.*6.1855407534e-5;
t1125 = t8.*t9.*t16.*t238.*4.888197259476159e-3;
t1129 = t262.*7.0373543e-8;
t1132 = t8.*t9.*t238.*5.561353061058431e-6;
t1135 = t264.*7.0373543e-8;
t1138 = t8.*t14.*t238.*5.561353061058431e-6;
t1139 = t9.*t13.*t238.*5.561353061058431e-6;
t1140 = t13.*t14.*t238.*5.561353061058431e-6;
t1141 = t262.*6.2868699538e-5;
t1142 = t264.*6.2868699538e-5;
t1144 = t8.*t9.*t237.*4.968273867075572e-3;
t1146 = t8.*t14.*t237.*4.968273867075572e-3;
t1147 = t9.*t13.*t237.*4.968273867075572e-3;
t1149 = t13.*t14.*t237.*4.968273867075572e-3;
t1165 = t13.*t14.*t238.*(-3.306395640309251e-6);
t1171 = t240.*t373;
t1174 = t240.*t376;
t1186 = t20.*t27.*t28.*t240.*1.297387533374166e+34;
t1187 = t21.*t50.*t240.*-1.746965228796509e+32i;
t1188 = t20.*t22.*t27.*t240.*2.386997519508773e+34;
t1191 = t240.*t381;
t1195 = t240.*t384;
t1206 = t240.*t397;
t1209 = t240.*t398;
t1213 = t20.*t50.*t240.*-4.394953650240249e+33i;
t1224 = t240.*t405;
t1226 = t240.*t411;
t1228 = t240.*t412;
t1239 = t240.*t421;
t1240 = t240.*t422;
t1241 = t240.*t423;
t1244 = t240.*t428;
t1245 = t21.*t26.*t50.*t240.*-1.03862462117543e+32i;
t1250 = t240.*t430;
t1251 = t26.*t27.*t50.*t240.*-1.03862462117543e+32i;
t1257 = t240.*t437;
t1258 = t240.*t438;
t1259 = t240.*t439;
t1260 = t240.*t441;
t1261 = t240.*t442;
t1262 = t20.*t27.*t50.*t240.*-4.136594366080324e+33i;
t1263 = t21.*t26.*t50.*t240.*-4.136594366080324e+33i;
t1264 = t240.*t444;
t1266 = t20.*t50.*t240.*-3.97028021545552e+36i;
t1268 = t26.*t50.*t240.*-3.97028021545552e+36i;
t1270 = t21.*t22.*t50.*t240.*-1.025883768304404e+34i;
t1271 = t21.*t28.*t50.*t240.*-5.575912001630188e+33i;
t1272 = t22.*t27.*t50.*t240.*-5.575912001630188e+33i;
t1281 = -t1269;
t1282 = t240.*t466;
t1283 = t240.*t469;
t1296 = t16.*t1265;
t1304 = t240.*t470;
t1310 = t240.*t460;
t1314 = t240.*t461;
t1325 = t240.*t462;
t1326 = t240.*t463;
t1330 = t21.*t26.*t28.*t50.*t240.*-3.315051378778914e+33i;
t1331 = t26.*t27.*t50.*t240.*1.595073594941899e+37i;
t1332 = t26.*t27.*t28.*t50.*t240.*-3.315051378778914e+33i;
t1353 = t240.*t487;
t1359 = t240.*t488;
t1364 = t240.*t489;
t1365 = t240.*t490;
t1372 = t26.*t240.*7.152220999552773e+52;
t1377 = t240.*t492;
t1381 = t240.*t473;
t1382 = t240.*t474;
t1383 = t240.*t475;
t1388 = t26.*t27.*t50.*t240.*-4.075691174875038e+36i;
t1390 = t240.*t479;
t1391 = t240.*t480;
t1401 = -t1327;
t1402 = -t1329;
t1403 = t324+t349;
t1418 = t21.*t22.*t26.*t50.*t240.*-6.099194893302011e+33i;
t1422 = t21.*t26.*t28.*t50.*t240.*-6.099194893302011e+33i;
t1423 = t22.*t26.*t27.*t50.*t240.*-6.099194893302011e+33i;
t1426 = -t1373;
t1431 = t20.*t28.*t50.*t240.*-1.249115114148252e+37i;
t1432 = t22.*t26.*t50.*t240.*-1.249115114148252e+37i;
t1437 = t26.*t28.*t50.*t240.*-1.249115114148252e+37i;
t1439 = t26.*t28.*t50.*t240.*-6.789225223739216e+36i;
t1444 = t27.*t240.*3.147052781374869e+48;
t1449 = t240.*t503;
t1450 = t240.*t504;
t1451 = t240.*t505;
t1452 = t240.*t506;
t1453 = t26.*t28.*t240.*2.250205745048369e+53;
t1457 = t20.*t240.*7.917244648613035e+49;
t1459 = t22.*t26.*t240.*1.223038087510652e+53;
t1460 = t240.*t499;
t1461 = t240.*t500;
t1462 = t21.*t240.*1.253396129822139e+50;
t1463 = t240.*t501;
t1464 = t240.*t502;
t1468 = t21.*t26.*t240.*1.871019782761396e+48;
t1469 = -t1455;
t1471 = -t1456;
t1479 = -t1470;
t1482 = -t1473;
t1484 = -t1475;
t1485 = -t1477;
t1486 = t20.*t22.*t27.*t240.*2.250205745048369e+53;
t1487 = t27.*t28.*t240.*1.004467008511696e+50;
t1489 = t26.*t27.*t240.*7.451825938264896e+49;
t1494 = -t1481;
t1495 = t22.*t27.*t240.*1.848067902664462e+50;
t1499 = t20.*t27.*t28.*t240.*1.223038087510652e+53;
t1504 = -t1488;
t1505 = -t1493;
t1506 = -t1496;
t1507 = -t1498;
t1510 = t50.*t240.*6.804240878490729e+18i;
t1512 = -t1501;
t1516 = -t1503;
t1522 = -t1511;
t1525 = t21.*t22.*t26.*t240.*1.098733273949399e+50;
t1526 = -t1513;
t1527 = -t1515;
t1529 = -t1519;
t1531 = -t1521;
t1532 = t21.*t26.*t28.*t240.*5.971865661673106e+49;
t1533 = -t1524;
t1535 = t57+t58+t59+t95;
t1536 = t56+t73+t410;
t1543 = -t1537;
t1544 = t123.*t238.*6.489053738789607e-19;
t1547 = t123.*t238.*7.194245199571015e-21;
t1549 = t238.*(t42-t43).*(-6.489053738789607e-19);
t1550 = -t1545;
t1551 = t20.*t28.*t50.*t240.*1.354293320444013e+18i;
t1552 = t20.*t22.*t50.*t240.*7.360892737071442e+17i;
t1554 = t238.*(t42-t43).*(-7.194245199571015e-21);
t1555 = t21.*t22.*t50.*t240.*2.277919560321538e+18i;
t1556 = t21.*t28.*t50.*t240.*1.238101177498716e+18i;
t1558 = t238.*(t42-t43).*7.194245199571015e-21;
t1559 = t123.*t237.*7.183142969324763e-22;
t1565 = t237.*(t42-t43).*(-7.183142969324763e-22);
t1568 = -t1561;
t1569 = -t1562;
t1572 = -t1563;
t1574 = t22.*t26.*t27.*t50.*t240.*1.354293320444013e+18i;
t1575 = t26.*t27.*t28.*t50.*t240.*7.360892737071442e+17i;
t1579 = -t1566;
t1583 = -t1573;
t1588 = t16.*t237.*5.68686e-3;
t1592 = t11.*t237.*1.247162e-2;
t1594 = t238.*6.48e-5;
t1595 = -t1577;
t1596 = -t1578;
t1599 = t264.*(t46-t47).*(-6.489053738789607e-19);
t1600 = -t1581;
t1601 = -t1586;
t1602 = -t1587;
t1604 = -t1589;
t1605 = -t1590;
t1606 = -t1591;
t1613 = t264.*(t46-t47).*(-7.194245199571015e-21);
t1618 = t262.*3.601891949238275e-7;
t1619 = t264.*3.601891949238275e-7;
t1620 = t262.*8.631097478604537e-5;
t1622 = t264.*8.631097478604537e-5;
t1626 = -t1608;
t1627 = -t1609;
t1628 = -t1611;
t1629 = t13.*t14.*t238.*1.509490621508912e-3;
t1631 = -t1617;
t1633 = t8.*t9.*t11.*t237.*2.498039274760989e-3;
t1634 = t8.*t9.*t16.*t237.*2.498039274760989e-3;
t1635 = t8.*t11.*t14.*t237.*2.498039274760989e-3;
t1636 = t9.*t11.*t13.*t237.*2.498039274760989e-3;
t1637 = t8.*t9.*t11.*t237.*3.257046415933332e-3;
t1639 = t8.*t9.*t16.*t238.*2.498039274760989e-3;
t1640 = t8.*t14.*t16.*t237.*2.498039274760989e-3;
t1641 = t9.*t13.*t16.*t237.*2.498039274760989e-3;
t1642 = t11.*t13.*t14.*t237.*2.498039274760989e-3;
t1643 = t8.*t9.*t16.*t237.*3.257046415933332e-3;
t1644 = t8.*t9.*t11.*t238.*3.257046415933332e-3;
t1645 = t8.*t11.*t14.*t237.*3.257046415933332e-3;
t1646 = t9.*t11.*t13.*t237.*3.257046415933332e-3;
t1650 = t8.*t9.*t11.*t237.*1.485161268617439e-3;
t1651 = t8.*t9.*t11.*t237.*5.478347731418506e-3;
t1652 = t8.*t14.*t16.*t238.*2.498039274760989e-3;
t1653 = t9.*t13.*t16.*t238.*2.498039274760989e-3;
t1654 = t13.*t14.*t16.*t237.*2.498039274760989e-3;
t1655 = t8.*t14.*t16.*t237.*3.257046415933332e-3;
t1656 = t8.*t11.*t14.*t238.*3.257046415933332e-3;
t1657 = t9.*t13.*t16.*t237.*3.257046415933332e-3;
t1658 = t9.*t11.*t13.*t238.*3.257046415933332e-3;
